simulink model "deltino"  (R2021b)
settings: Solver=VariableStepAuto  StartTime=0.0  StopTime=inf  FixedStep=0.0001  RelTol=1e-3
values from neighbouring files (symbols this model uses):
  alpha1 = 0    [compute_deltino_dyn_parallel.m]
  alpha2 = 2/3*pi    (= 2.09439510239)    [compute_deltino_dyn_parallel.m]
  alpha3 = 4/3*pi    (= 4.18879020479)    [compute_deltino_dyn_parallel.m]
  H = 0.05    [main.m]
  J_T = [J_1', J_2', J_3', J_4']    [main.m]
  K_d = 10    [main.m]
  K_el = 10000    [main.m]
  K_i = 1    [main.m]
  K_p = 200    [main.m]
  K_v = 10    [main.m]
  mu = 0.8    [main.m]
  ni_0 = zeros(18,1)    [main.m]
  offset1 = [l1/2; l2/2; -h/2]    [compute_deltino_dyn_parallel.m]    (also in main.m = [+l1/2; +l2/2; -h/2])
  offset2 = [l1/2; -l2/2; -h/2]    [compute_deltino_dyn_parallel.m]    (also in main.m = [+l1/2; -l2/2; -h/2])
  offset3 = [-l1/2; -l2/2; -h/2]    [compute_deltino_dyn_parallel.m]    (also in main.m)
  offset4 = [-l1/2; l2/2; -h/2]    [compute_deltino_dyn_parallel.m]    (also in main.m = [-l1/2; +l2/2; -h/2])
  p_leg1_0 = forward_kin(theta_leg1_0)    [main.m]
  p_leg2_0 = forward_kin(theta_leg2_0)    [main.m]
  p_leg3_0 = forward_kin(theta_leg3_0)    [main.m]
  p_leg4_0 = forward_kin(theta_leg4_0)    [main.m]
  points_ccw = [+0.1,  0.00 ... (first row only)    [main.m]
  points_cw = [-0.1,  0.00 ... (first row only)    [main.m]
  q_0 = [base_0; ypr_0; theta_leg1_0; ee_leg1_0; theta_leg2_0; ee_leg2_0;        theta_leg3_0; ee_leg3_0; theta_leg4_0; ee_leg4_0;]    [main.m]
  ratio = 2    [main.m]
  steps = 4+2*ratio    (= 8)    [main.m]
  theta_leg1_0 = [pi/6; pi/6; pi/6]    [main.m]
  theta_leg2_0 = [pi/6; pi/6; pi/6]    [main.m]
  theta_leg3_0 = [pi/6; pi/6; pi/6]    [main.m]
  theta_leg4_0 = [pi/6; pi/6; pi/6]    [main.m]
  ts = T/steps    (= 0.1875)    [main.m]
  ts2 = 3*ts    (= 0.5625)    [main.m]
  vel = 0.2    [main.m]
undefined symbols (not defined in the file or in its folder): l1, l_A, l_B, R, radius0, radius1, radius2, theta, WPs
libraries: simulink x14, dspsigops x12
(part 3 of 10)

== matlab function deltino/DELTINO DYNAMICS /compute_S_dot ==
  data: q input; S_dot output; q_dot input
function S_dot = S_dot(q, q_dot)
%#codegen

%    This function was generated by the Symbolic Math Toolbox version 9.0.
%    03-May-2022 13:43:05
bx = q(1); by = q(2); bz = q(3);
phi = q(4); zeta = q(5); psi = q(6);
th11 = q(7); th12 = q(8); th13 = q(9);
p1x = q(10); p1y = q(11); p1z = q(12);
th21 = q(13); th22 = q(14); th23 = q(15);
p2x = q(16); p2y = q(17); p2z = q(18);
th31 = q(19); th32 = q(20); th33 = q(21);
p3x = q(22); p3y = q(23); p3z = q(24);
th41 = q(25); th42 = q(26); th43 = q(27);
p4x = q(28); p4y = q(29); p4z = q(30);

bx_dot = q_dot(1); by_dot = q_dot(2); bz_dot = q(3);
phi_dot = q_dot(4); zeta_dot = q_dot(5); psi_dot = q(6);
th11_dot = q_dot(7); th12_dot = q_dot(8); th13_dot = q_dot(9);
p1x_dot = q_dot(10); p1y_dot = q_dot(11); p1z_dot = q_dot(12);
th21_dot = q_dot(13); th22_dot = q_dot(14); th23_dot = q_dot(15);
p2x_dot = q_dot(16); p2y_dot = q_dot(17); p2z_dot = q_dot(18);
th31_dot = q_dot(19); th32_dot = q_dot(20); th33_dot = q_dot(21);
p3x_dot = q_dot(22); p3y_dot = q_dot(23); p3z_dot = q_dot(24);
th41_dot = q_dot(25); th42_dot = q_dot(26); th43_dot = q_dot(27);
p4x_dot = q_dot(28); p4y_dot = q_dot(29); p4z_dot = q_dot(30);

t2 = cos(phi);
t3 = cos(psi);
t4 = cos(th11);
t5 = cos(th12);
t6 = cos(th13);
t7 = cos(th21);
t8 = cos(th22);
t9 = cos(th23);
t10 = cos(th31);
t11 = cos(th32);
t12 = cos(th33);
t13 = cos(th41);
t14 = cos(th42);
t15 = cos(th43);
t16 = cos(zeta);
t17 = sin(phi);
t18 = sin(psi);
t19 = sin(th11);
t20 = sin(th12);
t21 = sin(th13);
t22 = sin(th21);
t23 = sin(th22);
t24 = sin(th23);
t25 = sin(th31);
t26 = sin(th32);
t27 = sin(th33);
t28 = sin(th41);
t29 = sin(th42);
t30 = sin(th43);
t31 = sin(zeta);
t45 = -bx;
t46 = bx.*2.0e+1;
t47 = -bx_dot;
t48 = -by;
t49 = by.*2.0e+1;
t50 = -by_dot;
t51 = -bz;
t52 = bz.*2.0e+1;
t53 = p1x.*2.0e+1;
t54 = p2x.*2.0e+1;
t55 = p3x.*2.0e+1;
t56 = p4x.*2.0e+1;
t57 = -p1y;
t58 = -p2y;
t59 = -p4y;
t60 = p1y.*2.0e+1;
t61 = p2y.*2.0e+1;
t62 = p3y.*2.0e+1;
t63 = p4y.*2.0e+1;
t64 = -p3x_dot;
t65 = -p4x_dot;
t66 = -p4z;
t67 = p1z.*2.0e+1;
t68 = p2z.*2.0e+1;
t69 = p3z.*2.0e+1;
t70 = p4z.*2.0e+1;
t71 = -p1y_dot;
t72 = -p4y_dot;
t73 = -p1z_dot;
t74 = -p2z_dot;
t75 = -p3z_dot;
t76 = -p4z_dot;
t102 = sqrt(3.0);
t32 = t3.*7.0;
t33 = t5.*2.0;
t34 = t6.*2.0;
t35 = t8.*2.0;
t36 = t9.*2.0;
t37 = t11.*2.0;
t38 = t12.*2.0;
t39 = t14.*2.0;
t40 = t15.*2.0;
t41 = t18.*2.0;
t42 = t31.*5.0;
t43 = t31.*6.0;
t44 = t31.*7.0;
t77 = t2.*t3;
t78 = t2.*t16;
t79 = t2.*t18;
t80 = t3.*t17;
t81 = t16.*t17;
t82 = t17.*t18;
t84 = t19.*t31;
t85 = t20.*t31;
t86 = t21.*t31;
t87 = t22.*t31;
t88 = t23.*t31;
t89 = t24.*t31;
t90 = t25.*t31;
t91 = t26.*t31;
t92 = t27.*t31;
t93 = t28.*t31;
t94 = t29.*t31;
t95 = t30.*t31;
t100 = t31.*8.0;
t101 = t31.*9.0;
t103 = -t46;
t104 = -t49;
t105 = -t52;
t106 = -t60;
t107 = -t61;
t108 = -t63;
t109 = -t70;
t113 = t3.*t16.*2.0;
t118 = t16.*t18.*7.0;
t120 = t4.*t31.*4.0;
t123 = t7.*t31.*4.0;
t126 = t10.*t31.*4.0;
t129 = t13.*t31.*4.0;
t132 = t18.*t19.*4.0;
t133 = t18.*t20.*4.0;
t134 = t18.*t21.*4.0;
t135 = t18.*t22.*4.0;
t136 = t18.*t23.*4.0;
t137 = t18.*t24.*4.0;
t138 = t18.*t25.*4.0;
t139 = t18.*t26.*4.0;
t140 = t18.*t27.*4.0;
t141 = t18.*t28.*4.0;
t142 = t18.*t29.*4.0;
t143 = t18.*t30.*4.0;
t144 = t4./5.0;
t145 = t5./5.0;
t146 = t6./5.0;
t147 = t7./5.0;
t148 = t8./5.0;
t149 = t9./5.0;
t150 = t10./5.0;
t151 = t11./5.0;
t152 = t12./5.0;
t153 = t13./5.0;
t154 = t14./5.0;
t155 = t15./5.0;
t156 = t16./2.0;
t157 = t16./4.0;
t158 = t31./2.0;
t159 = t31./4.0;
t195 = t6.*t31.*-2.0;
t196 = t8.*t31.*-2.0;
t197 = t9.*t31.*-2.0;
t198 = t12.*t31.*-2.0;
t199 = t15.*t31.*-2.0;
t202 = t16.*(7.0./2.0e+1);
t204 = t31.*(7.0./2.0e+1);
t209 = t3.*t4.*t16;
t210 = t3.*t7.*t16;
t211 = t3.*t10.*t16;
t212 = t3.*t13.*t16;
t251 = t16.*(9.0./2.0e+1);
t253 = t31.*(9.0./2.0e+1);
t270 = t3.*t102;
t272 = t31.*zeta_dot.*(-1.0./2.0);
t291 = t3.*t16.*t19.*4.0;
t292 = t3.*t16.*t20.*4.0;
t293 = t3.*t16.*t21.*4.0;
t294 = t3.*t16.*t22.*4.0;
t295 = t3.*t16.*t23.*4.0;
t296 = t3.*t16.*t24.*4.0;
t297 = t3.*t16.*t25.*4.0;
t298 = t3.*t16.*t26.*4.0;
t299 = t3.*t16.*t27.*4.0;
t300 = t3.*t16.*t28.*4.0;
t301 = t3.*t16.*t29.*4.0;
t302 = t3.*t16.*t30.*4.0;
t314 = (t3.*t16)./1.0e+1;
t316 = t7.*t16.*(-1.0./5.0);
t317 = t10.*t16.*(-1.0./5.0);
t318 = t13.*t16.*(-1.0./5.0);
t326 = (t3.*t31)./1.0e+1;
t360 = (t16.*t19.*zeta_dot)./5.0;
t361 = (t16.*t22.*zeta_dot)./5.0;
t362 = (t16.*t25.*zeta_dot)./5.0;
t363 = (t16.*t28.*zeta_dot)./5.0;
t372 = t16.*zeta_dot.*(-7.0./2.0e+1);
t374 = t31.*zeta_dot.*(-7.0./2.0e+1);
t433 = t16.*t18.*(-7.0./2.0e+1);
t435 = t18.*t31.*(-7.0./2.0e+1);
t447 = t16.*t18.*t102;
t466 = t4.*t16.*zeta_dot.*(-1.0./5.0);
t473 = (psi_dot.*t16.*t18)./1.0e+1;
t481 = t2.*t31.*zeta_dot.*(-1.0./4.0);
t487 = phi_dot.*t17.*t31.*(-1.0./2.0);
t488 = phi_dot.*t17.*t31.*(-1.0./4.0);
t490 = (psi_dot.*t18.*t31)./1.0e+1;
t492 = t17.*t31.*zeta_dot.*(-1.0./4.0);
t494 = (t18.*t31.*zeta_dot)./1.0e+1;
t496 = t16.*zeta_dot.*(-9.0./2.0e+1);
t537 = (t3.*t16.*t19)./5.0;
t538 = (t3.*t16.*t20)./5.0;
t539 = (t3.*t16.*t21)./5.0;
t540 = (t3.*t16.*t22)./5.0;
t541 = (t3.*t16.*t23)./5.0;
t542 = (t3.*t16.*t24)./5.0;
t543 = (t3.*t16.*t25)./5.0;
t544 = (t3.*t16.*t26)./5.0;
t545 = (t3.*t16.*t27)./5.0;
t546 = (t3.*t16.*t28)./5.0;
t547 = (t3.*t16.*t29)./5.0;
t548 = (t3.*t16.*t30)./5.0;
t706 = (psi_dot.*t16.*t18.*t19)./5.0;
t707 = (psi_dot.*t16.*t18.*t20)./5.0;
t708 = (psi_dot.*t16.*t18.*t21)./5.0;
t709 = (psi_dot.*t16.*t18.*t22)./5.0;
t710 = (psi_dot.*t16.*t18.*t23)./5.0;
t711 = (psi_dot.*t16.*t18.*t24)./5.0;
t712 = (psi_dot.*t16.*t18.*t25)./5.0;
t713 = (psi_dot.*t16.*t18.*t26)./5.0;
t714 = (psi_dot.*t16.*t18.*t27)./5.0;
t715 = (psi_dot.*t16.*t18.*t28)./5.0;
t716 = (psi_dot.*t16.*t18.*t29)./5.0;
t717 = (psi_dot.*t16.*t18.*t30)./5.0;
t728 = psi_dot.*t3.*t16.*(-1.0./1.0e+1);
t729 = psi_dot.*t3.*t16.*(-7.0./2.0e+1);
t765 = t3.*t16.*zeta_dot.*(-1.0./1.0e+1);
t766 = phi_dot.*t2.*t31.*(-7.0./2.0e+1);
t770 = psi_dot.*t3.*t31.*(-7.0./2.0e+1);
t797 = phi_dot.*t17.*t31.*(-7.0./2.0e+1);
t857 = t3.*t5.*t16.*th12_dot.*(-1.0./5.0);
t858 = t3.*t6.*t16.*th13_dot.*(-1.0./5.0);
t860 = t3.*t8.*t16.*th22_dot.*(-1.0./5.0);
t861 = t3.*t9.*t16.*th23_dot.*(-1.0./5.0);
t863 = t3.*t11.*t16.*th32_dot.*(-1.0./5.0);
t864 = t3.*t12.*t16.*th33_dot.*(-1.0./5.0);
t866 = t3.*t14.*t16.*th42_dot.*(-1.0./5.0);
t867 = t3.*t15.*t16.*th43_dot.*(-1.0./5.0);
t1132 = t18.*t31.*t102.*(-1.0./2.0);
t83 = -t32;
t96 = -t41;
t97 = -t42;
t98 = -t43;
t99 = -t44;
t110 = t2.*t32;
t111 = t78.*5.0;
t112 = t78.*7.0;
t114 = t2.*t41;
t115 = t17.*t32;
t116 = t81.*5.0;
t117 = t81.*7.0;
t119 = t31.*t33;
t121 = t31.*t34;
t122 = t31.*t35;
t124 = t31.*t36;
t125 = t31.*t37;
t127 = t31.*t38;
t128 = t31.*t39;
t130 = t31.*t40;
t131 = t17.*t41;
t160 = -t100;
t161 = phi_dot.*t77;
t162 = psi_dot.*t77;
t163 = phi_dot.*t79;
t164 = phi_dot.*t80;
t165 = psi_dot.*t79;
t166 = psi_dot.*t80;
t167 = t33+1.0;
t168 = t34+1.0;
t169 = t35+1.0;
t170 = t36+1.0;
t171 = t37+1.0;
t172 = t38+1.0;
t173 = t39+1.0;
t174 = t40+1.0;
t175 = phi_dot.*t82;
t176 = psi_dot.*t82;
t177 = t31.*t79;
t178 = t31.*t80;
t179 = t77.*-7.0;
t180 = t19.*t81;
t181 = t22.*t81;
t182 = t25.*t81;
t183 = t28.*t81;
t185 = t78.*9.0;
t186 = -t113;
t187 = t31.*t82;
t188 = t79.*-2.0;
t189 = t80.*-7.0;
t190 = -t81;
t193 = t81.*9.0;
t194 = -t118;
t200 = -t137;
t201 = -t140;
t203 = -t159;
t205 = t156.*zeta_dot;
t206 = t157.*zeta_dot;
t207 = t158.*zeta_dot;
t208 = t159.*zeta_dot;
t213 = t4.*t79;
t214 = t7.*t79;
t215 = t10.*t79;
t216 = t13.*t79;
t217 = t31.*t77;
t218 = t19.*t78;
t219 = t22.*t78;
t220 = t25.*t78;
t221 = t28.*t78;
t222 = t4.*t82;
t223 = t7.*t82;
t224 = t10.*t82;
t225 = t13.*t82;
t227 = t44.*t79;
t228 = t19.*t82.*4.0;
t229 = t22.*t82.*4.0;
t230 = t25.*t82.*4.0;
t231 = t28.*t82.*4.0;
t232 = t78./2.0;
t233 = t78./4.0;
t235 = t44.*t82;
t236 = t16.*t144;
t237 = t16.*t147;
t238 = t16.*t150;
t239 = t16.*t153;
t240 = t81./2.0;
t241 = t81./4.0;
t242 = t31.*t144;
t243 = t31.*t147;
t244 = t31.*t150;
t245 = t31.*t153;
t246 = t84./5.0;
t247 = t87./5.0;
t248 = t90./5.0;
t249 = t93./5.0;
t250 = -t202;
t252 = -t204;
t254 = t16.*t77.*zeta_dot;
t257 = t18.*t78.*zeta_dot;
t258 = t16.*t80.*zeta_dot;
t265 = t18.*t81.*zeta_dot;
t271 = t202.*zeta_dot;
t273 = t204.*zeta_dot;
t274 = t4.*t78.*4.0;
t275 = t7.*t78.*4.0;
t276 = t10.*t78.*4.0;
t277 = t13.*t78.*4.0;
t278 = t3.*t16.*t33;
t279 = t3.*t16.*t34;
t280 = t3.*t16.*t35;
t281 = t3.*t16.*t36;
t282 = t3.*t16.*t37;
t283 = t3.*t16.*t38;
t284 = t3.*t16.*t39;
t285 = t3.*t16.*t40;
t287 = t4.*t81.*4.0;
t288 = t7.*t81.*4.0;
t289 = t10.*t81.*4.0;
t290 = t13.*t81.*4.0;
t303 = t19.*t79.*4.0;
t304 = t22.*t79.*4.0;
t305 = t25.*t79.*4.0;
t306 = t28.*t79.*4.0;
t311 = t77./1.0e+1;
t312 = t77.*(7.0./2.0e+1);
t313 = t78.*(7.0./2.0e+1);
t319 = t79./1.0e+1;
t320 = t80./1.0e+1;
t321 = t79.*(7.0./2.0e+1);
t322 = t80.*(7.0./2.0e+1);
t325 = t81.*(7.0./2.0e+1);
t327 = t18.*t202;
t328 = t82./1.0e+1;
t329 = t82.*(7.0./2.0e+1);
t330 = t18.*t204;
t331 = t85./1.0e+1;
t332 = t86./1.0e+1;
t333 = t88./1.0e+1;
t334 = t89./1.0e+1;
t335 = t91./1.0e+1;
t336 = t92./1.0e+1;
t337 = t94./1.0e+1;
t338 = t95./1.0e+1;
t339 = -t251;
t348 = phi_dot.*t2.*t158;
t350 = phi_dot.*t2.*t159;
t364 = phi_dot.*t17.*t158;
t365 = phi_dot.*t17.*t159;
t373 = t251.*zeta_dot;
t375 = t253.*zeta_dot;
t388 = -t209;
t389 = -t210;
t390 = -t211;
t391 = -t212;
t397 = -t292;
t398 = -t298;
t399 = -t301;
t400 = -t302;
t408 = (t3.*t85)./5.0;
t409 = (t3.*t86)./5.0;
t411 = (t3.*t88)./5.0;
t412 = (t3.*t89)./5.0;
t414 = (t3.*t91)./5.0;
t415 = (t3.*t92)./5.0;
t417 = (t3.*t94)./5.0;
t418 = (t3.*t95)./5.0;
t419 = (t19.*t82)./5.0;
t420 = (t22.*t82)./5.0;
t421 = (t25.*t82)./5.0;
t422 = (t28.*t82)./5.0;
t424 = t78.*(9.0./2.0e+1);
t425 = -t314;
t431 = t81.*(9.0./2.0e+1);
t432 = -t326;
t436 = t77.*t102;
t440 = t80.*t102;
t448 = phi_dot.*t78.*(-1.0./2.0);
t450 = psi_dot.*t314;
t451 = psi_dot.*t3.*t202;
t463 = t78.*zeta_dot.*(-1.0./2.0);
t465 = t314.*zeta_dot;
t467 = t316.*zeta_dot;
t468 = t317.*zeta_dot;
t469 = t318.*zeta_dot;
t470 = phi_dot.*t81.*(-1.0./4.0);
t471 = phi_dot.*t2.*t204;
t474 = psi_dot.*t3.*t204;
t476 = -t270;
t484 = t326.*zeta_dot;
t489 = phi_dot.*t17.*t204;
t491 = t17.*t272;
t497 = t77.*t84.*4.0;
t498 = t77.*t87.*4.0;
t499 = t77.*t90.*4.0;
t500 = t77.*t93.*4.0;
t501 = t78.*t144;
t502 = t78.*t147;
t503 = t78.*t150;
t504 = t78.*t153;
t506 = t3.*t16.*t145;
t507 = t3.*t16.*t146;
t509 = t3.*t16.*t148;
t510 = t3.*t16.*t149;
t512 = t3.*t16.*t151;
t513 = t3.*t16.*t152;
t515 = t3.*t16.*t154;
t516 = t3.*t16.*t155;
t517 = t80.*t84.*4.0;
t518 = t80.*t87.*4.0;
t519 = t80.*t90.*4.0;
t520 = t80.*t93.*4.0;
t521 = (t19.*t77)./5.0;
t522 = t79.*t144;
t523 = (t22.*t77)./5.0;
t524 = t79.*t147;
t525 = (t25.*t77)./5.0;
t526 = t79.*t150;
t527 = (t28.*t77)./5.0;
t528 = t79.*t153;
t530 = t81.*t144;
t532 = t81.*t147;
t534 = t81.*t150;
t536 = t81.*t153;
t549 = (t19.*t79)./5.0;
t550 = (t19.*t80)./5.0;
t551 = t82.*t144;
t552 = (t22.*t79)./5.0;
t553 = (t22.*t80)./5.0;
t554 = t82.*t147;
t555 = (t25.*t79)./5.0;
t556 = (t25.*t80)./5.0;
t557 = t82.*t150;
t558 = (t28.*t79)./5.0;
t559 = (t28.*t80)./5.0;
t560 = t82.*t153;
t569 = t3.*t84.*(-1.0./5.0);
t622 = psi_dot.*t16.*t18.*t145;
t623 = psi_dot.*t16.*t18.*t146;
t625 = psi_dot.*t16.*t18.*t148;
t626 = psi_dot.*t16.*t18.*t149;
t628 = psi_dot.*t16.*t18.*t151;
t629 = psi_dot.*t16.*t18.*t152;
t631 = psi_dot.*t16.*t18.*t154;
t632 = psi_dot.*t16.*t18.*t155;
t633 = t33.*t270;
t634 = t34.*t270;
t635 = t35.*t270;
t636 = t36.*t270;
t637 = t37.*t270;
t638 = t38.*t270;
t639 = t39.*t270;
t640 = t40.*t270;
t649 = t537.*th11_dot;
t650 = t538.*th12_dot;
t651 = t539.*th13_dot;
t652 = t540.*th21_dot;
t653 = t541.*th22_dot;
t654 = t542.*th23_dot;
t655 = t543.*th31_dot;
t656 = t544.*th32_dot;
t657 = t545.*th33_dot;
t658 = t546.*th41_dot;
t659 = t547.*th42_dot;
t660 = t548.*th43_dot;
t686 = t3.*t31.*t145.*zeta_dot;
t687 = t3.*t31.*t146.*zeta_dot;
t689 = t3.*t31.*t148.*zeta_dot;
t690 = t3.*t31.*t149.*zeta_dot;
t692 = t3.*t31.*t151.*zeta_dot;
t693 = t3.*t31.*t152.*zeta_dot;
t695 = t3.*t31.*t154.*zeta_dot;
t696 = t3.*t31.*t155.*zeta_dot;
t726 = phi_dot.*t78.*(-7.0./2.0e+1);
t763 = t78.*zeta_dot.*(-7.0./2.0e+1);
S_dot = ft_1({bx,bx_dot,by,by_dot,bz,bz_dot,p1x,p1x_dot,p1y,p1y_dot,p1z,p2x,p2x_dot,p2y,p2y_dot,p2z,p3x,p3x_dot,p3y,p3y_dot,p3z,p4x,p4x_dot,p4y,p4y_dot,p4z,phi_dot,psi_dot,t10,t100,t101,t102,t103,t104,t105,t106,t107,t108,t109,t11,t110,t111,t112,t113,t1132,t114,t115,t116,t117,t118,t119,t12,t120,t123,t125,t126,t128,t129,t13,t131,t132,t133,t134,t135,t136,t138,t139,t14,t141,t142,t143,t144,t145,t146,t147,t148,t149,t15,t150,t151,t152,t153,t154,t155,t156,t157,t158,t16,t160,t161,t162,t163,t164,t165,t166,t167,t168,t169,t17,t170,t171,t172,t173,t174,t175,t176,t177,t178,t179,t18,t180,t181,t182,t183,t185,t186,t187,t188,t189,t19,t190,t193,t194,t195,t196,t197,t198,t199,t2,t20,t200,t201,t202,t203,t204,t205,t206,t207,t208,t209,t21,t210,t211,t212,t213,t214,t215,t216,t217,t218,t219,t22,t220,t221,t222,t223,t224,t225,t227,t228,t229,t23,t230,t231,t232,t233,t235,t236,t237,t238,t239,t24,t240,t241,t242,t243,t244,t245,t246,t247,t248,t249,t25,t250,t251,t252,t253,t254,t257,t258,t26,t265,t27,t270,t271,t272,t273,t274,t275,t276,t277,t278,t279,t28,t280,t281,t282,t283,t284,t285,t287,t288,t289,t29,t290,t291,t292,t293,t294,t295,t296,t297,t298,t299,t3,t30,t300,t302,t303,t304,t305,t306,t31,t311,t312,t313,t314,t316,t317,t318,t319,t32,t320,t321,t322,t325,t326,t327,t328,t329,t33,t330,t331,t332,t333,t334,t335,t336,t337,t338,t339,t34,t348,t35,t350,t36,t360,t361,t362,t363,t364,t37,t372,t374,t375,t38,t388,t389,t39,t390,t391,t397,t398,t399,t4,t40,t400,t408,t409,t41,t411,t412,t414,t415,t417,t418,t419,t420,t421,t422,t424,t425,t43,t431,t432,t433,t435,t436,t44,t440,t447,t448,t45,t450,t451,t463,t465,t466,t467,t468,t469,t47,t470,t471,t473,t474,t476,t48,t481,t484,t487,t488,t489,t49,t490,t491,t492,t494,t496,t497,t498,t499,t5,t50,t500,t501,t502,t503,t504,t506,t507,t509,t51,t510,t512,t513,t515,t516,t517,t518,t519,t52,t520,t521,t522,t523,t524,t525,t526,t527,t528,t53,t530,t532,t534,t536,t537,t538,t539,t54,t540,t541,t542,t543,t544,t545,t546,t547,t548,t549,t55,t550,t551,t552,t553,t554,t555,t556,t557,t558,t559,t56,t560,t569,t57,t58,t59,t6,t61,t62,t622,t623,t625,t626,t628,t629,t631,t632,t633,t635,t636,t637,t638,t639,t64,t649,t65,t650,t651,t652,t653,t654,t655,t656,t657,t658,t659,t66,t660,t67,t68,t686,t687,t689,t69,t690,t692,t693,t695,t696,t7,t70,t706,t707,t708,t709,t71,t710,t711,t712,t713,t714,t715,t716,t717,t72,t726,t728,t729,t73,t74,t75,t76,t763,t765,t77,t770,t78,t79,t797,t8,t80,t81,t82,t83,t84,t85,t857,t858,t86,t860,t861,t863,t864,t866,t867,t87,t88,t89,t9,t90,t91,t92,t93,t94,t95,t96,t97,t98,t99,th11_dot,th12_dot,th13_dot,th21_dot,th22_dot,th23_dot,th31_dot,th32_dot,th33_dot,th41_dot,th42_dot,th43_dot,zeta_dot});
end
function S_dot = ft_1(ct)
bx = ct{1};
bx_dot = ct{2};
by = ct{3};
by_dot = ct{4};
bz = ct{5};
bz_dot = ct{6};
p1x = ct{7};
p1x_dot = ct{8};
p1y = ct{9};
p1y_dot = ct{10};
p1z = ct{11};
p2x = ct{12};
p2x_dot = ct{13};
p2y = ct{14};
p2y_dot = ct{15};
p2z = ct{16};
p3x = ct{17};
p3x_dot = ct{18};
p3y = ct{19};
p3y_dot = ct{20};
p3z = ct{21};
p4x = ct{22};
p4x_dot = ct{23};
p4y = ct{24};
p4y_dot = ct{25};
p4z = ct{26};
phi_dot = ct{27};
psi_dot = ct{28};
t10 = ct{29};
t100 = ct{30};
t101 = ct{31};
t102 = ct{32};
t103 = ct{33};
t104 = ct{34};
t105 = ct{35};
t106 = ct{36};
t107 = ct{37};
t108 = ct{38};
t109 = ct{39};
t11 = ct{40};
t110 = ct{41};
t111 = ct{42};
t112 = ct{43};
t113 = ct{44};
t1132 = ct{45};
t114 = ct{46};
t115 = ct{47};
t116 = ct{48};
t117 = ct{49};
t118 = ct{50};
t119 = ct{51};
t12 = ct{52};
t120 = ct{53};
t123 = ct{54};
t125 = ct{55};
t126 = ct{56};
t128 = ct{57};
t129 = ct{58};
t13 = ct{59};
t131 = ct{60};
t132 = ct{61};
t133 = ct{62};
t134 = ct{63};
t135 = ct{64};
t136 = ct{65};
t138 = ct{66};
t139 = ct{67};
t14 = ct{68};
t141 = ct{69};
t142 = ct{70};
t143 = ct{71};
t144 = ct{72};
t145 = ct{73};
t146 = ct{74};
t147 = ct{75};
t148 = ct{76};
t149 = ct{77};
t15 = ct{78};
t150 = ct{79};
t151 = ct{80};
t152 = ct{81};
t153 = ct{82};
t154 = ct{83};
t155 = ct{84};
t156 = ct{85};
t157 = ct{86};
t158 = ct{87};
t16 = ct{88};
t160 = ct{89};
t161 = ct{90};
t162 = ct{91};
t163 = ct{92};
t164 = ct{93};
t165 = ct{94};
t166 = ct{95};
t167 = ct{96};
t168 = ct{97};
t169 = ct{98};
t17 = ct{99};
t170 = ct{100};
t171 = ct{101};
t172 = ct{102};
t173 = ct{103};
t174 = ct{104};
t175 = ct{105};
t176 = ct{106};
t177 = ct{107};
t178 = ct{108};
t179 = ct{109};
t18 = ct{110};
t180 = ct{111};
t181 = ct{112};
t182 = ct{113};
t183 = ct{114};
t185 = ct{115};
t186 = ct{116};
t187 = ct{117};
t188 = ct{118};
t189 = ct{119};
t19 = ct{120};
t190 = ct{121};
t193 = ct{122};
t194 = ct{123};
t195 = ct{124};
t196 = ct{125};
t197 = ct{126};
t198 = ct{127};
t199 = ct{128};
t2 = ct{129};
t20 = ct{130};
t200 = ct{131};
t201 = ct{132};
t202 = ct{133};
t203 = ct{134};
t204 = ct{135};
t205 = ct{136};
t206 = ct{137};
t207 = ct{138};
t208 = ct{139};
t209 = ct{140};
t21 = ct{141};
t210 = ct{142};
t211 = ct{143};
t212 = ct{144};
t213 = ct{145};
t214 = ct{146};
t215 = ct{147};
t216 = ct{148};
t217 = ct{149};
t218 = ct{150};
t219 = ct{151};
t22 = ct{152};
t220 = ct{153};
t221 = ct{154};
t222 = ct{155};
t223 = ct{156};
t224 = ct{157};
t225 = ct{158};
t227 = ct{159};
t228 = ct{160};
t229 = ct{161};
t23 = ct{162};
t230 = ct{163};
t231 = ct{164};
t232 = ct{165};
t233 = ct{166};
t235 = ct{167};
t236 = ct{168};
t237 = ct{169};
t238 = ct{170};
t239 = ct{171};
t24 = ct{172};
t240 = ct{173};
t241 = ct{174};
t242 = ct{175};
t243 = ct{176};
t244 = ct{177};
t245 = ct{178};
t246 = ct{179};
t247 = ct{180};
t248 = ct{181};
t249 = ct{182};
t25 = ct{183};
t250 = ct{184};
t251 = ct{185};
t252 = ct{186};
t253 = ct{187};
t254 = ct{188};
t257 = ct{189};
t258 = ct{190};
t26 = ct{191};
t265 = ct{192};
t27 = ct{193};
t270 = ct{194};
t271 = ct{195};
t272 = ct{196};
t273 = ct{197};
t274 = ct{198};
t275 = ct{199};
t276 = ct{200};
t277 = ct{201};
t278 = ct{202};
t279 = ct{203};
t28 = ct{204};
t280 = ct{205};
t281 = ct{206};
t282 = ct{207};
t283 = ct{208};
t284 = ct{209};
t285 = ct{210};
t287 = ct{211};
t288 = ct{212};
t289 = ct{213};
t29 = ct{214};
t290 = ct{215};
t291 = ct{216};
t292 = ct{217};
t293 = ct{218};
t294 = ct{219};
t295 = ct{220};
t296 = ct{221};
t297 = ct{222};
t298 = ct{223};
t299 = ct{224};
t3 = ct{225};
t30 = ct{226};
t300 = ct{227};
t302 = ct{228};
t303 = ct{229};
t304 = ct{230};
t305 = ct{231};
t306 = ct{232};
t31 = ct{233};
t311 = ct{234};
t312 = ct{235};
t313 = ct{236};
t314 = ct{237};
t316 = ct{238};
t317 = ct{239};
t318 = ct{240};
t319 = ct{241};
t32 = ct{242};
t320 = ct{243};
t321 = ct{244};
t322 = ct{245};
t325 = ct{246};
t326 = ct{247};
t327 = ct{248};
t328 = ct{249};
t329 = ct{250};
t33 = ct{251};
t330 = ct{252};
t331 = ct{253};
t332 = ct{254};
t333 = ct{255};
t334 = ct{256};
t335 = ct{257};
t336 = ct{258};
t337 = ct{259};
t338 = ct{260};
t339 = ct{261};
t34 = ct{262};
t348 = ct{263};
t35 = ct{264};
t350 = ct{265};
t36 = ct{266};
t360 = ct{267};
t361 = ct{268};
t362 = ct{269};
t363 = ct{270};
t364 = ct{271};
t37 = ct{272};
t372 = ct{273};
t374 = ct{274};
t375 = ct{275};
t38 = ct{276};
t388 = ct{277};
t389 = ct{278};
t39 = ct{279};
t390 = ct{280};
t391 = ct{281};
t397 = ct{282};
t398 = ct{283};
t399 = ct{284};
t4 = ct{285};
t40 = ct{286};
t400 = ct{287};
t408 = ct{288};
t409 = ct{289};
t41 = ct{290};
t411 = ct{291};
t412 = ct{292};
t414 = ct{293};
t415 = ct{294};
t417 = ct{295};
t418 = ct{296};
t419 = ct{297};
t420 = ct{298};
t421 = ct{299};
t422 = ct{300};
t424 = ct{301};
t425 = ct{302};
t43 = ct{303};
t431 = ct{304};
t432 = ct{305};
t433 = ct{306};
t435 = ct{307};
t436 = ct{308};
t44 = ct{309};
t440 = ct{310};
t447 = ct{311};
t448 = ct{312};
t45 = ct{313};
t450 = ct{314};
t451 = ct{315};
t463 = ct{316};
t465 = ct{317};
t466 = ct{318};
t467 = ct{319};
t468 = ct{320};
t469 = ct{321};
t47 = ct{322};
t470 = ct{323};
t471 = ct{324};
t473 = ct{325};
t474 = ct{326};
t476 = ct{327};
t48 = ct{328};
t481 = ct{329};
t484 = ct{330};
t487 = ct{331};
t488 = ct{332};
t489 = ct{333};
t49 = ct{334};
t490 = ct{335};
t491 = ct{336};
t492 = ct{337};
t494 = ct{338};
t496 = ct{339};
t497 = ct{340};
t498 = ct{341};
t499 = ct{342};
t5 = ct{343};
t50 = ct{344};
t500 = ct{345};
t501 = ct{346};
t502 = ct{347};
t503 = ct{348};
t504 = ct{349};
t506 = ct{350};
t507 = ct{351};
t509 = ct{352};
t51 = ct{353};
t510 = ct{354};
t512 = ct{355};
t513 = ct{356};
t515 = ct{357};
t516 = ct{358};
t517 = ct{359};
t518 = ct{360};
t519 = ct{361};
t52 = ct{362};
t520 = ct{363};
t521 = ct{364};
t522 = ct{365};
t523 = ct{366};
t524 = ct{367};
t525 = ct{368};
t526 = ct{369};
t527 = ct{370};
t528 = ct{371};
t53 = ct{372};
t530 = ct{373};
t532 = ct{374};
t534 = ct{375};
t536 = ct{376};
t537 = ct{377};
t538 = ct{378};
t539 = ct{379};
t54 = ct{380};
t540 = ct{381};
t541 = ct{382};
t542 = ct{383};
t543 = ct{384};
t544 = ct{385};
t545 = ct{386};
t546 = ct{387};
t547 = ct{388};
t548 = ct{389};
t549 = ct{390};
t55 = ct{391};
t550 = ct{392};
t551 = ct{393};
t552 = ct{394};
t553 = ct{395};
t554 = ct{396};
t555 = ct{397};
t556 = ct{398};
t557 = ct{399};
t558 = ct{400};
t559 = ct{401};
t56 = ct{402};
t560 = ct{403};
t569 = ct{404};
t57 = ct{405};
t58 = ct{406};
t59 = ct{407};
t6 = ct{408};
t61 = ct{409};
t62 = ct{410};
t622 = ct{411};
t623 = ct{412};
t625 = ct{413};
t626 = ct{414};
t628 = ct{415};
t629 = ct{416};
t631 = ct{417};
t632 = ct{418};
t633 = ct{419};
t635 = ct{420};
t636 = ct{421};
t637 = ct{422};
t638 = ct{423};
t639 = ct{424};
t64 = ct{425};
t649 = ct{426};
t65 = ct{427};
t650 = ct{428};
t651 = ct{429};
t652 = ct{430};
t653 = ct{431};
t654 = ct{432};
t655 = ct{433};
t656 = ct{434};
t657 = ct{435};
t658 = ct{436};
t659 = ct{437};
t66 = ct{438};
t660 = ct{439};
t67 = ct{440};
t68 = ct{441};
t686 = ct{442};
t687 = ct{443};
t689 = ct{444};
t69 = ct{445};
t690 = ct{446};
t692 = ct{447};
t693 = ct{448};
t695 = ct{449};
t696 = ct{450};
t7 = ct{451};
t70 = ct{452};
t706 = ct{453};
t707 = ct{454};
t708 = ct{455};
t709 = ct{456};
t71 = ct{457};
t710 = ct{458};
t711 = ct{459};
t712 = ct{460};
t713 = ct{461};
t714 = ct{462};
t715 = ct{463};
t716 = ct{464};
t717 = ct{465};
t72 = ct{466};
t726 = ct{467};
t728 = ct{468};
t729 = ct{469};
t73 = ct{470};
t74 = ct{471};
t75 = ct{472};
t76 = ct{473};
t763 = ct{474};
t765 = ct{475};
t77 = ct{476};
t770 = ct{477};
t78 = ct{478};
t79 = ct{479};
t797 = ct{480};
t8 = ct{481};
t80 = ct{482};
t81 = ct{483};
t82 = ct{484};
t83 = ct{485};
t84 = ct{486};
t85 = ct{487};
t857 = ct{488};
t858 = ct{489};
t86 = ct{490};
t860 = ct{491};
t861 = ct{492};
t863 = ct{493};
t864 = ct{494};
t866 = ct{495};
t867 = ct{496};
t87 = ct{497};
t88 = ct{498};
t89 = ct{499};
t9 = ct{500};
t90 = ct{501};
t91 = ct{502};
t92 = ct{503};
t93 = ct{504};
t94 = ct{505};
t95 = ct{506};
t96 = ct{507};
t97 = ct{508};
t98 = ct{509};
t99 = ct{510};
th11_dot = ct{511};
th12_dot = ct{512};
th13_dot = ct{513};
th21_dot = ct{514};
th22_dot = ct{515};
th23_dot = ct{516};
th31_dot = ct{517};
th32_dot = ct{518};
th33_dot = ct{519};
th41_dot = ct{520};
th42_dot = ct{521};
th43_dot = ct{522};
zeta_dot = ct{523};
t767 = phi_dot.*t81.*(-7.0./2.0e+1);
t768 = phi_dot.*t2.*t253;
t771 = psi_dot.*t433;
t776 = t144+1.0./1.0e+1;
t777 = t145+1.0./1.0e+1;
t778 = t146+1.0./1.0e+1;
t779 = t147+1.0./1.0e+1;
t780 = t148+1.0./1.0e+1;
t781 = t149+1.0./1.0e+1;
t782 = t150+1.0./1.0e+1;
t783 = t151+1.0./1.0e+1;
t784 = t152+1.0./1.0e+1;
t785 = t153+1.0./1.0e+1;
t786 = t154+1.0./1.0e+1;
t787 = t155+1.0./1.0e+1;
t791 = t2.*t374;
t792 = t81.*zeta_dot.*(-7.0./2.0e+1);
t795 = t3.*t374;
t796 = t18.*t372;
t798 = phi_dot.*t17.*t253;
t799 = -t490;
t800 = t17.*t374;
t802 = -t494;
t803 = t18.*t374;
t806 = t4.*t78.*(-1.0./5.0);
t807 = t7.*t78.*(-1.0./5.0);
t808 = t10.*t78.*(-1.0./5.0);
t809 = t13.*t78.*(-1.0./5.0);
t810 = t209.*(-1.0./5.0);
t811 = t210.*(-1.0./5.0);
t812 = t211.*(-1.0./5.0);
t813 = t212.*(-1.0./5.0);
t826 = t77.*t204;
t827 = t10.*t81.*(-1.0./5.0);
t828 = -t547;
t829 = -t548;
t892 = (psi_dot.*t18.*t78)./1.0e+1;
t897 = t20.*t447;
t898 = t21.*t447;
t899 = t23.*t447;
t900 = t24.*t447;
t901 = t26.*t447;
t902 = t27.*t447;
t903 = t29.*t447;
t904 = t30.*t447;
t905 = t6.*t270.*-2.0;
t906 = t15.*t270.*-2.0;
t920 = (psi_dot.*t18.*t81)./1.0e+1;
t929 = -t447;
t930 = phi_dot.*t78.*(-9.0./2.0e+1);
t935 = t78.*zeta_dot.*(-9.0./2.0e+1);
t937 = t17.*t84.*zeta_dot.*(-1.0./5.0);
t938 = t17.*t87.*zeta_dot.*(-1.0./5.0);
t939 = t17.*t90.*zeta_dot.*(-1.0./5.0);
t940 = t17.*t93.*zeta_dot.*(-1.0./5.0);
t1019 = t33.*t447;
t1020 = t34.*t447;
t1021 = t35.*t447;
t1022 = t36.*t447;
t1023 = t37.*t447;
t1024 = t38.*t447;
t1025 = t39.*t447;
t1026 = t40.*t447;
t1074 = t18.*t102.*t156;
t1080 = t18.*t102.*t158;
t1084 = t31+t447;
t1094 = t80.*t84.*(-1.0./5.0);
t1095 = t79.*t87.*(-1.0./5.0);
t1096 = t80.*t87.*(-1.0./5.0);
t1097 = t79.*t90.*(-1.0./5.0);
t1098 = t80.*t93.*(-1.0./5.0);
t1104 = t8.*t447.*-2.0;
t1119 = t80.*t90.*th31_dot.*(-1.0./5.0);
t1131 = t447.*(-1.0./2.0);
t1140 = psi_dot.*t156.*t270;
t1147 = psi_dot.*t158.*t270;
t1150 = t32+t41+t132;
t1151 = t32+t41+t141;
t1152 = t18.*t102.*t272;
t1157 = t79.*t102.*t158;
t1158 = t82.*t102.*t158;
t1167 = psi_dot.*t16.*t270.*(-1.0./2.0);
t1367 = t156+t1132;
t1533 = t101+t113+t118+t123+t294;
t184 = -t112;
t191 = -t116;
t192 = -t117;
t226 = t178.*2.0;
t234 = -t185;
t255 = t31.*t161;
t256 = t31.*t162;
t259 = t31.*t163;
t260 = t31.*t164;
t261 = t31.*t165;
t262 = t31.*t166;
t263 = -t161;
t264 = -t162;
t266 = t31.*t175;
t267 = t31.*t176;
t268 = -t164;
t269 = -t165;
t286 = t217.*2.0;
t307 = -t177;
t308 = -t178;
t310 = t177.*-7.0;
t315 = t187.*-7.0;
t323 = -t240;
t324 = -t241;
t340 = phi_dot.*t232;
t341 = phi_dot.*t233;
t342 = t232.*zeta_dot;
t343 = t233.*zeta_dot;
t344 = t236.*zeta_dot;
t345 = t237.*zeta_dot;
t346 = t238.*zeta_dot;
t347 = t239.*zeta_dot;
t349 = phi_dot.*t240;
t351 = phi_dot.*t241;
t352 = t242.*th11_dot;
t353 = t243.*th21_dot;
t354 = t244.*th31_dot;
t355 = t245.*th41_dot;
t356 = t2.*t207;
t357 = t240.*zeta_dot;
t358 = t2.*t208;
t359 = t241.*zeta_dot;
t366 = t246.*th11_dot;
t367 = t247.*th21_dot;
t368 = t248.*th31_dot;
t369 = t249.*th41_dot;
t370 = t17.*t207;
t371 = t17.*t208;
t376 = t4.*t217;
t377 = t7.*t217;
t378 = t10.*t217;
t379 = t13.*t217;
t380 = t4.*t178;
t381 = t7.*t178;
t382 = t10.*t178;
t383 = t13.*t178;
t384 = -t274;
t385 = -t275;
t386 = -t276;
t387 = -t277;
t392 = -t213;
t393 = -t214;
t394 = -t215;
t395 = -t216;
t396 = -t289;
t401 = -t305;
t402 = -t312;
t403 = t180./5.0;
t404 = t181./5.0;
t405 = t182./5.0;
t406 = t183./5.0;
t407 = t3.*t246;
t410 = t3.*t247;
t413 = t3.*t248;
t416 = t3.*t249;
t423 = -t313;
t426 = -t319;
t427 = -t320;
t428 = -t321;
t429 = -t322;
t430 = -t325;
t434 = -t329;
t437 = bx_dot.*t312;
t441 = t161./1.0e+1;
t442 = t161.*(7.0./2.0e+1);
t443 = t162./1.0e+1;
t444 = t162.*(7.0./2.0e+1);
t445 = bx_dot.*t319;
t446 = by_dot.*t322;
t449 = phi_dot.*t313;
t454 = t163./1.0e+1;
t455 = t164./1.0e+1;
t456 = t163.*(7.0./2.0e+1);
t457 = t164.*(7.0./2.0e+1);
t458 = t165./1.0e+1;
t459 = t166./1.0e+1;
t460 = t165.*(7.0./2.0e+1);
t461 = t166.*(7.0./2.0e+1);
t462 = by_dot.*t328;
t464 = t313.*zeta_dot;
t472 = phi_dot.*t325;
t475 = psi_dot.*t327;
t477 = t175./1.0e+1;
t478 = t175.*(7.0./2.0e+1);
t479 = t176./1.0e+1;
t480 = t176.*(7.0./2.0e+1);
t482 = t2.*t273;
t483 = t325.*zeta_dot;
t485 = t3.*t273;
t486 = t18.*t271;
t493 = t17.*t273;
t495 = t18.*t273;
t505 = t3.*t236;
t508 = t3.*t237;
t511 = t3.*t238;
t514 = t3.*t239;
t529 = t218./5.0;
t531 = t219./5.0;
t533 = t220./5.0;
t535 = t221./5.0;
t561 = t177./1.0e+1;
t562 = t178./1.0e+1;
t563 = t177.*(7.0./2.0e+1);
t564 = t178.*(7.0./2.0e+1);
t570 = -t424;
t571 = t187./1.0e+1;
t572 = t187.*(7.0./2.0e+1);
t573 = t144.*t162;
t574 = t147.*t162;
t575 = t150.*t162;
t576 = t153.*t162;
t577 = phi_dot.*t501;
t578 = phi_dot.*t502;
t579 = phi_dot.*t503;
t580 = phi_dot.*t504;
t581 = t501.*th11_dot;
t582 = t502.*th21_dot;
t583 = t503.*th31_dot;
t584 = t504.*th41_dot;
t586 = t506.*th12_dot;
t587 = t507.*th13_dot;
t589 = t509.*th22_dot;
t590 = t510.*th23_dot;
t592 = t512.*th32_dot;
t593 = t513.*th33_dot;
t595 = t515.*th42_dot;
t596 = t516.*th43_dot;
t597 = t144.*t163;
t598 = t147.*t163;
t599 = t150.*t163;
t600 = t153.*t163;
t601 = (t19.*t162)./5.0;
t602 = t144.*t166;
t603 = (t22.*t162)./5.0;
t604 = t147.*t166;
t605 = (t25.*t162)./5.0;
t606 = t150.*t166;
t607 = (t28.*t162)./5.0;
t608 = t153.*t166;
t609 = t522.*th11_dot;
t610 = t524.*th21_dot;
t611 = t526.*th31_dot;
t612 = t528.*th41_dot;
t614 = phi_dot.*t530;
t616 = phi_dot.*t532;
t618 = phi_dot.*t534;
t620 = phi_dot.*t536;
t621 = psi_dot.*t18.*t236;
t624 = psi_dot.*t18.*t237;
t627 = psi_dot.*t18.*t238;
t630 = psi_dot.*t18.*t239;
t642 = t530.*th11_dot;
t644 = t532.*th21_dot;
t646 = t534.*th31_dot;
t648 = t536.*th41_dot;
t661 = (t19.*t163)./5.0;
t662 = t144.*t175;
t663 = (t22.*t163)./5.0;
t664 = t147.*t175;
t665 = (t25.*t163)./5.0;
t666 = t150.*t175;
t667 = (t28.*t163)./5.0;
t668 = t153.*t175;
t669 = (t19.*t166)./5.0;
t670 = (t22.*t166)./5.0;
t671 = (t25.*t166)./5.0;
t672 = (t28.*t166)./5.0;
t673 = t2.*t242.*zeta_dot;
t674 = t2.*t243.*zeta_dot;
t675 = t2.*t244.*zeta_dot;
t676 = t2.*t245.*zeta_dot;
t677 = t549.*th11_dot;
t678 = t551.*th11_dot;
t679 = t552.*th21_dot;
t680 = t554.*th21_dot;
t681 = t555.*th31_dot;
t682 = t557.*th31_dot;
t683 = t558.*th41_dot;
t684 = t560.*th41_dot;
t685 = t3.*t242.*zeta_dot;
t688 = t3.*t243.*zeta_dot;
t691 = t3.*t244.*zeta_dot;
t694 = t3.*t245.*zeta_dot;
t697 = by_dot.*t424;
t722 = (t19.*t175)./5.0;
t723 = (t22.*t175)./5.0;
t724 = (t25.*t175)./5.0;
t725 = (t28.*t175)./5.0;
t727 = phi_dot.*t424;
t730 = t2.*t246.*zeta_dot;
t731 = t17.*t242.*zeta_dot;
t732 = t2.*t247.*zeta_dot;
t733 = t17.*t243.*zeta_dot;
t734 = t2.*t248.*zeta_dot;
t735 = t17.*t244.*zeta_dot;
t736 = t2.*t249.*zeta_dot;
t737 = t17.*t245.*zeta_dot;
t738 = t419.*th11_dot;
t739 = t420.*th21_dot;
t740 = t421.*th31_dot;
t741 = t422.*th41_dot;
t743 = t408.*zeta_dot;
t744 = t409.*zeta_dot;
t746 = t411.*zeta_dot;
t747 = t412.*zeta_dot;
t749 = t414.*zeta_dot;
t750 = t415.*zeta_dot;
t752 = t417.*zeta_dot;
t753 = t418.*zeta_dot;
t754 = bx_dot.*t431;
t764 = t424.*zeta_dot;
t769 = phi_dot.*t431;
t772 = t17.*t246.*zeta_dot;
t773 = t17.*t247.*zeta_dot;
t774 = t17.*t248.*zeta_dot;
t775 = t17.*t249.*zeta_dot;
t793 = t2.*t375;
t794 = t431.*zeta_dot;
t801 = t17.*t375;
t818 = -t517;
t819 = -t518;
t820 = -t520;
t821 = t213.*(-1.0./5.0);
t822 = t214.*(-1.0./5.0);
t823 = t215.*(-1.0./5.0);
t824 = t216.*(-1.0./5.0);
t825 = t217./1.0e+1;
t832 = -t550;
t833 = -t555;
t834 = -t559;
t841 = t4.*t162.*(-1.0./5.0);
t842 = t7.*t162.*(-1.0./5.0);
t843 = t10.*t162.*(-1.0./5.0);
t844 = t13.*t162.*(-1.0./5.0);
t846 = t162.*t202;
t848 = phi_dot.*t806;
t849 = phi_dot.*t807;
t850 = phi_dot.*t808;
t851 = phi_dot.*t809;
t852 = t806.*th11_dot;
t853 = t807.*th21_dot;
t854 = t808.*th31_dot;
t855 = t809.*th41_dot;
t856 = t810.*th11_dot;
t859 = t811.*th21_dot;
t862 = t812.*th31_dot;
t865 = t813.*th41_dot;
t868 = t4.*t163.*(-1.0./5.0);
t869 = t7.*t163.*(-1.0./5.0);
t870 = t10.*t163.*(-1.0./5.0);
t871 = t13.*t163.*(-1.0./5.0);
t872 = t254./1.0e+1;
t873 = t77.*t271;
t875 = t4.*t166.*(-1.0./5.0);
t877 = t7.*t166.*(-1.0./5.0);
t879 = t10.*t166.*(-1.0./5.0);
t881 = t13.*t166.*(-1.0./5.0);
t886 = t102.*t177;
t889 = t161.*t204;
t893 = t162.*t204;
t894 = t166.*t202;
t908 = t257./1.0e+1;
t909 = t258./1.0e+1;
t910 = t257.*(7.0./2.0e+1);
t911 = t80.*t271;
t912 = t102.*t187;
t915 = t163.*t204;
t916 = t164.*t204;
t921 = t165.*t204;
t922 = t166.*t204;
t923 = -t440;
t926 = t265./1.0e+1;
t928 = t265.*(7.0./2.0e+1);
t932 = t175.*t204;
t934 = t176.*t204;
t941 = t144.*t217;
t942 = t147.*t217;
t943 = t150.*t217;
t944 = t153.*t217;
t945 = t77.*t246;
t946 = t144.*t178;
t947 = t77.*t247;
t948 = t147.*t178;
t949 = t77.*t248;
t950 = t150.*t178;
t951 = t77.*t249;
t952 = t153.*t178;
t954 = bx.*t164.*(-7.0./2.0e+1);
t955 = bx.*t165.*(-7.0./2.0e+1);
t956 = t79.*t246;
t957 = t80.*t246;
t958 = t79.*t247;
t959 = t80.*t247;
t960 = t79.*t248;
t961 = t80.*t248;
t962 = t79.*t249;
t963 = t80.*t249;
t965 = t217.*(-7.0./2.0e+1);
t966 = bx.*t175.*(-1.0./1.0e+1);
t967 = by.*t176.*(-7.0./2.0e+1);
t968 = t82.*t246;
t969 = t82.*t247;
t970 = t82.*t248;
t971 = t82.*t249;
t977 = t161.*t242;
t978 = t161.*t243;
t979 = t161.*t244;
t980 = t161.*t245;
t985 = (t19.*t254)./5.0;
t987 = (t22.*t254)./5.0;
t989 = (t25.*t254)./5.0;
t991 = (t28.*t254)./5.0;
t993 = t161.*t246;
t994 = t164.*t242;
t995 = t161.*t247;
t996 = t164.*t243;
t997 = t161.*t248;
t998 = t164.*t244;
t999 = t161.*t249;
t1000 = t164.*t245;
t1001 = t165.*t242;
t1002 = t165.*t243;
t1003 = t165.*t244;
t1004 = t165.*t245;
t1013 = t16.*t161.*(-1.0./1.0e+1);
t1014 = t16.*t162.*(-7.0./2.0e+1);
t1015 = (t19.*t258)./5.0;
t1016 = (t22.*t258)./5.0;
t1017 = (t25.*t258)./5.0;
t1018 = (t28.*t258)./5.0;
t1027 = t164.*t246;
t1028 = t164.*t247;
t1029 = t164.*t248;
t1030 = t164.*t249;
t1031 = t165.*t246;
t1032 = t176.*t242;
t1033 = t165.*t247;
t1034 = t176.*t243;
t1035 = t165.*t248;
t1036 = t176.*t244;
t1037 = t165.*t249;
t1038 = t176.*t245;
t1040 = t254.*(-7.0./2.0e+1);
t1047 = t18.*t726;
t1049 = t16.*t166.*(-7.0./2.0e+1);
t1050 = t436./2.0;
t1051 = bx_dot.*t178.*(-1.0./1.0e+1);
t1052 = by_dot.*t177.*(-7.0./2.0e+1);
t1053 = t176.*t246;
t1054 = t176.*t247;
t1055 = t176.*t248;
t1056 = t176.*t249;
t1059 = t258.*(-7.0./2.0e+1);
t1063 = t18.*t767;
t1065 = -t920;
t1068 = t440./2.0;
t1069 = t77+t187;
t1070 = t82+t217;
t1071 = t178.*zeta_dot.*(-1.0./1.0e+1);
t1072 = t177.*zeta_dot.*(-7.0./2.0e+1);
t1079 = t187.*zeta_dot.*(-7.0./2.0e+1);
t1099 = t18.*t102.*t207;
t1100 = t4.*t254.*(-1.0./5.0);
t1101 = t7.*t254.*(-1.0./5.0);
t1102 = t10.*t254.*(-1.0./5.0);
t1103 = t13.*t254.*(-1.0./5.0);
t1105 = t84.*t164.*(-1.0./5.0);
t1106 = t87.*t164.*(-1.0./5.0);
t1107 = t90.*t164.*(-1.0./5.0);
t1108 = t93.*t164.*(-1.0./5.0);
t1109 = t84.*t165.*(-1.0./5.0);
t1111 = t87.*t165.*(-1.0./5.0);
t1113 = t90.*t165.*(-1.0./5.0);
t1115 = t93.*t165.*(-1.0./5.0);
t1117 = t1094.*th11_dot;
t1118 = t1096.*th21_dot;
t1120 = t1098.*th41_dot;
t1122 = -t898;
t1123 = -t900;
t1124 = -t902;
t1125 = -t904;
t1126 = t84.*t176.*(-1.0./5.0);
t1127 = t87.*t176.*(-1.0./5.0);
t1128 = t90.*t176.*(-1.0./5.0);
t1129 = t93.*t176.*(-1.0./5.0);
t1135 = bx.*t258.*(-1.0./1.0e+1);
t1136 = by.*t257.*(-7.0./2.0e+1);
t1137 = (t102.*t161)./2.0;
t1141 = t31.*t776;
t1142 = t31.*t779;
t1143 = t31.*t782;
t1144 = t31.*t785;
t1145 = (t102.*t164)./2.0;
t1146 = (t102.*t165)./2.0;
t1148 = (t102.*t176)./2.0;
t1149 = t18.*t102.*t205;
S_dot = ft_2({bx,bx_dot,by,by_dot,bz,bz_dot,p1x,p1x_dot,p1y,p1y_dot,p1z,p2x,p2x_dot,p2y,p2y_dot,p2z,p3x,p3x_dot,p3y,p3y_dot,p3z,p4x,p4x_dot,p4y,p4y_dot,p4z,phi_dot,psi_dot,t10,t100,t1000,t1001,t1002,t1003,t1004,t101,t1013,t1014,t1015,t1016,t1017,t1018,t1019,t102,t1020,t1022,t1023,t1024,t1025,t1026,t1027,t1028,t103,t1030,t1031,t1033,t1037,t104,t1040,t1047,t1049,t105,t1050,t1051,t1052,t1053,t1054,t1056,t1059,t106,t1063,t1065,t1068,t1069,t107,t1070,t1071,t1072,t1074,t1079,t108,t1080,t1084,t109,t1094,t1095,t1096,t1097,t1098,t1099,t11,t110,t1100,t1101,t1102,t1103,t1104,t1105,t1106,t1107,t1108,t1109,t111,t1111,t1113,t1115,t1117,t1118,t1119,t112,t1120,t1122,t1123,t1124,t1125,t1126,t1127,t1128,t1129,t113,t1131,t1135,t1136,t1137,t114,t1140,t1141,t1142,t1143,t1144,t1145,t1146,t1147,t1148,t1149,t115,t1150,t1151,t1152,t1157,t1158,t116,t1167,t117,t118,t119,t12,t120,t125,t126,t128,t129,t13,t131,t133,t134,t135,t136,t1367,t138,t139,t14,t142,t143,t144,t145,t146,t147,t148,t149,t15,t150,t151,t152,t153,t1533,t154,t155,t156,t157,t158,t16,t160,t161,t162,t163,t164,t165,t166,t167,t168,t169,t17,t170,t171,t172,t173,t174,t175,t176,t177,t179,t18,t180,t181,t182,t183,t184,t186,t187,t188,t189,t19,t190,t191,t192,t193,t194,t195,t196,t197,t198,t199,t2,t20,t200,t201,t202,t203,t204,t205,t206,t207,t208,t209,t21,t210,t211,t212,t214,t217,t218,t219,t22,t220,t221,t222,t223,t224,t225,t226,t227,t228,t229,t23,t230,t231,t232,t233,t234,t235,t236,t237,t238,t24,t240,t241,t242,t243,t244,t245,t246,t247,t248,t249,t25,t250,t251,t252,t253,t254,t255,t256,t257,t258,t259,t26,t260,t261,t262,t263,t264,t265,t266,t267,t268,t269,t27,t270,t271,t272,t273,t278,t279,t28,t280,t281,t282,t283,t284,t285,t286,t287,t288,t29,t290,t291,t292,t293,t295,t296,t297,t298,t299,t3,t30,t300,t302,t303,t304,t306,t307,t308,t31,t310,t311,t312,t313,t314,t315,t316,t317,t318,t319,t32,t320,t321,t322,t323,t324,t325,t326,t327,t328,t329,t33,t330,t331,t332,t333,t334,t335,t336,t337,t338,t339,t34,t340,t341,t342,t343,t344,t345,t346,t347,t348,t349,t35,t350,t351,t352,t353,t354,t355,t356,t357,t358,t359,t36,t360,t361,t362,t363,t364,t366,t367,t368,t369,t37,t370,t371,t372,t374,t375,t376,t377,t378,t379,t38,t380,t381,t382,t383,t384,t385,t386,t387,t388,t389,t39,t390,t391,t392,t393,t394,t395,t396,t397,t398,t399,t4,t40,t400,t401,t402,t403,t404,t405,t406,t407,t408,t409,t41,t410,t411,t412,t413,t414,t415,t416,t417,t418,t419,t420,t421,t422,t423,t424,t425,t426,t427,t428,t429,t43,t430,t431,t432,t433,t434,t435,t436,t437,t44,t440,t441,t442,t443,t444,t445,t446,t447,t448,t449,t45,t450,t451,t454,t455,t456,t457,t458,t459,t460,t461,t462,t463,t464,t465,t466,t467,t468,t469,t47,t470,t471,t472,t473,t474,t475,t476,t477,t478,t479,t48,t480,t481,t482,t483,t484,t485,t486,t487,t488,t489,t49,t490,t491,t492,t493,t494,t495,t496,t497,t498,t499,t5,t50,t500,t501,t502,t504,t505,t506,t507,t508,t509,t51,t510,t511,t512,t513,t514,t515,t516,t519,t52,t521,t523,t525,t527,t529,t53,t530,t531,t532,t533,t535,t536,t537,t538,t539,t54,t540,t541,t542,t543,t544,t545,t546,t548,t549,t55,t551,t552,t553,t554,t556,t557,t558,t56,t560,t561,t562,t563,t564,t569,t57,t570,t571,t572,t577,t578,t58,t580,t59,t6,t601,t603,t605,t607,t609,t61,t610,t612,t614,t616,t618,t62,t620,t621,t622,t623,t624,t625,t626,t627,t628,t629,t630,t631,t632,t633,t635,t636,t637,t638,t639,t64,t642,t644,t646,t648,t649,t65,t650,t651,t652,t653,t654,t655,t656,t657,t658,t659,t66,t660,t661,t662,t663,t664,t665,t666,t667,t668,t669,t67,t670,t671,t672,t673,t674,t675,t676,t677,t678,t679,t68,t680,t681,t682,t683,t684,t685,t686,t687,t688,t689,t69,t690,t691,t692,t693,t694,t695,t696,t7,t70,t706,t707,t708,t709,t71,t710,t711,t712,t713,t714,t715,t716,t717,t72,t722,t723,t724,t725,t726,t727,t728,t729,t73,t730,t731,t732,t733,t734,t735,t736,t737,t738,t739,t74,t740,t741,t743,t744,t746,t747,t749,t75,t750,t752,t753,t754,t76,t763,t765,t767,t768,t769,t77,t770,t771,t776,t777,t778,t779,t78,t780,t781,t782,t783,t784,t785,t786,t787,t79,t791,t792,t793,t794,t795,t796,t797,t798,t799,t8,t80,t800,t801,t802,t803,t806,t807,t808,t809,t81,t810,t811,t812,t813,t818,t819,t82,t820,t821,t822,t823,t824,t825,t826,t827,t828,t829,t83,t832,t833,t834,t84,t841,t842,t843,t844,t846,t848,t849,t85,t850,t851,t852,t853,t854,t855,t856,t857,t858,t859,t86,t860,t861,t862,t863,t864,t865,t866,t867,t868,t869,t87,t870,t871,t872,t873,t875,t877,t879,t88,t881,t886,t889,t89,t892,t893,t894,t897,t898,t899,t9,t90,t900,t901,t902,t903,t904,t905,t906,t908,t909,t91,t910,t911,t912,t915,t916,t92,t920,t921,t922,t923,t926,t928,t929,t93,t930,t932,t934,t935,t937,t938,t939,t94,t940,t941,t942,t943,t944,t945,t946,t947,t948,t949,t95,t950,t951,t952,t954,t955,t956,t957,t959,t96,t961,t962,t963,t965,t966,t967,t968,t969,t97,t970,t971,t977,t978,t979,t98,t980,t985,t987,t989,t99,t991,t993,t994,t995,t996,t997,t998,t999,th11_dot,th12_dot,th13_dot,th21_dot,th22_dot,th23_dot,th31_dot,th32_dot,th33_dot,th41_dot,th42_dot,th43_dot,zeta_dot});
end
function S_dot = ft_2(ct)
bx = ct{1};
bx_dot = ct{2};
by = ct{3};
by_dot = ct{4};
bz = ct{5};
bz_dot = ct{6};
p1x = ct{7};
p1x_dot = ct{8};
p1y = ct{9};
p1y_dot = ct{10};
p1z = ct{11};
p2x = ct{12};
p2x_dot = ct{13};
p2y = ct{14};
p2y_dot = ct{15};
p2z = ct{16};
p3x = ct{17};
p3x_dot = ct{18};
p3y = ct{19};
p3y_dot = ct{20};
p3z = ct{21};
p4x = ct{22};
p4x_dot = ct{23};
p4y = ct{24};
p4y_dot = ct{25};
p4z = ct{26};
phi_dot = ct{27};
psi_dot = ct{28};
t10 = ct{29};
t100 = ct{30};
t1000 = ct{31};
t1001 = ct{32};
t1002 = ct{33};
t1003 = ct{34};
t1004 = ct{35};
t101 = ct{36};
t1013 = ct{37};
t1014 = ct{38};
t1015 = ct{39};
t1016 = ct{40};
t1017 = ct{41};
t1018 = ct{42};
t1019 = ct{43};
t102 = ct{44};
t1020 = ct{45};
t1022 = ct{46};
t1023 = ct{47};
t1024 = ct{48};
t1025 = ct{49};
t1026 = ct{50};
t1027 = ct{51};
t1028 = ct{52};
t103 = ct{53};
t1030 = ct{54};
t1031 = ct{55};
t1033 = ct{56};
t1037 = ct{57};
t104 = ct{58};
t1040 = ct{59};
t1047 = ct{60};
t1049 = ct{61};
t105 = ct{62};
t1050 = ct{63};
t1051 = ct{64};
t1052 = ct{65};
t1053 = ct{66};
t1054 = ct{67};
t1056 = ct{68};
t1059 = ct{69};
t106 = ct{70};
t1063 = ct{71};
t1065 = ct{72};
t1068 = ct{73};
t1069 = ct{74};
t107 = ct{75};
t1070 = ct{76};
t1071 = ct{77};
t1072 = ct{78};
t1074 = ct{79};
t1079 = ct{80};
t108 = ct{81};
t1080 = ct{82};
t1084 = ct{83};
t109 = ct{84};
t1094 = ct{85};
t1095 = ct{86};
t1096 = ct{87};
t1097 = ct{88};
t1098 = ct{89};
t1099 = ct{90};
t11 = ct{91};
t110 = ct{92};
t1100 = ct{93};
t1101 = ct{94};
t1102 = ct{95};
t1103 = ct{96};
t1104 = ct{97};
t1105 = ct{98};
t1106 = ct{99};
t1107 = ct{100};
t1108 = ct{101};
t1109 = ct{102};
t111 = ct{103};
t1111 = ct{104};
t1113 = ct{105};
t1115 = ct{106};
t1117 = ct{107};
t1118 = ct{108};
t1119 = ct{109};
t112 = ct{110};
t1120 = ct{111};
t1122 = ct{112};
t1123 = ct{113};
t1124 = ct{114};
t1125 = ct{115};
t1126 = ct{116};
t1127 = ct{117};
t1128 = ct{118};
t1129 = ct{119};
t113 = ct{120};
t1131 = ct{121};
t1135 = ct{122};
t1136 = ct{123};
t1137 = ct{124};
t114 = ct{125};
t1140 = ct{126};
t1141 = ct{127};
t1142 = ct{128};
t1143 = ct{129};
t1144 = ct{130};
t1145 = ct{131};
t1146 = ct{132};
t1147 = ct{133};
t1148 = ct{134};
t1149 = ct{135};
t115 = ct{136};
t1150 = ct{137};
t1151 = ct{138};
t1152 = ct{139};
t1157 = ct{140};
t1158 = ct{141};
t116 = ct{142};
t1167 = ct{143};
t117 = ct{144};
t118 = ct{145};
t119 = ct{146};
t12 = ct{147};
t120 = ct{148};
t125 = ct{149};
t126 = ct{150};
t128 = ct{151};
t129 = ct{152};
t13 = ct{153};
t131 = ct{154};
t133 = ct{155};
t134 = ct{156};
t135 = ct{157};
t136 = ct{158};
t1367 = ct{159};
t138 = ct{160};
t139 = ct{161};
t14 = ct{162};
t142 = ct{163};
t143 = ct{164};
t144 = ct{165};
t145 = ct{166};
t146 = ct{167};
t147 = ct{168};
t148 = ct{169};
t149 = ct{170};
t15 = ct{171};
t150 = ct{172};
t151 = ct{173};
t152 = ct{174};
t153 = ct{175};
t1533 = ct{176};
t154 = ct{177};
t155 = ct{178};
t156 = ct{179};
t157 = ct{180};
t158 = ct{181};
t16 = ct{182};
t160 = ct{183};
t161 = ct{184};
t162 = ct{185};
t163 = ct{186};
t164 = ct{187};
t165 = ct{188};
t166 = ct{189};
t167 = ct{190};
t168 = ct{191};
t169 = ct{192};
t17 = ct{193};
t170 = ct{194};
t171 = ct{195};
t172 = ct{196};
t173 = ct{197};
t174 = ct{198};
t175 = ct{199};
t176 = ct{200};
t177 = ct{201};
t179 = ct{202};
t18 = ct{203};
t180 = ct{204};
t181 = ct{205};
t182 = ct{206};
t183 = ct{207};
t184 = ct{208};
t186 = ct{209};
t187 = ct{210};
t188 = ct{211};
t189 = ct{212};
t19 = ct{213};
t190 = ct{214};
t191 = ct{215};
t192 = ct{216};
t193 = ct{217};
t194 = ct{218};
t195 = ct{219};
t196 = ct{220};
t197 = ct{221};
t198 = ct{222};
t199 = ct{223};
t2 = ct{224};
t20 = ct{225};
t200 = ct{226};
t201 = ct{227};
t202 = ct{228};
t203 = ct{229};
t204 = ct{230};
t205 = ct{231};
t206 = ct{232};
t207 = ct{233};
t208 = ct{234};
t209 = ct{235};
t21 = ct{236};
t210 = ct{237};
t211 = ct{238};
t212 = ct{239};
t214 = ct{240};
t217 = ct{241};
t218 = ct{242};
t219 = ct{243};
t22 = ct{244};
t220 = ct{245};
t221 = ct{246};
t222 = ct{247};
t223 = ct{248};
t224 = ct{249};
t225 = ct{250};
t226 = ct{251};
t227 = ct{252};
t228 = ct{253};
t229 = ct{254};
t23 = ct{255};
t230 = ct{256};
t231 = ct{257};
t232 = ct{258};
t233 = ct{259};
t234 = ct{260};
t235 = ct{261};
t236 = ct{262};
t237 = ct{263};
t238 = ct{264};
t24 = ct{265};
t240 = ct{266};
t241 = ct{267};
t242 = ct{268};
t243 = ct{269};
t244 = ct{270};
t245 = ct{271};
t246 = ct{272};
t247 = ct{273};
t248 = ct{274};
t249 = ct{275};
t25 = ct{276};
t250 = ct{277};
t251 = ct{278};
t252 = ct{279};
t253 = ct{280};
t254 = ct{281};
t255 = ct{282};
t256 = ct{283};
t257 = ct{284};
t258 = ct{285};
t259 = ct{286};
t26 = ct{287};
t260 = ct{288};
t261 = ct{289};
t262 = ct{290};
t263 = ct{291};
t264 = ct{292};
t265 = ct{293};
t266 = ct{294};
t267 = ct{295};
t268 = ct{296};
t269 = ct{297};
t27 = ct{298};
t270 = ct{299};
t271 = ct{300};
t272 = ct{301};
t273 = ct{302};
t278 = ct{303};
t279 = ct{304};
t28 = ct{305};
t280 = ct{306};
t281 = ct{307};
t282 = ct{308};
t283 = ct{309};
t284 = ct{310};
t285 = ct{311};
t286 = ct{312};
t287 = ct{313};
t288 = ct{314};
t29 = ct{315};
t290 = ct{316};
t291 = ct{317};
t292 = ct{318};
t293 = ct{319};
t295 = ct{320};
t296 = ct{321};
t297 = ct{322};
t298 = ct{323};
t299 = ct{324};
t3 = ct{325};
t30 = ct{326};
t300 = ct{327};
t302 = ct{328};
t303 = ct{329};
t304 = ct{330};
t306 = ct{331};
t307 = ct{332};
t308 = ct{333};
t31 = ct{334};
t310 = ct{335};
t311 = ct{336};
t312 = ct{337};
t313 = ct{338};
t314 = ct{339};
t315 = ct{340};
t316 = ct{341};
t317 = ct{342};
t318 = ct{343};
t319 = ct{344};
t32 = ct{345};
t320 = ct{346};
t321 = ct{347};
t322 = ct{348};
t323 = ct{349};
t324 = ct{350};
t325 = ct{351};
t326 = ct{352};
t327 = ct{353};
t328 = ct{354};
t329 = ct{355};
t33 = ct{356};
t330 = ct{357};
t331 = ct{358};
t332 = ct{359};
t333 = ct{360};
t334 = ct{361};
t335 = ct{362};
t336 = ct{363};
t337 = ct{364};
t338 = ct{365};
t339 = ct{366};
t34 = ct{367};
t340 = ct{368};
t341 = ct{369};
t342 = ct{370};
t343 = ct{371};
t344 = ct{372};
t345 = ct{373};
t346 = ct{374};
t347 = ct{375};
t348 = ct{376};
t349 = ct{377};
t35 = ct{378};
t350 = ct{379};
t351 = ct{380};
t352 = ct{381};
t353 = ct{382};
t354 = ct{383};
t355 = ct{384};
t356 = ct{385};
t357 = ct{386};
t358 = ct{387};
t359 = ct{388};
t36 = ct{389};
t360 = ct{390};
t361 = ct{391};
t362 = ct{392};
t363 = ct{393};
t364 = ct{394};
t366 = ct{395};
t367 = ct{396};
t368 = ct{397};
t369 = ct{398};
t37 = ct{399};
t370 = ct{400};
t371 = ct{401};
t372 = ct{402};
t374 = ct{403};
t375 = ct{404};
t376 = ct{405};
t377 = ct{406};
t378 = ct{407};
t379 = ct{408};
t38 = ct{409};
t380 = ct{410};
t381 = ct{411};
t382 = ct{412};
t383 = ct{413};
t384 = ct{414};
t385 = ct{415};
t386 = ct{416};
t387 = ct{417};
t388 = ct{418};
t389 = ct{419};
t39 = ct{420};
t390 = ct{421};
t391 = ct{422};
t392 = ct{423};
t393 = ct{424};
t394 = ct{425};
t395 = ct{426};
t396 = ct{427};
t397 = ct{428};
t398 = ct{429};
t399 = ct{430};
t4 = ct{431};
t40 = ct{432};
t400 = ct{433};
t401 = ct{434};
t402 = ct{435};
t403 = ct{436};
t404 = ct{437};
t405 = ct{438};
t406 = ct{439};
t407 = ct{440};
t408 = ct{441};
t409 = ct{442};
t41 = ct{443};
t410 = ct{444};
t411 = ct{445};
t412 = ct{446};
t413 = ct{447};
t414 = ct{448};
t415 = ct{449};
t416 = ct{450};
t417 = ct{451};
t418 = ct{452};
t419 = ct{453};
t420 = ct{454};
t421 = ct{455};
t422 = ct{456};
t423 = ct{457};
t424 = ct{458};
t425 = ct{459};
t426 = ct{460};
t427 = ct{461};
t428 = ct{462};
t429 = ct{463};
t43 = ct{464};
t430 = ct{465};
t431 = ct{466};
t432 = ct{467};
t433 = ct{468};
t434 = ct{469};
t435 = ct{470};
t436 = ct{471};
t437 = ct{472};
t44 = ct{473};
t440 = ct{474};
t441 = ct{475};
t442 = ct{476};
t443 = ct{477};
t444 = ct{478};
t445 = ct{479};
t446 = ct{480};
t447 = ct{481};
t448 = ct{482};
t449 = ct{483};
t45 = ct{484};
t450 = ct{485};
t451 = ct{486};
t454 = ct{487};
t455 = ct{488};
t456 = ct{489};
t457 = ct{490};
t458 = ct{491};
t459 = ct{492};
t460 = ct{493};
t461 = ct{494};
t462 = ct{495};
t463 = ct{496};
t464 = ct{497};
t465 = ct{498};
t466 = ct{499};
t467 = ct{500};
t468 = ct{501};
t469 = ct{502};
t47 = ct{503};
t470 = ct{504};
t471 = ct{505};
t472 = ct{506};
t473 = ct{507};
t474 = ct{508};
t475 = ct{509};
t476 = ct{510};
t477 = ct{511};
t478 = ct{512};
t479 = ct{513};
t48 = ct{514};
t480 = ct{515};
t481 = ct{516};
t482 = ct{517};
t483 = ct{518};
t484 = ct{519};
t485 = ct{520};
t486 = ct{521};
t487 = ct{522};
t488 = ct{523};
t489 = ct{524};
t49 = ct{525};
t490 = ct{526};
t491 = ct{527};
t492 = ct{528};
t493 = ct{529};
t494 = ct{530};
t495 = ct{531};
t496 = ct{532};
t497 = ct{533};
t498 = ct{534};
t499 = ct{535};
t5 = ct{536};
t50 = ct{537};
t500 = ct{538};
t501 = ct{539};
t502 = ct{540};
t504 = ct{541};
t505 = ct{542};
t506 = ct{543};
t507 = ct{544};
t508 = ct{545};
t509 = ct{546};
t51 = ct{547};
t510 = ct{548};
t511 = ct{549};
t512 = ct{550};
t513 = ct{551};
t514 = ct{552};
t515 = ct{553};
t516 = ct{554};
t519 = ct{555};
t52 = ct{556};
t521 = ct{557};
t523 = ct{558};
t525 = ct{559};
t527 = ct{560};
t529 = ct{561};
t53 = ct{562};
t530 = ct{563};
t531 = ct{564};
t532 = ct{565};
t533 = ct{566};
t535 = ct{567};
t536 = ct{568};
t537 = ct{569};
t538 = ct{570};
t539 = ct{571};
t54 = ct{572};
t540 = ct{573};
t541 = ct{574};
t542 = ct{575};
t543 = ct{576};
t544 = ct{577};
t545 = ct{578};
t546 = ct{579};
t548 = ct{580};
t549 = ct{581};
t55 = ct{582};
t551 = ct{583};
t552 = ct{584};
t553 = ct{585};
t554 = ct{586};
t556 = ct{587};
t557 = ct{588};
t558 = ct{589};
t56 = ct{590};
t560 = ct{591};
t561 = ct{592};
t562 = ct{593};
t563 = ct{594};
t564 = ct{595};
t569 = ct{596};
t57 = ct{597};
t570 = ct{598};
t571 = ct{599};
t572 = ct{600};
t577 = ct{601};
t578 = ct{602};
t58 = ct{603};
t580 = ct{604};
t59 = ct{605};
t6 = ct{606};
t601 = ct{607};
t603 = ct{608};
t605 = ct{609};
t607 = ct{610};
t609 = ct{611};
t61 = ct{612};
t610 = ct{613};
t612 = ct{614};
t614 = ct{615};
t616 = ct{616};
t618 = ct{617};
t62 = ct{618};
t620 = ct{619};
t621 = ct{620};
t622 = ct{621};
t623 = ct{622};
t624 = ct{623};
t625 = ct{624};
t626 = ct{625};
t627 = ct{626};
t628 = ct{627};
t629 = ct{628};
t630 = ct{629};
t631 = ct{630};
t632 = ct{631};
t633 = ct{632};
t635 = ct{633};
t636 = ct{634};
t637 = ct{635};
t638 = ct{636};
t639 = ct{637};
t64 = ct{638};
t642 = ct{639};
t644 = ct{640};
t646 = ct{641};
t648 = ct{642};
t649 = ct{643};
t65 = ct{644};
t650 = ct{645};
t651 = ct{646};
t652 = ct{647};
t653 = ct{648};
t654 = ct{649};
t655 = ct{650};
t656 = ct{651};
t657 = ct{652};
t658 = ct{653};
t659 = ct{654};
t66 = ct{655};
t660 = ct{656};
t661 = ct{657};
t662 = ct{658};
t663 = ct{659};
t664 = ct{660};
t665 = ct{661};
t666 = ct{662};
t667 = ct{663};
t668 = ct{664};
t669 = ct{665};
t67 = ct{666};
t670 = ct{667};
t671 = ct{668};
t672 = ct{669};
t673 = ct{670};
t674 = ct{671};
t675 = ct{672};
t676 = ct{673};
t677 = ct{674};
t678 = ct{675};
t679 = ct{676};
t68 = ct{677};
t680 = ct{678};
t681 = ct{679};
t682 = ct{680};
t683 = ct{681};
t684 = ct{682};
t685 = ct{683};
t686 = ct{684};
t687 = ct{685};
t688 = ct{686};
t689 = ct{687};
t69 = ct{688};
t690 = ct{689};
t691 = ct{690};
t692 = ct{691};
t693 = ct{692};
t694 = ct{693};
t695 = ct{694};
t696 = ct{695};
t7 = ct{696};
t70 = ct{697};
t706 = ct{698};
t707 = ct{699};
t708 = ct{700};
t709 = ct{701};
t71 = ct{702};
t710 = ct{703};
t711 = ct{704};
t712 = ct{705};
t713 = ct{706};
t714 = ct{707};
t715 = ct{708};
t716 = ct{709};
t717 = ct{710};
t72 = ct{711};
t722 = ct{712};
t723 = ct{713};
t724 = ct{714};
t725 = ct{715};
t726 = ct{716};
t727 = ct{717};
t728 = ct{718};
t729 = ct{719};
t73 = ct{720};
t730 = ct{721};
t731 = ct{722};
t732 = ct{723};
t733 = ct{724};
t734 = ct{725};
t735 = ct{726};
t736 = ct{727};
t737 = ct{728};
t738 = ct{729};
t739 = ct{730};
t74 = ct{731};
t740 = ct{732};
t741 = ct{733};
t743 = ct{734};
t744 = ct{735};
t746 = ct{736};
t747 = ct{737};
t749 = ct{738};
t75 = ct{739};
t750 = ct{740};
t752 = ct{741};
t753 = ct{742};
t754 = ct{743};
t76 = ct{744};
t763 = ct{745};
t765 = ct{746};
t767 = ct{747};
t768 = ct{748};
t769 = ct{749};
t77 = ct{750};
t770 = ct{751};
t771 = ct{752};
t776 = ct{753};
t777 = ct{754};
t778 = ct{755};
t779 = ct{756};
t78 = ct{757};
t780 = ct{758};
t781 = ct{759};
t782 = ct{760};
t783 = ct{761};
t784 = ct{762};
t785 = ct{763};
t786 = ct{764};
t787 = ct{765};
t79 = ct{766};
t791 = ct{767};
t792 = ct{768};
t793 = ct{769};
t794 = ct{770};
t795 = ct{771};
t796 = ct{772};
t797 = ct{773};
t798 = ct{774};
t799 = ct{775};
t8 = ct{776};
t80 = ct{777};
t800 = ct{778};
t801 = ct{779};
t802 = ct{780};
t803 = ct{781};
t806 = ct{782};
t807 = ct{783};
t808 = ct{784};
t809 = ct{785};
t81 = ct{786};
t810 = ct{787};
t811 = ct{788};
t812 = ct{789};
t813 = ct{790};
t818 = ct{791};
t819 = ct{792};
t82 = ct{793};
t820 = ct{794};
t821 = ct{795};
t822 = ct{796};
t823 = ct{797};
t824 = ct{798};
t825 = ct{799};
t826 = ct{800};
t827 = ct{801};
t828 = ct{802};
t829 = ct{803};
t83 = ct{804};
t832 = ct{805};
t833 = ct{806};
t834 = ct{807};
t84 = ct{808};
t841 = ct{809};
t842 = ct{810};
t843 = ct{811};
t844 = ct{812};
t846 = ct{813};
t848 = ct{814};
t849 = ct{815};
t85 = ct{816};
t850 = ct{817};
t851 = ct{818};
t852 = ct{819};
t853 = ct{820};
t854 = ct{821};
t855 = ct{822};
t856 = ct{823};
t857 = ct{824};
t858 = ct{825};
t859 = ct{826};
t86 = ct{827};
t860 = ct{828};
t861 = ct{829};
t862 = ct{830};
t863 = ct{831};
t864 = ct{832};
t865 = ct{833};
t866 = ct{834};
t867 = ct{835};
t868 = ct{836};
t869 = ct{837};
t87 = ct{838};
t870 = ct{839};
t871 = ct{840};
t872 = ct{841};
t873 = ct{842};
t875 = ct{843};
t877 = ct{844};
t879 = ct{845};
t88 = ct{846};
t881 = ct{847};
t886 = ct{848};
t889 = ct{849};
t89 = ct{850};
t892 = ct{851};
t893 = ct{852};
t894 = ct{853};
t897 = ct{854};
t898 = ct{855};
t899 = ct{856};
t9 = ct{857};
t90 = ct{858};
t900 = ct{859};
t901 = ct{860};
t902 = ct{861};
t903 = ct{862};
t904 = ct{863};
t905 = ct{864};
t906 = ct{865};
t908 = ct{866};
t909 = ct{867};
t91 = ct{868};
t910 = ct{869};
t911 = ct{870};
t912 = ct{871};
t915 = ct{872};
t916 = ct{873};
t92 = ct{874};
t920 = ct{875};
t921 = ct{876};
t922 = ct{877};
t923 = ct{878};
t926 = ct{879};
t928 = ct{880};
t929 = ct{881};
t93 = ct{882};
t930 = ct{883};
t932 = ct{884};
t934 = ct{885};
t935 = ct{886};
t937 = ct{887};
t938 = ct{888};
t939 = ct{889};
t94 = ct{890};
t940 = ct{891};
t941 = ct{892};
t942 = ct{893};
t943 = ct{894};
t944 = ct{895};
t945 = ct{896};
t946 = ct{897};
t947 = ct{898};
t948 = ct{899};
t949 = ct{900};
t95 = ct{901};
t950 = ct{902};
t951 = ct{903};
t952 = ct{904};
t954 = ct{905};
t955 = ct{906};
t956 = ct{907};
t957 = ct{908};
t959 = ct{909};
t96 = ct{910};
t961 = ct{911};
t962 = ct{912};
t963 = ct{913};
t965 = ct{914};
t966 = ct{915};
t967 = ct{916};
t968 = ct{917};
t969 = ct{918};
t97 = ct{919};
t970 = ct{920};
t971 = ct{921};
t977 = ct{922};
t978 = ct{923};
t979 = ct{924};
t98 = ct{925};
t980 = ct{926};
t985 = ct{927};
t987 = ct{928};
t989 = ct{929};
t99 = ct{930};
t991 = ct{931};
t993 = ct{932};
t994 = ct{933};
t995 = ct{934};
t996 = ct{935};
t997 = ct{936};
t998 = ct{937};
t999 = ct{938};
th11_dot = ct{939};
th12_dot = ct{940};
th13_dot = ct{941};
th21_dot = ct{942};
th22_dot = ct{943};
th23_dot = ct{944};
th31_dot = ct{945};
th32_dot = ct{946};
th33_dot = ct{947};
th41_dot = ct{948};
th42_dot = ct{949};
th43_dot = ct{950};
zeta_dot = ct{951};
t1153 = t16.*t776.*zeta_dot;
t1154 = t16.*t779.*zeta_dot;
t1155 = t16.*t782.*zeta_dot;
t1156 = t16.*t785.*zeta_dot;
t1161 = t84+t388;
t1162 = t87+t389;
t1163 = t90+t390;
t1164 = t93+t391;
t1165 = t31+t929;
t1171 = t41+t83+t135;
t1172 = t41+t83+t138;
t1174 = t897./1.0e+1;
t1175 = t898./1.0e+1;
t1176 = t899./1.0e+1;
t1177 = t900./1.0e+1;
t1178 = t901./1.0e+1;
t1179 = t902./1.0e+1;
t1180 = t903./1.0e+1;
t1181 = t904./1.0e+1;
t1182 = t78.*t776;
t1183 = t78.*t779;
t1184 = t78.*t782;
t1185 = t78.*t785;
t1186 = t102.*t156.*t162;
t1187 = t81.*t776;
t1188 = t81.*t779;
t1189 = t81.*t782;
t1190 = t81.*t785;
t1192 = t102.*t158.*t162;
t1193 = t102.*t156.*t166;
t1195 = t102.*t158.*t163;
t1197 = t102.*t158.*t166;
t1198 = t79.*t102.*t207;
t1200 = t102.*t158.*t175;
t1201 = t82.*t102.*t207;
t1234 = t16.*t102.*t162.*(-1.0./2.0);
t1243 = t18.*t102.*t448;
t1245 = t16.*t102.*t166.*(-1.0./2.0);
t1246 = t102.*t257.*(-1.0./2.0);
t1261 = t190.*t782;
t1326 = t156+t1080;
t1327 = t158+t1074;
t1340 = t246+t810;
t1341 = t247+t811;
t1342 = t248+t812;
t1343 = t249+t813;
t1359 = t167.*t1084;
t1360 = t169.*t1084;
t1361 = t171.*t1084;
t1362 = t173.*t1084;
t1368 = t158+t1131;
t1473 = t85+t278+t897;
t1474 = t88+t280+t899;
t1475 = t91+t282+t901;
t1476 = t94+t284+t903;
t1534 = t97+t113+t118+t126+t297;
t1539 = t777.*t1367;
t1541 = t780.*t1367;
t1543 = t783.*t1367;
t1545 = t786.*t1367;
t1571 = t101+t113+t120+t194+t291;
t1572 = t97+t113+t129+t194+t300;
t1582 = t32+t41+t133+t270+t633;
t1583 = t32+t41+t142+t270+t639;
t1599 = t41+t83+t136+t270+t635;
t1600 = t41+t83+t139+t270+t637;
t1610 = t32+t96+t200+t270+t636;
t1611 = t32+t96+t201+t270+t638;
t1612 = t205+t1140+t1152;
t1634 = t32+t41+t134+t476+t905;
t1635 = t32+t41+t143+t476+t906;
t1640 = t68+t105+t1533;
t1730 = t236+t251+t330+t432+t569;
t1796 = p3z+t51+t203+t244+t314+t327+t543;
t1809 = p2z+t51+t243+t253+t314+t327+t540;
t1810 = p4z+t51+t203+t245+t314+t433+t546;
t1823 = p1z+t51+t242+t253+t314+t433+t537;
t1847 = t43+t113+t118+t197+t296+t447+t1022;
t1851 = t43+t113+t194+t195+t293+t447+t1020;
t1858 = t98+t118+t119+t186+t397+t447+t1019;
t1859 = t113+t118+t160+t198+t299+t447+t1024;
t1860 = t100+t118+t128+t186+t399+t447+t1025;
t1866 = t43+t113+t118+t196+t295+t929+t1104;
t1867 = t100+t125+t186+t194+t398+t447+t1023;
t1868 = t113+t160+t194+t199+t302+t447+t1026;
t309 = -t226;
t438 = -t260;
t439 = -t261;
t452 = -t266;
t453 = -t267;
t565 = -t403;
t566 = -t404;
t567 = -t405;
t568 = -t406;
t585 = t505.*th11_dot;
t588 = t508.*th21_dot;
t591 = t511.*th31_dot;
t594 = t514.*th41_dot;
t613 = phi_dot.*t529;
t615 = phi_dot.*t531;
t617 = phi_dot.*t533;
t619 = phi_dot.*t535;
t641 = t529.*th11_dot;
t643 = t531.*th21_dot;
t645 = t533.*th31_dot;
t647 = t535.*th41_dot;
t698 = -t441;
t699 = -t442;
t700 = -t443;
t701 = -t444;
t702 = phi_dot.*t403;
t703 = phi_dot.*t404;
t704 = phi_dot.*t405;
t705 = phi_dot.*t406;
t718 = t403.*th11_dot;
t719 = t404.*th21_dot;
t720 = t405.*th31_dot;
t721 = t406.*th41_dot;
t742 = t407.*zeta_dot;
t745 = t410.*zeta_dot;
t748 = t413.*zeta_dot;
t751 = t416.*zeta_dot;
t755 = -t454;
t756 = -t455;
t757 = -t456;
t758 = -t457;
t759 = -t458;
t760 = -t459;
t761 = -t460;
t762 = -t461;
t788 = -t477;
t789 = -t478;
t790 = -t480;
t804 = by.*t442;
t805 = bx.*t443;
t814 = bx.*t457;
t815 = by.*t454;
t816 = bx.*t460;
t817 = by.*t459;
t830 = bx.*t477;
t831 = by.*t480;
t835 = -t561;
t836 = -t562;
t837 = -t563;
t838 = -t564;
t839 = bx.*t801;
t840 = -t572;
t845 = t16.*t441;
t847 = by_dot.*t825;
t874 = -t601;
t876 = -t603;
t878 = -t605;
t880 = -t607;
t882 = t821.*th11_dot;
t883 = t822.*th21_dot;
t884 = t823.*th31_dot;
t885 = t824.*th41_dot;
t887 = t255./1.0e+1;
t888 = t16.*t455;
t890 = t18.*t449;
t891 = t256./1.0e+1;
t895 = bx_dot.*t562;
t896 = by_dot.*t563;
t907 = t825.*zeta_dot;
t913 = t259./1.0e+1;
t914 = t260./1.0e+1;
t917 = t18.*t472;
t918 = t261./1.0e+1;
t919 = t262./1.0e+1;
t924 = bx_dot.*t572;
t925 = t562.*zeta_dot;
t927 = t563.*zeta_dot;
t931 = t266./1.0e+1;
t933 = t267./1.0e+1;
t936 = t572.*zeta_dot;
t953 = bx.*t727;
t964 = by.*t769;
t972 = by.*t793;
t973 = t77.*t344;
t974 = t77.*t345;
t975 = t77.*t346;
t976 = t77.*t347;
t981 = t941.*th11_dot;
t982 = t942.*th21_dot;
t983 = t943.*th31_dot;
t984 = t944.*th41_dot;
t986 = t80.*t344;
t988 = t80.*t345;
t990 = t80.*t346;
t992 = t80.*t347;
t1005 = t77.*t366;
t1006 = t946.*th11_dot;
t1007 = t77.*t367;
t1008 = t948.*th21_dot;
t1009 = t77.*t368;
t1010 = t950.*th31_dot;
t1011 = t77.*t369;
t1012 = t952.*th41_dot;
t1039 = -t872;
t1041 = t80.*t366;
t1042 = t80.*t367;
t1043 = t80.*t368;
t1044 = t80.*t369;
t1046 = t255.*(-7.0./2.0e+1);
t1048 = t256.*(-7.0./2.0e+1);
t1057 = -t909;
t1058 = -t910;
t1061 = t259.*(-7.0./2.0e+1);
t1062 = t260.*(-7.0./2.0e+1);
t1066 = t261.*(-7.0./2.0e+1);
t1067 = t262.*(-7.0./2.0e+1);
t1073 = -t928;
t1076 = t266.*(-7.0./2.0e+1);
t1078 = t267.*(-7.0./2.0e+1);
t1081 = by.*t872;
t1083 = by.*t893;
t1085 = bx.*t909;
t1086 = by.*t910;
t1087 = bx.*t915;
t1089 = bx.*t922;
t1091 = bx.*t928;
t1092 = by.*t932;
t1110 = t4.*t267.*(-1.0./5.0);
t1112 = t7.*t267.*(-1.0./5.0);
t1114 = t10.*t267.*(-1.0./5.0);
t1116 = t13.*t267.*(-1.0./5.0);
t1121 = t102.*t307;
t1130 = -t1068;
t1133 = bx.*t255.*(-1.0./1.0e+1);
t1138 = by.*t260.*(-1.0./1.0e+1);
t1139 = by.*t261.*(-1.0./1.0e+1);
t1159 = t79+t308;
t1160 = t80+t307;
t1166 = -t1137;
t1168 = -t1145;
t1169 = -t1146;
t1170 = -t1148;
t1173 = t886.*(-1.0./2.0);
t1191 = t18.*t102.*t340;
t1194 = t18.*t102.*t342;
t1196 = t18.*t102.*t349;
t1199 = t18.*t102.*t357;
t1202 = phi_dot.*t1182;
t1203 = phi_dot.*t1183;
t1204 = phi_dot.*t1184;
t1205 = phi_dot.*t1185;
t1206 = phi_dot.*t1187;
t1207 = phi_dot.*t1188;
t1208 = phi_dot.*t1189;
t1209 = phi_dot.*t1190;
t1210 = t2.*t1141.*zeta_dot;
t1211 = t2.*t1142.*zeta_dot;
t1212 = t2.*t1143.*zeta_dot;
t1213 = t2.*t1144.*zeta_dot;
t1214 = t17.*t1141.*zeta_dot;
t1215 = t17.*t1142.*zeta_dot;
t1216 = t17.*t1143.*zeta_dot;
t1217 = t17.*t1144.*zeta_dot;
t1218 = -t1153;
t1219 = -t1154;
t1220 = -t1155;
t1221 = -t1156;
t1222 = -t1175;
t1223 = -t1177;
t1224 = -t1179;
t1225 = -t1181;
t1226 = t33.*t1070;
t1227 = t34.*t1070;
t1228 = t35.*t1070;
t1229 = t36.*t1070;
t1230 = t37.*t1070;
t1231 = t38.*t1070;
t1232 = t39.*t1070;
t1233 = t40.*t1070;
t1235 = t20.*t1070.*4.0;
t1236 = t21.*t1070.*4.0;
t1237 = t23.*t1070.*4.0;
t1238 = t24.*t1070.*4.0;
t1239 = t26.*t1070.*4.0;
t1240 = t27.*t1070.*4.0;
t1241 = t29.*t1070.*4.0;
t1242 = t30.*t1070.*4.0;
t1244 = t102.*t256.*(-1.0./2.0);
t1247 = t102.*t266.*(-1.0./2.0);
t1248 = t912.*zeta_dot.*(-1.0./2.0);
t1249 = -t1182;
t1250 = -t1183;
t1251 = -t1184;
t1252 = -t1185;
t1253 = t5.*t1070.*-2.0;
t1254 = t6.*t1070.*-2.0;
t1255 = t8.*t1070.*-2.0;
t1256 = t9.*t1070.*-2.0;
t1257 = t11.*t1070.*-2.0;
t1258 = t12.*t1070.*-2.0;
t1259 = t14.*t1070.*-2.0;
t1260 = t15.*t1070.*-2.0;
t1268 = t144.*t1070;
t1269 = t145.*t1070;
t1270 = t146.*t1070;
t1273 = t147.*t1070;
t1274 = t148.*t1070;
t1275 = t149.*t1070;
t1278 = t150.*t1070;
t1279 = t151.*t1070;
t1280 = t152.*t1070;
t1283 = t153.*t1070;
t1284 = t154.*t1070;
t1285 = t155.*t1070;
t1286 = (t19.*t1070)./5.0;
t1288 = (t20.*t1069)./5.0;
t1289 = (t20.*t1070)./5.0;
t1291 = (t21.*t1069)./5.0;
t1292 = (t21.*t1070)./5.0;
t1293 = (t22.*t1070)./5.0;
t1295 = (t23.*t1069)./5.0;
t1296 = (t23.*t1070)./5.0;
t1298 = (t24.*t1069)./5.0;
t1299 = (t24.*t1070)./5.0;
t1300 = (t25.*t1070)./5.0;
t1302 = (t26.*t1069)./5.0;
t1303 = (t26.*t1070)./5.0;
t1305 = (t27.*t1069)./5.0;
t1306 = (t27.*t1070)./5.0;
t1307 = (t28.*t1070)./5.0;
t1309 = (t29.*t1069)./5.0;
t1310 = (t29.*t1070)./5.0;
t1312 = (t30.*t1069)./5.0;
t1313 = (t30.*t1070)./5.0;
t1345 = t5.*t1070.*(-1.0./5.0);
t1346 = t6.*t1070.*(-1.0./5.0);
t1348 = t8.*t1070.*(-1.0./5.0);
t1349 = t9.*t1070.*(-1.0./5.0);
t1351 = t11.*t1070.*(-1.0./5.0);
t1352 = t12.*t1070.*(-1.0./5.0);
t1354 = t14.*t1070.*(-1.0./5.0);
t1355 = t15.*t1070.*(-1.0./5.0);
t1369 = t20.*t1070.*th12_dot.*(-1.0./5.0);
t1370 = t21.*t1070.*th13_dot.*(-1.0./5.0);
t1371 = t23.*t1070.*th22_dot.*(-1.0./5.0);
t1372 = t24.*t1070.*th23_dot.*(-1.0./5.0);
t1373 = t26.*t1070.*th32_dot.*(-1.0./5.0);
t1374 = t27.*t1070.*th33_dot.*(-1.0./5.0);
t1375 = t29.*t1070.*th42_dot.*(-1.0./5.0);
t1376 = t30.*t1070.*th43_dot.*(-1.0./5.0);
t1443 = -t1359;
t1444 = t168.*t1165;
t1445 = -t1360;
t1446 = t170.*t1165;
t1447 = -t1361;
t1448 = t172.*t1165;
t1449 = t174.*t1165;
t1462 = t218+t222+t376;
t1463 = t219+t223+t377;
t1464 = t220+t224+t378;
t1465 = t221+t225+t379;
t1469 = t180+t380+t392;
t1470 = t181+t381+t393;
t1471 = t182+t382+t394;
t1472 = t183+t383+t395;
t1477 = t145.*t1327.*th12_dot;
t1478 = t148.*t1327.*th22_dot;
t1479 = t151.*t1327.*th32_dot;
t1480 = t154.*t1327.*th42_dot;
t1481 = (t20.*t1327.*th12_dot)./5.0;
t1482 = (t23.*t1327.*th22_dot)./5.0;
t1483 = (t26.*t1327.*th32_dot)./5.0;
t1484 = (t29.*t1327.*th42_dot)./5.0;
t1485 = t81+t436+t912;
t1486 = t5.*t1327.*th12_dot.*(-1.0./5.0);
t1487 = t146.*t1368.*th13_dot;
t1488 = t8.*t1327.*th22_dot.*(-1.0./5.0);
t1489 = t149.*t1368.*th23_dot;
t1490 = t11.*t1327.*th32_dot.*(-1.0./5.0);
t1491 = t152.*t1368.*th33_dot;
t1492 = t14.*t1327.*th42_dot.*(-1.0./5.0);
t1493 = t155.*t1368.*th43_dot;
t1494 = t86+t279+t1122;
t1495 = t89+t281+t1123;
t1496 = t92+t283+t1124;
t1497 = t95+t285+t1125;
t1499 = (t21.*t1368.*th13_dot)./5.0;
t1501 = (t24.*t1368.*th23_dot)./5.0;
t1503 = (t27.*t1368.*th33_dot)./5.0;
t1505 = (t30.*t1368.*th43_dot)./5.0;
t1506 = t6.*t1368.*th13_dot.*(-1.0./5.0);
t1507 = t9.*t1368.*th23_dot.*(-1.0./5.0);
t1508 = t12.*t1368.*th33_dot.*(-1.0./5.0);
t1509 = t15.*t1368.*th43_dot.*(-1.0./5.0);
t1519 = t78+t886+t923;
t1520 = t190+t436+t912;
t1525 = t777.*t1327;
t1526 = t778.*t1326;
t1527 = t780.*t1327;
t1528 = t781.*t1326;
t1529 = t783.*t1327;
t1530 = t784.*t1326;
t1531 = t786.*t1327;
t1532 = t787.*t1326;
t1540 = t778.*t1368;
t1542 = t781.*t1368;
t1544 = t784.*t1368;
t1546 = t787.*t1368;
t1547 = t529+t551+t941;
t1548 = t531+t554+t942;
t1549 = t533+t557+t943;
t1550 = t535+t560+t944;
t1563 = (t102.*t777.*t1070)./2.0;
t1564 = (t102.*t778.*t1070)./2.0;
t1565 = (t102.*t780.*t1070)./2.0;
t1566 = (t102.*t781.*t1070)./2.0;
t1567 = (t102.*t783.*t1070)./2.0;
t1568 = (t102.*t784.*t1070)./2.0;
t1569 = (t102.*t786.*t1070)./2.0;
t1570 = (t102.*t787.*t1070)./2.0;
t1576 = t403+t821+t946;
t1577 = t404+t822+t948;
t1578 = t405+t823+t950;
t1579 = t406+t824+t952;
t1601 = t207+t1147+t1149;
t1606 = t331+t506+t1174;
t1607 = t333+t509+t1176;
t1608 = t335+t512+t1178;
t1609 = t337+t515+t1180;
t1613 = t205+t1099+t1167;
t1614 = t272+t1147+t1149;
t1629 = t240+t1050+t1158;
t1638 = t323+t1050+t1158;
t1641 = t69+t105+t1534;
t1645 = t259+t262+t265+t268+t269;
t1646 = t67+t105+t1571;
t1647 = t70+t105+t1572;
t1648 = (t20.*t1612)./5.0;
t1650 = (t23.*t1612)./5.0;
t1652 = (t26.*t1612)./5.0;
t1654 = (t29.*t1612)./5.0;
t1664 = t157+t317+t326+t330+t413;
t1701 = t157+t318+t326+t416+t435;
t1731 = t316+t326+t330+t339+t410;
t1801 = t777.*t1612;
t1803 = t780.*t1612;
t1805 = t783.*t1612;
t1807 = t786.*t1612;
t1839 = t352+t360+t621+t649+t685;
t1840 = t353+t361+t624+t652+t688;
t1841 = t354+t362+t627+t655+t691;
t1842 = t355+t363+t630+t658+t694;
t1848 = p2z+t51+t204+t314+t327+t540+t1142;
t1850 = t44+t52+t109+t118+t186+t399+t1362;
t1852 = p1z+t51+t204+t314+t433+t537+t1141;
t1853 = p3z+t51+t252+t314+t327+t543+t1143;
t1856 = t1162.*t1640;
t1861 = p4z+t51+t252+t314+t433+t546+t1144;
t1872 = t311+t428+t521+t564+t571+t968;
t1875 = t311+t428+t527+t564+t571+t971;
t1876 = t329+t427+t561+t826+t832+t956;
t1879 = t329+t427+t561+t826+t834+t962;
t1898 = t348+t357+t1201+t1243+t1245;
t1900 = t202+t326+t330+t414+t1543;
t1905 = t250+t326+t330+t411+t1541;
t1906 = t202+t326+t417+t435+t1545;
t1907 = t250+t326+t408+t435+t1539;
t1908 = t55+t103+t111+t131+t189+t227+t230+t286+t386+t499;
t1909 = t56+t103+t111+t115+t131+t231+t286+t310+t387+t500;
t1911 = t62+t104+t110+t116+t188+t226+t235+t396+t401+t519;
t1913 = t53+t103+t115+t131+t228+t234+t286+t310+t384+t497;
t1914 = t54+t103+t131+t189+t227+t229+t234+t286+t385+t498;
t1942 = p3x+t45+t233+t328+t421+t429+t563+t808+t825+t949;
t1945 = p3y+t48+t241+t312+t426+t562+t572+t827+t833+t961;
t1951 = p2x+t45+t328+t420+t429+t563+t570+t807+t825+t947;
t1045 = -t887;
t1060 = -t914;
t1064 = -t918;
t1075 = -t931;
t1077 = -t933;
t1082 = bx.*t887;
t1088 = by.*t914;
t1090 = by.*t918;
t1093 = bx.*t933;
t1134 = by.*t1048;
t1262 = -t1202;
t1263 = -t1203;
t1264 = -t1204;
t1265 = -t1205;
t1266 = t33.*t1159;
t1267 = t34.*t1159;
t1271 = t35.*t1159;
t1272 = t36.*t1159;
t1276 = t37.*t1159;
t1277 = t38.*t1159;
t1281 = t39.*t1159;
t1282 = t40.*t1159;
t1287 = t20.*t1159.*4.0;
t1290 = t21.*t1159.*4.0;
t1294 = t23.*t1159.*4.0;
t1297 = t24.*t1159.*4.0;
t1301 = t26.*t1159.*4.0;
t1304 = t27.*t1159.*4.0;
t1308 = t29.*t1159.*4.0;
t1311 = t30.*t1159.*4.0;
S_dot = ft_3({bx,bx_dot,by,by_dot,bz,bz_dot,p1x,p1x_dot,p1y,p1y_dot,p1z,p2x,p2x_dot,p2y,p2y_dot,p2z,p3x,p3x_dot,p3y,p3y_dot,p3z,p4x,p4x_dot,p4y,p4y_dot,phi_dot,psi_dot,t10,t1000,t1001,t1002,t1003,t1004,t1005,t1006,t1007,t1008,t1009,t1010,t1011,t1012,t1013,t1014,t1015,t1016,t1017,t1018,t102,t1027,t1028,t103,t1030,t1031,t1033,t1037,t1039,t104,t1040,t1045,t1046,t1047,t1048,t1049,t105,t1051,t1052,t1053,t1054,t1056,t1057,t1058,t1059,t106,t1060,t1061,t1062,t1063,t1064,t1065,t1066,t1067,t1068,t1069,t107,t1070,t1071,t1072,t1073,t1074,t1075,t1076,t1077,t1078,t1079,t108,t1081,t1083,t1084,t1086,t1087,t1089,t109,t1091,t1092,t1093,t1094,t1095,t1096,t1097,t1098,t11,t110,t1100,t1101,t1102,t1103,t1105,t1106,t1107,t1108,t1109,t1110,t1111,t1112,t1113,t1114,t1115,t1116,t1117,t1118,t1119,t112,t1120,t1121,t1126,t1127,t1128,t1129,t113,t1130,t1131,t1133,t1134,t1135,t1136,t1137,t1138,t1139,t114,t1148,t115,t1150,t1151,t1157,t1159,t1160,t1161,t1163,t1164,t1165,t1166,t1168,t1169,t117,t1170,t1171,t1172,t1173,t118,t1187,t1188,t1190,t1191,t1192,t1193,t1194,t1195,t1196,t1197,t1198,t1199,t12,t1200,t1206,t1207,t1208,t1209,t1210,t1211,t1212,t1213,t1214,t1215,t1216,t1217,t1218,t1219,t1220,t1221,t1222,t1223,t1224,t1225,t1226,t1227,t1228,t1229,t1230,t1231,t1232,t1233,t1234,t1235,t1236,t1237,t1238,t1239,t1240,t1241,t1242,t1244,t1246,t1247,t1248,t1249,t1250,t1251,t1252,t1253,t1254,t1255,t1256,t1257,t1258,t1259,t1260,t1261,t1262,t1263,t1264,t1265,t1266,t1267,t1268,t1269,t1270,t1271,t1272,t1273,t1274,t1275,t1276,t1277,t1278,t1279,t1280,t1281,t1282,t1283,t1284,t1285,t1286,t1287,t1288,t1289,t1290,t1291,t1292,t1293,t1294,t1295,t1296,t1297,t1298,t1299,t13,t1300,t1301,t1302,t1303,t1304,t1305,t1306,t1307,t1308,t1309,t131,t1310,t1311,t1312,t1313,t1326,t1345,t1346,t1348,t1349,t1351,t1352,t1354,t1355,t1367,t1369,t1370,t1371,t1372,t1373,t1374,t1375,t1376,t14,t144,t1443,t1444,t1445,t1446,t1447,t1448,t1449,t145,t146,t1462,t1463,t1464,t1465,t1469,t147,t1470,t1471,t1472,t1473,t1474,t1475,t1476,t148,t1481,t1482,t1483,t1484,t1485,t1486,t1488,t149,t1490,t1492,t1494,t1495,t1496,t1497,t1499,t15,t150,t1501,t1503,t1505,t1506,t1507,t1508,t1509,t151,t1519,t152,t1520,t1525,t1526,t1527,t1528,t1529,t153,t1530,t1531,t1532,t1533,t1534,t154,t1540,t1542,t1544,t1546,t1547,t1548,t1549,t155,t1550,t1563,t1564,t1565,t1566,t1567,t1568,t1569,t1570,t1571,t1572,t1576,t1577,t1578,t1579,t1582,t1583,t1599,t16,t1600,t1601,t1606,t1607,t1608,t1609,t161,t1610,t1611,t1613,t1614,t162,t1629,t163,t1634,t1635,t1638,t164,t1641,t1645,t1646,t1647,t1648,t165,t1650,t1652,t1654,t166,t1664,t167,t168,t169,t17,t170,t1701,t171,t172,t173,t1730,t1731,t174,t175,t176,t177,t179,t1796,t18,t180,t1801,t1803,t1805,t1807,t1809,t181,t1810,t1823,t183,t1839,t184,t1840,t1841,t1842,t1847,t1848,t1850,t1851,t1852,t1853,t1856,t1858,t1859,t186,t1860,t1861,t1866,t1867,t1868,t187,t1872,t1875,t1876,t1879,t188,t189,t1898,t19,t190,t1900,t1905,t1906,t1907,t1908,t1909,t191,t1911,t1913,t1914,t192,t193,t194,t1942,t1945,t1951,t2,t20,t202,t204,t206,t207,t208,t209,t21,t210,t211,t212,t214,t217,t218,t219,t22,t221,t222,t223,t225,t226,t227,t23,t232,t233,t235,t236,t237,t238,t24,t241,t242,t243,t244,t245,t246,t247,t248,t249,t25,t250,t252,t254,t255,t256,t257,t258,t26,t260,t261,t263,t264,t265,t267,t27,t270,t271,t272,t273,t28,t286,t287,t288,t29,t290,t292,t293,t295,t296,t298,t299,t3,t30,t303,t304,t306,t308,t309,t31,t310,t311,t312,t313,t314,t315,t316,t317,t318,t319,t320,t321,t322,t324,t325,t326,t327,t328,t329,t330,t332,t334,t336,t338,t340,t341,t342,t343,t348,t349,t350,t351,t352,t353,t354,t356,t357,t358,t359,t360,t361,t362,t364,t366,t367,t368,t369,t370,t371,t372,t374,t375,t376,t377,t379,t380,t381,t383,t4,t400,t402,t403,t404,t405,t406,t409,t412,t415,t418,t419,t420,t422,t423,t424,t425,t426,t427,t428,t429,t430,t431,t433,t434,t435,t437,t438,t439,t44,t440,t442,t443,t444,t445,t446,t448,t449,t45,t450,t451,t452,t453,t454,t455,t456,t457,t458,t459,t460,t461,t462,t463,t464,t465,t466,t467,t468,t469,t47,t470,t471,t472,t473,t474,t475,t477,t478,t479,t48,t480,t481,t482,t483,t484,t485,t486,t487,t488,t489,t49,t490,t491,t492,t493,t494,t495,t496,t5,t50,t501,t502,t504,t507,t51,t510,t513,t516,t52,t523,t525,t529,t53,t530,t531,t532,t533,t535,t536,t538,t539,t54,t540,t541,t542,t543,t544,t545,t548,t549,t55,t552,t553,t556,t558,t56,t561,t562,t563,t564,t565,t566,t567,t568,t57,t570,t571,t572,t577,t578,t58,t580,t59,t6,t601,t603,t607,t609,t61,t610,t612,t613,t614,t615,t616,t617,t618,t619,t62,t620,t622,t623,t625,t626,t628,t629,t631,t632,t64,t641,t642,t643,t644,t645,t646,t647,t648,t65,t650,t651,t653,t654,t656,t657,t659,t66,t660,t661,t662,t663,t664,t665,t666,t667,t668,t669,t67,t670,t671,t672,t673,t674,t675,t676,t677,t678,t679,t68,t680,t681,t682,t683,t684,t686,t687,t689,t69,t690,t692,t693,t695,t696,t698,t699,t7,t700,t701,t702,t703,t704,t705,t706,t707,t708,t709,t71,t710,t711,t712,t713,t714,t715,t716,t717,t718,t719,t72,t720,t721,t722,t723,t724,t725,t726,t728,t729,t73,t730,t731,t732,t733,t734,t735,t736,t737,t738,t739,t74,t740,t741,t742,t743,t744,t745,t746,t747,t748,t749,t75,t750,t751,t752,t753,t754,t755,t756,t757,t758,t759,t76,t760,t761,t762,t763,t765,t767,t768,t769,t77,t770,t771,t777,t778,t78,t780,t781,t783,t784,t786,t787,t788,t789,t79,t790,t791,t792,t793,t794,t795,t796,t797,t798,t799,t8,t80,t800,t801,t802,t803,t804,t805,t806,t807,t808,t809,t81,t814,t815,t816,t817,t818,t819,t82,t820,t825,t826,t827,t828,t829,t831,t835,t836,t837,t838,t84,t840,t841,t842,t843,t844,t845,t846,t847,t848,t849,t85,t850,t851,t852,t853,t854,t855,t856,t857,t858,t859,t86,t860,t861,t862,t863,t864,t865,t866,t867,t868,t869,t87,t870,t871,t872,t873,t874,t875,t876,t877,t878,t879,t88,t880,t881,t882,t883,t884,t885,t887,t888,t889,t89,t890,t891,t892,t893,t894,t896,t9,t90,t907,t908,t909,t91,t910,t911,t913,t914,t915,t916,t917,t918,t919,t92,t920,t921,t922,t924,t925,t926,t927,t928,t93,t930,t932,t933,t934,t935,t936,t937,t938,t939,t94,t940,t945,t947,t949,t95,t951,t953,t954,t955,t957,t959,t961,t963,t964,t965,t966,t967,t969,t970,t972,t977,t978,t979,t980,t981,t982,t983,t984,t985,t986,t987,t988,t989,t99,t990,t991,t992,t993,t994,t995,t996,t997,t998,t999,th11_dot,th12_dot,th13_dot,th21_dot,th22_dot,th23_dot,th31_dot,th32_dot,th33_dot,th41_dot,th42_dot,th43_dot,zeta_dot});
end
function S_dot = ft_3(ct)
bx = ct{1};
bx_dot = ct{2};
by = ct{3};
by_dot = ct{4};
bz = ct{5};
bz_dot = ct{6};
p1x = ct{7};
p1x_dot = ct{8};
p1y = ct{9};
p1y_dot = ct{10};
p1z = ct{11};
p2x = ct{12};
p2x_dot = ct{13};
p2y = ct{14};
p2y_dot = ct{15};
p2z = ct{16};
p3x = ct{17};
p3x_dot = ct{18};
p3y = ct{19};
p3y_dot = ct{20};
p3z = ct{21};
p4x = ct{22};
p4x_dot = ct{23};
p4y = ct{24};
p4y_dot = ct{25};
phi_dot = ct{26};
psi_dot = ct{27};
t10 = ct{28};
t1000 = ct{29};
t1001 = ct{30};
t1002 = ct{31};
t1003 = ct{32};
t1004 = ct{33};
t1005 = ct{34};
t1006 = ct{35};
t1007 = ct{36};
t1008 = ct{37};
t1009 = ct{38};
t1010 = ct{39};
t1011 = ct{40};
t1012 = ct{41};
t1013 = ct{42};
t1014 = ct{43};
t1015 = ct{44};
t1016 = ct{45};
t1017 = ct{46};
t1018 = ct{47};
t102 = ct{48};
t1027 = ct{49};
t1028 = ct{50};
t103 = ct{51};
t1030 = ct{52};
t1031 = ct{53};
t1033 = ct{54};
t1037 = ct{55};
t1039 = ct{56};
t104 = ct{57};
t1040 = ct{58};
t1045 = ct{59};
t1046 = ct{60};
t1047 = ct{61};
t1048 = ct{62};
t1049 = ct{63};
t105 = ct{64};
t1051 = ct{65};
t1052 = ct{66};
t1053 = ct{67};
t1054 = ct{68};
t1056 = ct{69};
t1057 = ct{70};
t1058 = ct{71};
t1059 = ct{72};
t106 = ct{73};
t1060 = ct{74};
t1061 = ct{75};
t1062 = ct{76};
t1063 = ct{77};
t1064 = ct{78};
t1065 = ct{79};
t1066 = ct{80};
t1067 = ct{81};
t1068 = ct{82};
t1069 = ct{83};
t107 = ct{84};
t1070 = ct{85};
t1071 = ct{86};
t1072 = ct{87};
t1073 = ct{88};
t1074 = ct{89};
t1075 = ct{90};
t1076 = ct{91};
t1077 = ct{92};
t1078 = ct{93};
t1079 = ct{94};
t108 = ct{95};
t1081 = ct{96};
t1083 = ct{97};
t1084 = ct{98};
t1086 = ct{99};
t1087 = ct{100};
t1089 = ct{101};
t109 = ct{102};
t1091 = ct{103};
t1092 = ct{104};
t1093 = ct{105};
t1094 = ct{106};
t1095 = ct{107};
t1096 = ct{108};
t1097 = ct{109};
t1098 = ct{110};
t11 = ct{111};
t110 = ct{112};
t1100 = ct{113};
t1101 = ct{114};
t1102 = ct{115};
t1103 = ct{116};
t1105 = ct{117};
t1106 = ct{118};
t1107 = ct{119};
t1108 = ct{120};
t1109 = ct{121};
t1110 = ct{122};
t1111 = ct{123};
t1112 = ct{124};
t1113 = ct{125};
t1114 = ct{126};
t1115 = ct{127};
t1116 = ct{128};
t1117 = ct{129};
t1118 = ct{130};
t1119 = ct{131};
t112 = ct{132};
t1120 = ct{133};
t1121 = ct{134};
t1126 = ct{135};
t1127 = ct{136};
t1128 = ct{137};
t1129 = ct{138};
t113 = ct{139};
t1130 = ct{140};
t1131 = ct{141};
t1133 = ct{142};
t1134 = ct{143};
t1135 = ct{144};
t1136 = ct{145};
t1137 = ct{146};
t1138 = ct{147};
t1139 = ct{148};
t114 = ct{149};
t1148 = ct{150};
t115 = ct{151};
t1150 = ct{152};
t1151 = ct{153};
t1157 = ct{154};
t1159 = ct{155};
t1160 = ct{156};
t1161 = ct{157};
t1163 = ct{158};
t1164 = ct{159};
t1165 = ct{160};
t1166 = ct{161};
t1168 = ct{162};
t1169 = ct{163};
t117 = ct{164};
t1170 = ct{165};
t1171 = ct{166};
t1172 = ct{167};
t1173 = ct{168};
t118 = ct{169};
t1187 = ct{170};
t1188 = ct{171};
t1190 = ct{172};
t1191 = ct{173};
t1192 = ct{174};
t1193 = ct{175};
t1194 = ct{176};
t1195 = ct{177};
t1196 = ct{178};
t1197 = ct{179};
t1198 = ct{180};
t1199 = ct{181};
t12 = ct{182};
t1200 = ct{183};
t1206 = ct{184};
t1207 = ct{185};
t1208 = ct{186};
t1209 = ct{187};
t1210 = ct{188};
t1211 = ct{189};
t1212 = ct{190};
t1213 = ct{191};
t1214 = ct{192};
t1215 = ct{193};
t1216 = ct{194};
t1217 = ct{195};
t1218 = ct{196};
t1219 = ct{197};
t1220 = ct{198};
t1221 = ct{199};
t1222 = ct{200};
t1223 = ct{201};
t1224 = ct{202};
t1225 = ct{203};
t1226 = ct{204};
t1227 = ct{205};
t1228 = ct{206};
t1229 = ct{207};
t1230 = ct{208};
t1231 = ct{209};
t1232 = ct{210};
t1233 = ct{211};
t1234 = ct{212};
t1235 = ct{213};
t1236 = ct{214};
t1237 = ct{215};
t1238 = ct{216};
t1239 = ct{217};
t1240 = ct{218};
t1241 = ct{219};
t1242 = ct{220};
t1244 = ct{221};
t1246 = ct{222};
t1247 = ct{223};
t1248 = ct{224};
t1249 = ct{225};
t1250 = ct{226};
t1251 = ct{227};
t1252 = ct{228};
t1253 = ct{229};
t1254 = ct{230};
t1255 = ct{231};
t1256 = ct{232};
t1257 = ct{233};
t1258 = ct{234};
t1259 = ct{235};
t1260 = ct{236};
t1261 = ct{237};
t1262 = ct{238};
t1263 = ct{239};
t1264 = ct{240};
t1265 = ct{241};
t1266 = ct{242};
t1267 = ct{243};
t1268 = ct{244};
t1269 = ct{245};
t1270 = ct{246};
t1271 = ct{247};
t1272 = ct{248};
t1273 = ct{249};
t1274 = ct{250};
t1275 = ct{251};
t1276 = ct{252};
t1277 = ct{253};
t1278 = ct{254};
t1279 = ct{255};
t1280 = ct{256};
t1281 = ct{257};
t1282 = ct{258};
t1283 = ct{259};
t1284 = ct{260};
t1285 = ct{261};
t1286 = ct{262};
t1287 = ct{263};
t1288 = ct{264};
t1289 = ct{265};
t1290 = ct{266};
t1291 = ct{267};
t1292 = ct{268};
t1293 = ct{269};
t1294 = ct{270};
t1295 = ct{271};
t1296 = ct{272};
t1297 = ct{273};
t1298 = ct{274};
t1299 = ct{275};
t13 = ct{276};
t1300 = ct{277};
t1301 = ct{278};
t1302 = ct{279};
t1303 = ct{280};
t1304 = ct{281};
t1305 = ct{282};
t1306 = ct{283};
t1307 = ct{284};
t1308 = ct{285};
t1309 = ct{286};
t131 = ct{287};
t1310 = ct{288};
t1311 = ct{289};
t1312 = ct{290};
t1313 = ct{291};
t1326 = ct{292};
t1345 = ct{293};
t1346 = ct{294};
t1348 = ct{295};
t1349 = ct{296};
t1351 = ct{297};
t1352 = ct{298};
t1354 = ct{299};
t1355 = ct{300};
t1367 = ct{301};
t1369 = ct{302};
t1370 = ct{303};
t1371 = ct{304};
t1372 = ct{305};
t1373 = ct{306};
t1374 = ct{307};
t1375 = ct{308};
t1376 = ct{309};
t14 = ct{310};
t144 = ct{311};
t1443 = ct{312};
t1444 = ct{313};
t1445 = ct{314};
t1446 = ct{315};
t1447 = ct{316};
t1448 = ct{317};
t1449 = ct{318};
t145 = ct{319};
t146 = ct{320};
t1462 = ct{321};
t1463 = ct{322};
t1464 = ct{323};
t1465 = ct{324};
t1469 = ct{325};
t147 = ct{326};
t1470 = ct{327};
t1471 = ct{328};
t1472 = ct{329};
t1473 = ct{330};
t1474 = ct{331};
t1475 = ct{332};
t1476 = ct{333};
t148 = ct{334};
t1481 = ct{335};
t1482 = ct{336};
t1483 = ct{337};
t1484 = ct{338};
t1485 = ct{339};
t1486 = ct{340};
t1488 = ct{341};
t149 = ct{342};
t1490 = ct{343};
t1492 = ct{344};
t1494 = ct{345};
t1495 = ct{346};
t1496 = ct{347};
t1497 = ct{348};
t1499 = ct{349};
t15 = ct{350};
t150 = ct{351};
t1501 = ct{352};
t1503 = ct{353};
t1505 = ct{354};
t1506 = ct{355};
t1507 = ct{356};
t1508 = ct{357};
t1509 = ct{358};
t151 = ct{359};
t1519 = ct{360};
t152 = ct{361};
t1520 = ct{362};
t1525 = ct{363};
t1526 = ct{364};
t1527 = ct{365};
t1528 = ct{366};
t1529 = ct{367};
t153 = ct{368};
t1530 = ct{369};
t1531 = ct{370};
t1532 = ct{371};
t1533 = ct{372};
t1534 = ct{373};
t154 = ct{374};
t1540 = ct{375};
t1542 = ct{376};
t1544 = ct{377};
t1546 = ct{378};
t1547 = ct{379};
t1548 = ct{380};
t1549 = ct{381};
t155 = ct{382};
t1550 = ct{383};
t1563 = ct{384};
t1564 = ct{385};
t1565 = ct{386};
t1566 = ct{387};
t1567 = ct{388};
t1568 = ct{389};
t1569 = ct{390};
t1570 = ct{391};
t1571 = ct{392};
t1572 = ct{393};
t1576 = ct{394};
t1577 = ct{395};
t1578 = ct{396};
t1579 = ct{397};
t1582 = ct{398};
t1583 = ct{399};
t1599 = ct{400};
t16 = ct{401};
t1600 = ct{402};
t1601 = ct{403};
t1606 = ct{404};
t1607 = ct{405};
t1608 = ct{406};
t1609 = ct{407};
t161 = ct{408};
t1610 = ct{409};
t1611 = ct{410};
t1613 = ct{411};
t1614 = ct{412};
t162 = ct{413};
t1629 = ct{414};
t163 = ct{415};
t1634 = ct{416};
t1635 = ct{417};
t1638 = ct{418};
t164 = ct{419};
t1641 = ct{420};
t1645 = ct{421};
t1646 = ct{422};
t1647 = ct{423};
t1648 = ct{424};
t165 = ct{425};
t1650 = ct{426};
t1652 = ct{427};
t1654 = ct{428};
t166 = ct{429};
t1664 = ct{430};
t167 = ct{431};
t168 = ct{432};
t169 = ct{433};
t17 = ct{434};
t170 = ct{435};
t1701 = ct{436};
t171 = ct{437};
t172 = ct{438};
t173 = ct{439};
t1730 = ct{440};
t1731 = ct{441};
t174 = ct{442};
t175 = ct{443};
t176 = ct{444};
t177 = ct{445};
t179 = ct{446};
t1796 = ct{447};
t18 = ct{448};
t180 = ct{449};
t1801 = ct{450};
t1803 = ct{451};
t1805 = ct{452};
t1807 = ct{453};
t1809 = ct{454};
t181 = ct{455};
t1810 = ct{456};
t1823 = ct{457};
t183 = ct{458};
t1839 = ct{459};
t184 = ct{460};
t1840 = ct{461};
t1841 = ct{462};
t1842 = ct{463};
t1847 = ct{464};
t1848 = ct{465};
t1850 = ct{466};
t1851 = ct{467};
t1852 = ct{468};
t1853 = ct{469};
t1856 = ct{470};
t1858 = ct{471};
t1859 = ct{472};
t186 = ct{473};
t1860 = ct{474};
t1861 = ct{475};
t1866 = ct{476};
t1867 = ct{477};
t1868 = ct{478};
t187 = ct{479};
t1872 = ct{480};
t1875 = ct{481};
t1876 = ct{482};
t1879 = ct{483};
t188 = ct{484};
t189 = ct{485};
t1898 = ct{486};
t19 = ct{487};
t190 = ct{488};
t1900 = ct{489};
t1905 = ct{490};
t1906 = ct{491};
t1907 = ct{492};
t1908 = ct{493};
t1909 = ct{494};
t191 = ct{495};
t1911 = ct{496};
t1913 = ct{497};
t1914 = ct{498};
t192 = ct{499};
t193 = ct{500};
t194 = ct{501};
t1942 = ct{502};
t1945 = ct{503};
t1951 = ct{504};
t2 = ct{505};
t20 = ct{506};
t202 = ct{507};
t204 = ct{508};
t206 = ct{509};
t207 = ct{510};
t208 = ct{511};
t209 = ct{512};
t21 = ct{513};
t210 = ct{514};
t211 = ct{515};
t212 = ct{516};
t214 = ct{517};
t217 = ct{518};
t218 = ct{519};
t219 = ct{520};
t22 = ct{521};
t221 = ct{522};
t222 = ct{523};
t223 = ct{524};
t225 = ct{525};
t226 = ct{526};
t227 = ct{527};
t23 = ct{528};
t232 = ct{529};
t233 = ct{530};
t235 = ct{531};
t236 = ct{532};
t237 = ct{533};
t238 = ct{534};
t24 = ct{535};
t241 = ct{536};
t242 = ct{537};
t243 = ct{538};
t244 = ct{539};
t245 = ct{540};
t246 = ct{541};
t247 = ct{542};
t248 = ct{543};
t249 = ct{544};
t25 = ct{545};
t250 = ct{546};
t252 = ct{547};
t254 = ct{548};
t255 = ct{549};
t256 = ct{550};
t257 = ct{551};
t258 = ct{552};
t26 = ct{553};
t260 = ct{554};
t261 = ct{555};
t263 = ct{556};
t264 = ct{557};
t265 = ct{558};
t267 = ct{559};
t27 = ct{560};
t270 = ct{561};
t271 = ct{562};
t272 = ct{563};
t273 = ct{564};
t28 = ct{565};
t286 = ct{566};
t287 = ct{567};
t288 = ct{568};
t29 = ct{569};
t290 = ct{570};
t292 = ct{571};
t293 = ct{572};
t295 = ct{573};
t296 = ct{574};
t298 = ct{575};
t299 = ct{576};
t3 = ct{577};
t30 = ct{578};
t303 = ct{579};
t304 = ct{580};
t306 = ct{581};
t308 = ct{582};
t309 = ct{583};
t31 = ct{584};
t310 = ct{585};
t311 = ct{586};
t312 = ct{587};
t313 = ct{588};
t314 = ct{589};
t315 = ct{590};
t316 = ct{591};
t317 = ct{592};
t318 = ct{593};
t319 = ct{594};
t320 = ct{595};
t321 = ct{596};
t322 = ct{597};
t324 = ct{598};
t325 = ct{599};
t326 = ct{600};
t327 = ct{601};
t328 = ct{602};
t329 = ct{603};
t330 = ct{604};
t332 = ct{605};
t334 = ct{606};
t336 = ct{607};
t338 = ct{608};
t340 = ct{609};
t341 = ct{610};
t342 = ct{611};
t343 = ct{612};
t348 = ct{613};
t349 = ct{614};
t350 = ct{615};
t351 = ct{616};
t352 = ct{617};
t353 = ct{618};
t354 = ct{619};
t356 = ct{620};
t357 = ct{621};
t358 = ct{622};
t359 = ct{623};
t360 = ct{624};
t361 = ct{625};
t362 = ct{626};
t364 = ct{627};
t366 = ct{628};
t367 = ct{629};
t368 = ct{630};
t369 = ct{631};
t370 = ct{632};
t371 = ct{633};
t372 = ct{634};
t374 = ct{635};
t375 = ct{636};
t376 = ct{637};
t377 = ct{638};
t379 = ct{639};
t380 = ct{640};
t381 = ct{641};
t383 = ct{642};
t4 = ct{643};
t400 = ct{644};
t402 = ct{645};
t403 = ct{646};
t404 = ct{647};
t405 = ct{648};
t406 = ct{649};
t409 = ct{650};
t412 = ct{651};
t415 = ct{652};
t418 = ct{653};
t419 = ct{654};
t420 = ct{655};
t422 = ct{656};
t423 = ct{657};
t424 = ct{658};
t425 = ct{659};
t426 = ct{660};
t427 = ct{661};
t428 = ct{662};
t429 = ct{663};
t430 = ct{664};
t431 = ct{665};
t433 = ct{666};
t434 = ct{667};
t435 = ct{668};
t437 = ct{669};
t438 = ct{670};
t439 = ct{671};
t44 = ct{672};
t440 = ct{673};
t442 = ct{674};
t443 = ct{675};
t444 = ct{676};
t445 = ct{677};
t446 = ct{678};
t448 = ct{679};
t449 = ct{680};
t45 = ct{681};
t450 = ct{682};
t451 = ct{683};
t452 = ct{684};
t453 = ct{685};
t454 = ct{686};
t455 = ct{687};
t456 = ct{688};
t457 = ct{689};
t458 = ct{690};
t459 = ct{691};
t460 = ct{692};
t461 = ct{693};
t462 = ct{694};
t463 = ct{695};
t464 = ct{696};
t465 = ct{697};
t466 = ct{698};
t467 = ct{699};
t468 = ct{700};
t469 = ct{701};
t47 = ct{702};
t470 = ct{703};
t471 = ct{704};
t472 = ct{705};
t473 = ct{706};
t474 = ct{707};
t475 = ct{708};
t477 = ct{709};
t478 = ct{710};
t479 = ct{711};
t48 = ct{712};
t480 = ct{713};
t481 = ct{714};
t482 = ct{715};
t483 = ct{716};
t484 = ct{717};
t485 = ct{718};
t486 = ct{719};
t487 = ct{720};
t488 = ct{721};
t489 = ct{722};
t49 = ct{723};
t490 = ct{724};
t491 = ct{725};
t492 = ct{726};
t493 = ct{727};
t494 = ct{728};
t495 = ct{729};
t496 = ct{730};
t5 = ct{731};
t50 = ct{732};
t501 = ct{733};
t502 = ct{734};
t504 = ct{735};
t507 = ct{736};
t51 = ct{737};
t510 = ct{738};
t513 = ct{739};
t516 = ct{740};
t52 = ct{741};
t523 = ct{742};
t525 = ct{743};
t529 = ct{744};
t53 = ct{745};
t530 = ct{746};
t531 = ct{747};
t532 = ct{748};
t533 = ct{749};
t535 = ct{750};
t536 = ct{751};
t538 = ct{752};
t539 = ct{753};
t54 = ct{754};
t540 = ct{755};
t541 = ct{756};
t542 = ct{757};
t543 = ct{758};
t544 = ct{759};
t545 = ct{760};
t548 = ct{761};
t549 = ct{762};
t55 = ct{763};
t552 = ct{764};
t553 = ct{765};
t556 = ct{766};
t558 = ct{767};
t56 = ct{768};
t561 = ct{769};
t562 = ct{770};
t563 = ct{771};
t564 = ct{772};
t565 = ct{773};
t566 = ct{774};
t567 = ct{775};
t568 = ct{776};
t57 = ct{777};
t570 = ct{778};
t571 = ct{779};
t572 = ct{780};
t577 = ct{781};
t578 = ct{782};
t58 = ct{783};
t580 = ct{784};
t59 = ct{785};
t6 = ct{786};
t601 = ct{787};
t603 = ct{788};
t607 = ct{789};
t609 = ct{790};
t61 = ct{791};
t610 = ct{792};
t612 = ct{793};
t613 = ct{794};
t614 = ct{795};
t615 = ct{796};
t616 = ct{797};
t617 = ct{798};
t618 = ct{799};
t619 = ct{800};
t62 = ct{801};
t620 = ct{802};
t622 = ct{803};
t623 = ct{804};
t625 = ct{805};
t626 = ct{806};
t628 = ct{807};
t629 = ct{808};
t631 = ct{809};
t632 = ct{810};
t64 = ct{811};
t641 = ct{812};
t642 = ct{813};
t643 = ct{814};
t644 = ct{815};
t645 = ct{816};
t646 = ct{817};
t647 = ct{818};
t648 = ct{819};
t65 = ct{820};
t650 = ct{821};
t651 = ct{822};
t653 = ct{823};
t654 = ct{824};
t656 = ct{825};
t657 = ct{826};
t659 = ct{827};
t66 = ct{828};
t660 = ct{829};
t661 = ct{830};
t662 = ct{831};
t663 = ct{832};
t664 = ct{833};
t665 = ct{834};
t666 = ct{835};
t667 = ct{836};
t668 = ct{837};
t669 = ct{838};
t67 = ct{839};
t670 = ct{840};
t671 = ct{841};
t672 = ct{842};
t673 = ct{843};
t674 = ct{844};
t675 = ct{845};
t676 = ct{846};
t677 = ct{847};
t678 = ct{848};
t679 = ct{849};
t68 = ct{850};
t680 = ct{851};
t681 = ct{852};
t682 = ct{853};
t683 = ct{854};
t684 = ct{855};
t686 = ct{856};
t687 = ct{857};
t689 = ct{858};
t69 = ct{859};
t690 = ct{860};
t692 = ct{861};
t693 = ct{862};
t695 = ct{863};
t696 = ct{864};
t698 = ct{865};
t699 = ct{866};
t7 = ct{867};
t700 = ct{868};
t701 = ct{869};
t702 = ct{870};
t703 = ct{871};
t704 = ct{872};
t705 = ct{873};
t706 = ct{874};
t707 = ct{875};
t708 = ct{876};
t709 = ct{877};
t71 = ct{878};
t710 = ct{879};
t711 = ct{880};
t712 = ct{881};
t713 = ct{882};
t714 = ct{883};
t715 = ct{884};
t716 = ct{885};
t717 = ct{886};
t718 = ct{887};
t719 = ct{888};
t72 = ct{889};
t720 = ct{890};
t721 = ct{891};
t722 = ct{892};
t723 = ct{893};
t724 = ct{894};
t725 = ct{895};
t726 = ct{896};
t728 = ct{897};
t729 = ct{898};
t73 = ct{899};
t730 = ct{900};
t731 = ct{901};
t732 = ct{902};
t733 = ct{903};
t734 = ct{904};
t735 = ct{905};
t736 = ct{906};
t737 = ct{907};
t738 = ct{908};
t739 = ct{909};
t74 = ct{910};
t740 = ct{911};
t741 = ct{912};
t742 = ct{913};
t743 = ct{914};
t744 = ct{915};
t745 = ct{916};
t746 = ct{917};
t747 = ct{918};
t748 = ct{919};
t749 = ct{920};
t75 = ct{921};
t750 = ct{922};
t751 = ct{923};
t752 = ct{924};
t753 = ct{925};
t754 = ct{926};
t755 = ct{927};
t756 = ct{928};
t757 = ct{929};
t758 = ct{930};
t759 = ct{931};
t76 = ct{932};
t760 = ct{933};
t761 = ct{934};
t762 = ct{935};
t763 = ct{936};
t765 = ct{937};
t767 = ct{938};
t768 = ct{939};
t769 = ct{940};
t77 = ct{941};
t770 = ct{942};
t771 = ct{943};
t777 = ct{944};
t778 = ct{945};
t78 = ct{946};
t780 = ct{947};
t781 = ct{948};
t783 = ct{949};
t784 = ct{950};
t786 = ct{951};
t787 = ct{952};
t788 = ct{953};
t789 = ct{954};
t79 = ct{955};
t790 = ct{956};
t791 = ct{957};
t792 = ct{958};
t793 = ct{959};
t794 = ct{960};
t795 = ct{961};
t796 = ct{962};
t797 = ct{963};
t798 = ct{964};
t799 = ct{965};
t8 = ct{966};
t80 = ct{967};
t800 = ct{968};
t801 = ct{969};
t802 = ct{970};
t803 = ct{971};
t804 = ct{972};
t805 = ct{973};
t806 = ct{974};
t807 = ct{975};
t808 = ct{976};
t809 = ct{977};
t81 = ct{978};
t814 = ct{979};
t815 = ct{980};
t816 = ct{981};
t817 = ct{982};
t818 = ct{983};
t819 = ct{984};
t82 = ct{985};
t820 = ct{986};
t825 = ct{987};
t826 = ct{988};
t827 = ct{989};
t828 = ct{990};
t829 = ct{991};
t831 = ct{992};
t835 = ct{993};
t836 = ct{994};
t837 = ct{995};
t838 = ct{996};
t84 = ct{997};
t840 = ct{998};
t841 = ct{999};
t842 = ct{1000};
t843 = ct{1001};
t844 = ct{1002};
t845 = ct{1003};
t846 = ct{1004};
t847 = ct{1005};
t848 = ct{1006};
t849 = ct{1007};
t85 = ct{1008};
t850 = ct{1009};
t851 = ct{1010};
t852 = ct{1011};
t853 = ct{1012};
t854 = ct{1013};
t855 = ct{1014};
t856 = ct{1015};
t857 = ct{1016};
t858 = ct{1017};
t859 = ct{1018};
t86 = ct{1019};
t860 = ct{1020};
t861 = ct{1021};
t862 = ct{1022};
t863 = ct{1023};
t864 = ct{1024};
t865 = ct{1025};
t866 = ct{1026};
t867 = ct{1027};
t868 = ct{1028};
t869 = ct{1029};
t87 = ct{1030};
t870 = ct{1031};
t871 = ct{1032};
t872 = ct{1033};
t873 = ct{1034};
t874 = ct{1035};
t875 = ct{1036};
t876 = ct{1037};
t877 = ct{1038};
t878 = ct{1039};
t879 = ct{1040};
t88 = ct{1041};
t880 = ct{1042};
t881 = ct{1043};
t882 = ct{1044};
t883 = ct{1045};
t884 = ct{1046};
t885 = ct{1047};
t887 = ct{1048};
t888 = ct{1049};
t889 = ct{1050};
t89 = ct{1051};
t890 = ct{1052};
t891 = ct{1053};
t892 = ct{1054};
t893 = ct{1055};
t894 = ct{1056};
t896 = ct{1057};
t9 = ct{1058};
t90 = ct{1059};
t907 = ct{1060};
t908 = ct{1061};
t909 = ct{1062};
t91 = ct{1063};
t910 = ct{1064};
t911 = ct{1065};
t913 = ct{1066};
t914 = ct{1067};
t915 = ct{1068};
t916 = ct{1069};
t917 = ct{1070};
t918 = ct{1071};
t919 = ct{1072};
t92 = ct{1073};
t920 = ct{1074};
t921 = ct{1075};
t922 = ct{1076};
t924 = ct{1077};
t925 = ct{1078};
t926 = ct{1079};
t927 = ct{1080};
t928 = ct{1081};
t93 = ct{1082};
t930 = ct{1083};
t932 = ct{1084};
t933 = ct{1085};
t934 = ct{1086};
t935 = ct{1087};
t936 = ct{1088};
t937 = ct{1089};
t938 = ct{1090};
t939 = ct{1091};
t94 = ct{1092};
t940 = ct{1093};
t945 = ct{1094};
t947 = ct{1095};
t949 = ct{1096};
t95 = ct{1097};
t951 = ct{1098};
t953 = ct{1099};
t954 = ct{1100};
t955 = ct{1101};
t957 = ct{1102};
t959 = ct{1103};
t961 = ct{1104};
t963 = ct{1105};
t964 = ct{1106};
t965 = ct{1107};
t966 = ct{1108};
t967 = ct{1109};
t969 = ct{1110};
t970 = ct{1111};
t972 = ct{1112};
t977 = ct{1113};
t978 = ct{1114};
t979 = ct{1115};
t980 = ct{1116};
t981 = ct{1117};
t982 = ct{1118};
t983 = ct{1119};
t984 = ct{1120};
t985 = ct{1121};
t986 = ct{1122};
t987 = ct{1123};
t988 = ct{1124};
t989 = ct{1125};
t99 = ct{1126};
t990 = ct{1127};
t991 = ct{1128};
t992 = ct{1129};
t993 = ct{1130};
t994 = ct{1131};
t995 = ct{1132};
t996 = ct{1133};
t997 = ct{1134};
t998 = ct{1135};
t999 = ct{1136};
th11_dot = ct{1137};
th12_dot = ct{1138};
th13_dot = ct{1139};
th21_dot = ct{1140};
th22_dot = ct{1141};
th23_dot = ct{1142};
th31_dot = ct{1143};
th32_dot = ct{1144};
th33_dot = ct{1145};
th41_dot = ct{1146};
th42_dot = ct{1147};
th43_dot = ct{1148};
zeta_dot = ct{1149};
t1314 = t1268.*th11_dot;
t1315 = t1269.*th12_dot;
t1316 = t1270.*th13_dot;
t1317 = t1273.*th21_dot;
t1318 = t1274.*th22_dot;
t1319 = t1275.*th23_dot;
t1320 = t1278.*th31_dot;
t1321 = t1279.*th32_dot;
t1322 = t1280.*th33_dot;
t1323 = t1283.*th41_dot;
t1324 = t1284.*th42_dot;
t1325 = t1285.*th43_dot;
t1328 = t1286.*th11_dot;
t1329 = t1289.*th12_dot;
t1330 = t1292.*th13_dot;
t1331 = t1293.*th21_dot;
t1332 = t1296.*th22_dot;
t1333 = t1299.*th23_dot;
t1334 = t1300.*th31_dot;
t1335 = t1303.*th32_dot;
t1336 = t1306.*th33_dot;
t1337 = t1307.*th41_dot;
t1338 = t1310.*th42_dot;
t1339 = t1313.*th43_dot;
t1344 = t5.*t1159.*-2.0;
t1347 = t8.*t1159.*-2.0;
t1350 = t11.*t1159.*-2.0;
t1353 = t14.*t1159.*-2.0;
t1363 = t1351.*th32_dot;
t1364 = t1352.*th33_dot;
t1365 = t1354.*th42_dot;
t1366 = t1355.*th43_dot;
t1377 = t144.*t1159;
t1378 = t145.*t1159;
t1379 = t146.*t1159;
t1380 = t147.*t1159;
t1381 = t148.*t1159;
t1382 = t149.*t1159;
t1383 = t150.*t1159;
t1384 = t151.*t1159;
t1385 = t152.*t1159;
t1386 = t153.*t1159;
t1387 = t154.*t1159;
t1388 = t155.*t1159;
t1389 = (t19.*t1159)./5.0;
t1390 = (t20.*t1159)./5.0;
t1391 = (t20.*t1160)./5.0;
t1392 = (t21.*t1159)./5.0;
t1393 = (t21.*t1160)./5.0;
t1394 = (t22.*t1159)./5.0;
t1395 = (t23.*t1159)./5.0;
t1396 = (t23.*t1160)./5.0;
t1397 = (t24.*t1159)./5.0;
t1398 = (t24.*t1160)./5.0;
t1399 = (t25.*t1159)./5.0;
t1400 = (t26.*t1159)./5.0;
t1401 = (t26.*t1160)./5.0;
t1402 = (t27.*t1159)./5.0;
t1403 = (t27.*t1160)./5.0;
t1404 = (t28.*t1159)./5.0;
t1405 = (t29.*t1159)./5.0;
t1406 = (t29.*t1160)./5.0;
t1407 = (t30.*t1159)./5.0;
t1408 = (t30.*t1160)./5.0;
t1433 = t5.*t1159.*(-1.0./5.0);
t1434 = t8.*t1159.*(-1.0./5.0);
t1435 = t11.*t1159.*(-1.0./5.0);
t1436 = t14.*t1159.*(-1.0./5.0);
t1450 = t4.*t1159.*th11_dot.*(-1.0./5.0);
t1451 = t7.*t1159.*th21_dot.*(-1.0./5.0);
t1453 = t9.*t1159.*th23_dot.*(-1.0./5.0);
t1454 = t10.*t1159.*th31_dot.*(-1.0./5.0);
t1456 = t12.*t1159.*th33_dot.*(-1.0./5.0);
t1457 = t13.*t1159.*th41_dot.*(-1.0./5.0);
t1458 = t21.*t1159.*th13_dot.*(-1.0./5.0);
t1459 = t24.*t1159.*th23_dot.*(-1.0./5.0);
t1460 = t27.*t1159.*th33_dot.*(-1.0./5.0);
t1461 = t30.*t1159.*th43_dot.*(-1.0./5.0);
t1466 = -t1444;
t1467 = -t1446;
t1468 = -t1448;
t1498 = -t1481;
t1500 = -t1482;
t1502 = -t1483;
t1504 = -t1484;
t1510 = -t1499;
t1511 = -t1501;
t1512 = -t1503;
t1513 = -t1505;
t1514 = t529+t1268;
t1515 = t531+t1273;
t1516 = t533+t1278;
t1517 = t535+t1283;
t1518 = t78+t440+t1121;
t1521 = t21.*t1485;
t1522 = t24.*t1485;
t1523 = t27.*t1485;
t1524 = t30.*t1485;
t1552 = t21.*t1519;
t1554 = t24.*t1519;
t1556 = t27.*t1519;
t1558 = t30.*t1519;
t1559 = t20.*t1520;
t1560 = t23.*t1520;
t1561 = t26.*t1520;
t1562 = t29.*t1520;
t1573 = -t1525;
t1574 = -t1527;
t1575 = -t1529;
t1580 = -t1565;
t1581 = -t1567;
t1584 = -t1540;
t1585 = -t1542;
t1586 = -t1544;
t1587 = t168.*t1485;
t1588 = t170.*t1485;
t1589 = t172.*t1485;
t1590 = t174.*t1485;
t1591 = (t102.*t777.*t1159)./2.0;
t1592 = (t102.*t778.*t1159)./2.0;
t1593 = (t102.*t780.*t1159)./2.0;
t1594 = (t102.*t781.*t1159)./2.0;
t1595 = (t102.*t783.*t1159)./2.0;
t1596 = (t102.*t784.*t1159)./2.0;
t1597 = (t102.*t786.*t1159)./2.0;
t1598 = (t102.*t787.*t1159)./2.0;
t1616 = t168.*t1519;
t1618 = t170.*t1519;
t1620 = t172.*t1519;
t1622 = t174.*t1519;
t1623 = t167.*t1520;
t1625 = t169.*t1520;
t1626 = t171.*t1520;
t1627 = t173.*t1520;
t1630 = t332+t507+t1222;
t1631 = t334+t510+t1223;
t1632 = t336+t513+t1224;
t1633 = t338+t516+t1225;
t1636 = t232+t1130+t1157;
t1637 = t232+t1068+t1173;
t1642 = t163+t166+t254+t438+t439;
t1643 = t176+t256+t257+t263+t452;
t1644 = t175+t255+t258+t264+t453;
t1649 = (t21.*t1613)./5.0;
t1651 = (t24.*t1613)./5.0;
t1653 = (t27.*t1613)./5.0;
t1655 = (t30.*t1613)./5.0;
t1656 = (t21.*t1629)./5.0;
t1657 = (t24.*t1629)./5.0;
t1658 = (t27.*t1629)./5.0;
t1659 = (t30.*t1629)./5.0;
t1660 = t146.*t1629.*th13_dot;
t1661 = t149.*t1629.*th23_dot;
t1662 = t152.*t1629.*th33_dot;
t1663 = t155.*t1629.*th43_dot;
t1669 = -t1648;
t1671 = -t1650;
t1673 = -t1652;
t1675 = -t1654;
t1685 = (t20.*t1638)./5.0;
t1686 = (t23.*t1638)./5.0;
t1687 = (t26.*t1638)./5.0;
t1688 = (t29.*t1638)./5.0;
t1689 = t145.*t1638.*th12_dot;
t1692 = t148.*t1638.*th22_dot;
t1695 = t151.*t1638.*th32_dot;
t1698 = t154.*t1638.*th42_dot;
t1704 = t24.*t1629.*th23_dot.*(-1.0./5.0);
t1706 = t27.*t1629.*th33_dot.*(-1.0./5.0);
t1720 = t20.*t1638.*th12_dot.*(-1.0./5.0);
t1721 = t29.*t1638.*th42_dot.*(-1.0./5.0);
t1797 = t778.*t1629;
t1798 = t781.*t1629;
t1799 = t784.*t1629;
t1800 = t787.*t1629;
t1802 = t778.*t1613;
t1804 = t781.*t1613;
t1806 = t784.*t1613;
t1808 = t787.*t1613;
t1819 = t777.*t1638;
t1820 = t780.*t1638;
t1821 = t783.*t1638;
t1822 = t786.*t1638;
t1849 = t44+t68+t105+t113+t118+t295+t1445;
t1854 = t44+t67+t105+t113+t194+t292+t1443;
t1855 = t69+t99+t105+t113+t118+t298+t1447;
t1857 = t1163.*t1641;
t1863 = t44+t52+t109+t118+t186+t400+t1449;
t1864 = t1161.*t1646;
t1865 = t1164.*t1647;
t1873 = t311+t321+t523+t571+t838+t969;
t1874 = t311+t321+t525+t571+t838+t970;
t1877 = t320+t329+t553+t826+t835+t1095;
t1878 = t320+t329+t556+t826+t835+t1097;
t1896 = t348+t357+t1191+t1193+t1248;
t1897 = t202+t326+t330+t415+t1530;
t1899 = t250+t326+t330+t412+t1528;
t1901 = t202+t326+t418+t435+t1532;
t1902 = t364+t463+t1196+t1198+t1234;
t1903 = t342+t487+t1196+t1198+t1234;
t1904 = t250+t326+t409+t435+t1526;
t1910 = t49+t106+t110+t114+t193+t235+t287+t303+t309+t818;
t1912 = t49+t108+t110+t114+t191+t235+t290+t306+t309+t820;
t1916 = bz+t66+t204+t327+t425+t828+t1531;
t1917 = t49+t107+t114+t179+t193+t288+t304+t309+t315+t819;
t1921 = bz+t66+t204+t327+t425+t829+t1546;
t1922 = -t1848.*(t210./5.0-t247);
t1925 = -t1852.*(t209./5.0-t246);
t1926 = -t1853.*(t211./5.0-t248);
t1927 = t1848.*(t210./5.0-t247);
t1928 = -t1861.*(t212./5.0-t249);
t1929 = t1852.*(t209./5.0-t246);
t1930 = t1861.*(t212./5.0-t249);
t1932 = t1476.*t1850;
t1939 = t313+t328+t429+t563+t825+t1251+t1300;
t1943 = p4x+t45+t233+t322+t328+t422+t809+t825+t837+t951;
t1946 = by+t59+t312+t319+t324+t536+t558+t572+t836+t1098;
t1948 = by+t57+t312+t319+t431+t530+t549+t572+t836+t1094;
t1950 = p1x+t45+t322+t328+t419+t570+t806+t825+t837+t945;
t1952 = by+t58+t319+t402+t431+t532+t552+t836+t840+t1096;
t1954 = p4x+t45+t313+t322+t328+t825+t837+t1252+t1307;
t1956 = p1x+t45+t322+t328+t423+t825+t837+t1249+t1286;
t1957 = p2x+t45+t328+t423+t429+t563+t825+t1250+t1293;
t1975 = t1464.*t1908;
t1976 = t1465.*t1909;
t1977 = t349+t356+t1148+t1166+t1192+t1194+t1247;
t1980 = t349+t356+t1137+t1170+t1200+t1244+t1246;
t1981 = t370+t448+t1168+t1169+t1195+t1197+t1199;
t1982 = t340+t491+t1168+t1169+t1195+t1197+t1199;
t1987 = t1462.*t1913;
t1988 = t1463.*t1914;
t1996 = t1471.*t1911;
t2005 = t1796.*t1841;
t2012 = t1809.*t1840;
t2013 = t1810.*t1842;
t2035 = t1823.*t1839;
t2044 = bz_dot+t75+t206+t368+t468+t473+t484+t495+t712+t729+t748+t862;
t2045 = bz_dot+t76+t206+t369+t451+t469+t473+t484+t715+t751+t803+t865;
t2050 = t1840.*t1848;
t2051 = t1839.*t1852;
t2052 = t1841.*t1853;
t2057 = t1842.*t1861;
t2058 = bz_dot+t73+t366+t451+t466+t473+t484+t496+t706+t742+t803+t856;
t2059 = bz_dot+t74+t367+t467+t473+t484+t495+t496+t709+t729+t745+t859;
t2080 = bz_dot+t75+t271+t368+t473+t484+t495+t712+t729+t748+t862+t1220;
t2081 = bz_dot+t76+t271+t369+t451+t473+t484+t715+t751+t803+t865+t1221;
t2082 = bz_dot+t73+t366+t372+t451+t473+t484+t706+t742+t803+t856+t1218;
t2083 = bz_dot+t74+t367+t372+t473+t484+t495+t709+t729+t745+t859+t1219;
t2094 = t702+t730+t738+t852+t868+t875+t994+t1001+t1005+t1100;
t2095 = t703+t732+t739+t853+t869+t877+t996+t1002+t1007+t1101;
t2096 = t704+t734+t740+t854+t870+t879+t998+t1003+t1009+t1102;
t2097 = t705+t736+t741+t855+t871+t881+t1000+t1004+t1011+t1103;
t2098 = t613+t642+t662+t677+t841+t937+t977+t986+t1110+t1117;
t2099 = t615+t644+t664+t679+t842+t938+t978+t988+t1112+t1118;
t2100 = t617+t646+t666+t681+t843+t939+t979+t990+t1114+t1119;
t2101 = t619+t648+t668+t683+t844+t940+t980+t992+t1116+t1120;
t1356 = -t1297;
t1357 = -t1301;
t1358 = -t1304;
t1409 = t1377.*th11_dot;
t1410 = t1378.*th12_dot;
t1411 = t1379.*th13_dot;
t1412 = t1380.*th21_dot;
t1413 = t1381.*th22_dot;
t1414 = t1382.*th23_dot;
t1415 = t1383.*th31_dot;
t1416 = t1384.*th32_dot;
t1417 = t1385.*th33_dot;
t1418 = t1386.*th41_dot;
t1419 = t1387.*th42_dot;
t1420 = t1388.*th43_dot;
t1421 = t1389.*th11_dot;
t1422 = t1390.*th12_dot;
t1423 = t1392.*th13_dot;
t1424 = t1394.*th21_dot;
t1425 = t1395.*th22_dot;
t1426 = t1397.*th23_dot;
t1427 = t1399.*th31_dot;
t1428 = t1400.*th32_dot;
t1429 = t1402.*th33_dot;
t1430 = t1404.*th41_dot;
t1431 = t1405.*th42_dot;
t1432 = t1407.*th43_dot;
t1437 = -t1391;
t1438 = -t1397;
t1439 = -t1399;
t1440 = -t1400;
t1441 = -t1402;
t1442 = -t1406;
t1452 = t1434.*th22_dot;
t1455 = t1435.*th32_dot;
t1535 = t565+t1377;
t1536 = t566+t1380;
t1537 = t567+t1383;
t1538 = t568+t1386;
t1551 = t20.*t1518;
t1553 = t23.*t1518;
t1555 = t26.*t1518;
t1557 = t29.*t1518;
t1602 = -t1591;
t1603 = -t1593;
t1604 = -t1595;
t1605 = -t1597;
t1615 = t167.*t1518;
t1617 = t169.*t1518;
t1619 = t171.*t1518;
t1621 = t173.*t1518;
t1624 = -t1587;
t1628 = -t1590;
t1639 = -t1626;
t1665 = t1656.*th13_dot;
t1666 = t1657.*th23_dot;
t1667 = t1658.*th33_dot;
t1668 = t1659.*th43_dot;
t1670 = -t1649;
t1672 = -t1651;
t1674 = -t1653;
t1676 = -t1655;
t1677 = (t20.*t1637)./5.0;
t1678 = (t21.*t1636)./5.0;
t1679 = (t23.*t1637)./5.0;
t1680 = (t24.*t1636)./5.0;
t1681 = (t26.*t1637)./5.0;
t1682 = (t27.*t1636)./5.0;
t1683 = (t29.*t1637)./5.0;
t1684 = (t30.*t1636)./5.0;
t1702 = t1685.*th12_dot;
t1703 = t1686.*th22_dot;
t1705 = t1687.*th32_dot;
t1707 = t1688.*th42_dot;
t1708 = t145.*t1637.*th12_dot;
t1709 = t146.*t1636.*th13_dot;
t1710 = t148.*t1637.*th22_dot;
t1711 = t149.*t1636.*th23_dot;
t1712 = t151.*t1637.*th32_dot;
t1713 = t152.*t1636.*th33_dot;
t1714 = t154.*t1637.*th42_dot;
t1715 = t155.*t1636.*th43_dot;
t1716 = t20.*t1637.*th12_dot.*(-1.0./5.0);
t1717 = t21.*t1636.*th13_dot.*(-1.0./5.0);
t1718 = t23.*t1637.*th22_dot.*(-1.0./5.0);
t1719 = t24.*t1636.*th23_dot.*(-1.0./5.0);
t1722 = t5.*t1637.*th12_dot.*(-1.0./5.0);
t1723 = t6.*t1636.*th13_dot.*(-1.0./5.0);
t1724 = t8.*t1637.*th22_dot.*(-1.0./5.0);
t1725 = t9.*t1636.*th23_dot.*(-1.0./5.0);
t1726 = t11.*t1637.*th32_dot.*(-1.0./5.0);
t1727 = t12.*t1636.*th33_dot.*(-1.0./5.0);
t1728 = t14.*t1637.*th42_dot.*(-1.0./5.0);
t1729 = t15.*t1636.*th43_dot.*(-1.0./5.0);
t1732 = (t19.*t1644)./5.0;
t1733 = (t20.*t1644)./5.0;
t1734 = (t21.*t1644)./5.0;
t1735 = (t22.*t1644)./5.0;
t1736 = (t23.*t1644)./5.0;
t1737 = (t24.*t1644)./5.0;
t1738 = (t25.*t1644)./5.0;
t1739 = (t26.*t1644)./5.0;
t1740 = (t27.*t1644)./5.0;
t1741 = (t28.*t1644)./5.0;
t1742 = (t29.*t1644)./5.0;
t1743 = (t30.*t1644)./5.0;
t1744 = t144.*t1642;
t1745 = t145.*t1642;
t1746 = t146.*t1642;
t1747 = t147.*t1642;
t1748 = t148.*t1642;
t1749 = t149.*t1642;
t1750 = t150.*t1642;
t1751 = t151.*t1642;
t1752 = t152.*t1642;
t1753 = t153.*t1642;
t1754 = t154.*t1642;
t1755 = t155.*t1642;
t1756 = t144.*t1644;
t1757 = (t19.*t1642)./5.0;
t1758 = t145.*t1644;
t1759 = (t20.*t1642)./5.0;
t1760 = t146.*t1644;
t1761 = (t21.*t1642)./5.0;
t1762 = t147.*t1644;
t1763 = (t22.*t1642)./5.0;
t1764 = t148.*t1644;
t1765 = (t23.*t1642)./5.0;
t1766 = t149.*t1644;
t1767 = (t24.*t1642)./5.0;
t1768 = t150.*t1644;
t1769 = (t25.*t1642)./5.0;
t1770 = t151.*t1644;
t1771 = (t26.*t1642)./5.0;
t1772 = t152.*t1644;
t1773 = (t27.*t1642)./5.0;
t1774 = t153.*t1644;
t1775 = (t28.*t1642)./5.0;
t1776 = t154.*t1644;
t1777 = (t29.*t1642)./5.0;
t1778 = t155.*t1644;
t1779 = (t30.*t1642)./5.0;
t1784 = t4.*t1642.*(-1.0./5.0);
t1785 = t7.*t1642.*(-1.0./5.0);
t1786 = t10.*t1642.*(-1.0./5.0);
t1787 = t13.*t1642.*(-1.0./5.0);
t1788 = t6.*t1644.*(-1.0./5.0);
t1789 = t9.*t1644.*(-1.0./5.0);
t1791 = t12.*t1644.*(-1.0./5.0);
t1794 = t15.*t1644.*(-1.0./5.0);
t1811 = t777.*t1637;
t1812 = t778.*t1636;
t1813 = t780.*t1637;
t1814 = t781.*t1636;
t1815 = t783.*t1637;
t1816 = t784.*t1636;
t1817 = t786.*t1637;
t1818 = t787.*t1636;
t1824 = -t1797;
t1825 = -t1800;
t1826 = t1267+t1521;
t1827 = t1272+t1522;
t1828 = t1277+t1523;
t1829 = t1282+t1524;
t1830 = -t1821;
t1832 = t1254+t1552;
t1834 = t1256+t1554;
t1836 = t1258+t1556;
t1838 = t1260+t1558;
t1843 = t1344+t1559;
t1844 = t1347+t1560;
t1845 = t1350+t1561;
t1846 = t1353+t1562;
t1862 = t44+t68+t105+t113+t118+t296+t1467;
t1869 = t44+t67+t105+t113+t194+t293+t1466;
t1870 = t69+t99+t105+t113+t118+t299+t1468;
t1871 = -t1857;
t1888 = t1379+t1656;
t1889 = t1382+t1657;
t1890 = t1385+t1658;
t1891 = t1388+t1659;
t1892 = t1433+t1685;
t1893 = t1434+t1686;
t1894 = t1435+t1687;
t1895 = t1436+t1688;
t1915 = p2z+t51+t204+t314+t327+t541+t1574;
t1918 = p1z+t51+t204+t314+t433+t538+t1573;
t1919 = p2z+t51+t204+t314+t327+t542+t1585;
t1920 = p3z+t51+t252+t314+t327+t544+t1575;
t1923 = p1z+t51+t204+t314+t433+t539+t1584;
t1924 = p3z+t51+t252+t314+t327+t545+t1586;
t1931 = t1474.*t1849;
t1933 = t1473.*t1854;
t1934 = t1475.*t1855;
t1938 = t1497.*t1863;
t1953 = p3x+t45+t1939;
t1955 = by+t57+t312+t319+t325+t572+t836+t1187+t1389;
t1958 = by+t59+t312+t319+t430+t572+t836+t1190+t1404;
t1959 = by+t58+t319+t325+t402+t836+t840+t1188+t1394;
t1960 = t311+t428+t564+t571+t1291+t1592;
t1961 = t311+t321+t571+t838+t1298+t1594;
t1962 = t320+t329+t826+t835+t1398+t1566;
t1963 = t311+t321+t571+t838+t1305+t1596;
t1964 = t320+t329+t826+t835+t1403+t1568;
t1965 = t311+t428+t564+t571+t1312+t1598;
t1970 = t320+t329+t826+t835+t1396+t1580;
t1972 = t320+t329+t826+t835+t1401+t1581;
t1978 = t320+t434+t835+t965+t1393+t1564;
t1979 = t320+t434+t835+t965+t1408+t1570;
t1984 = t55+t103+t112+t131+t189+t227+t286+t1240+t1620;
t1986 = t56+t103+t112+t115+t131+t286+t310+t1242+t1622;
t1989 = -t1976;
t1991 = t53+t103+t115+t131+t184+t286+t310+t1236+t1616;
t1993 = t54+t103+t131+t184+t189+t227+t286+t1238+t1618;
t1995 = t1469.*t1910;
t1997 = t1472.*t1912;
t1998 = t49+t106+t110+t114+t117+t235+t309+t1287+t1623;
t2001 = -t1987;
t2002 = -t1988;
t2003 = t49+t108+t110+t114+t192+t235+t309+t1308+t1627;
t2006 = t1470.*t1917;
t2007 = (t20.*t1977)./5.0;
t2008 = (t23.*t1977)./5.0;
t2009 = (t26.*t1977)./5.0;
t2010 = (t29.*t1977)./5.0;
t2011 = t49+t107+t114+t117+t179+t309+t315+t1294+t1625;
t2022 = (t21.*t1980)./5.0;
t2023 = (t24.*t1980)./5.0;
t2024 = (t27.*t1980)./5.0;
t2025 = (t30.*t1980)./5.0;
t2026 = (t20.*t1981)./5.0;
t2027 = (t21.*t1982)./5.0;
t2028 = (t23.*t1981)./5.0;
t2029 = (t24.*t1982)./5.0;
t2030 = (t26.*t1981)./5.0;
t2031 = (t27.*t1982)./5.0;
t2032 = (t29.*t1981)./5.0;
t2033 = (t30.*t1982)./5.0;
t2036 = -t2005;
t2037 = -t2012;
t2038 = -t2013;
t2039 = -t2035;
t2040 = t622+t650+t686+t1486+t1669;
t2041 = t625+t653+t689+t1488+t1671;
S_dot = ft_4({bx,bx_dot,by,by_dot,bz_dot,p1x,p1x_dot,p1y,p1y_dot,p2x,p2x_dot,p2y,p2y_dot,p3x,p3x_dot,p3y,p3y_dot,p4x,p4x_dot,p4y,p4y_dot,phi_dot,psi_dot,t10,t1006,t1008,t1010,t1012,t1013,t1014,t1015,t1016,t1017,t1018,t102,t1027,t1028,t103,t1030,t1031,t1033,t1037,t1039,t104,t1040,t1045,t1046,t1047,t1048,t1049,t1051,t1052,t1053,t1054,t1056,t1057,t1058,t1059,t106,t1060,t1061,t1062,t1063,t1064,t1065,t1066,t1067,t1069,t1070,t1071,t1072,t1073,t1074,t1075,t1076,t1077,t1078,t1079,t108,t1081,t1083,t1084,t1086,t1087,t1089,t1091,t1092,t1093,t1094,t1096,t1098,t11,t110,t1105,t1106,t1107,t1108,t1109,t1111,t1113,t1115,t112,t1126,t1127,t1128,t1129,t1131,t1133,t1134,t1135,t1136,t1138,t1139,t114,t115,t1150,t1151,t1159,t1160,t1165,t117,t1171,t1172,t12,t1206,t1207,t1208,t1209,t1210,t1211,t1212,t1213,t1214,t1215,t1216,t1217,t1226,t1227,t1228,t1229,t1230,t1231,t1232,t1233,t1235,t1237,t1239,t1241,t1253,t1255,t1257,t1259,t1261,t1262,t1263,t1264,t1265,t1266,t1271,t1276,t1281,t1288,t1289,t1290,t1292,t1295,t1296,t1299,t13,t1302,t1303,t1306,t1309,t131,t1310,t1311,t1313,t1314,t1315,t1316,t1317,t1318,t1319,t1320,t1323,t1326,t1328,t1331,t1334,t1337,t1345,t1346,t1348,t1349,t1351,t1352,t1354,t1355,t1356,t1357,t1358,t1363,t1364,t1365,t1366,t1367,t1369,t1370,t1371,t1372,t1373,t1374,t1375,t1376,t1390,t1392,t1393,t1395,t14,t1405,t1407,t1408,t1410,t1411,t1419,t1420,t1421,t1422,t1424,t1425,t1427,t1428,t1430,t1431,t1436,t1437,t1438,t1439,t144,t1440,t1441,t1442,t145,t1450,t1451,t1452,t1453,t1454,t1455,t1456,t1457,t1458,t1459,t146,t1460,t1461,t147,t148,t149,t1490,t1492,t1494,t1495,t1496,t1498,t15,t150,t1500,t1502,t1504,t1506,t1507,t1508,t1509,t151,t1510,t1511,t1512,t1513,t1514,t1515,t1516,t1517,t152,t153,t1533,t1534,t154,t1547,t1548,t1549,t155,t1550,t1551,t1552,t1553,t1554,t1555,t1556,t1557,t1558,t1559,t1560,t1561,t1562,t1563,t1564,t1569,t1570,t1571,t1572,t1576,t1577,t1578,t1579,t1582,t1583,t1588,t1589,t1599,t16,t1600,t1601,t1602,t1603,t1604,t1605,t1606,t1607,t1608,t1609,t161,t1610,t1611,t1614,t1615,t1617,t1619,t162,t1621,t1624,t1628,t1629,t163,t1630,t1631,t1632,t1633,t1634,t1635,t1636,t1637,t1639,t164,t1642,t1643,t1644,t1645,t165,t166,t1660,t1661,t1662,t1663,t1664,t1665,t1668,t1670,t1672,t1673,t1674,t1675,t1676,t1677,t1678,t1679,t1680,t1681,t1682,t1683,t1684,t1685,t1686,t1687,t1688,t1689,t1692,t1695,t1698,t17,t1701,t1703,t1704,t1705,t1706,t1707,t1716,t1717,t1718,t1719,t1720,t1721,t1722,t1723,t1724,t1725,t1726,t1727,t1728,t1729,t1730,t1731,t1732,t1733,t1734,t1735,t1736,t1737,t1738,t1739,t1740,t1741,t1742,t1743,t1745,t1746,t1748,t1749,t175,t1751,t1752,t1754,t1755,t1756,t1757,t1758,t1759,t176,t1761,t1762,t1763,t1764,t1765,t1767,t1768,t1769,t177,t1770,t1771,t1773,t1774,t1775,t1776,t1777,t1779,t1784,t1785,t1786,t1787,t1788,t1789,t1791,t1794,t1796,t1798,t1799,t18,t180,t1801,t1802,t1803,t1804,t1805,t1806,t1807,t1808,t1809,t181,t1810,t1811,t1812,t1813,t1814,t1815,t1816,t1817,t1818,t1819,t1820,t1822,t1823,t1824,t1825,t1826,t1827,t1828,t1829,t183,t1830,t184,t1847,t1848,t1851,t1852,t1853,t1856,t1858,t1859,t1860,t1861,t1862,t1864,t1865,t1866,t1867,t1868,t1869,t187,t1870,t1871,t1872,t1873,t1874,t1875,t1876,t1877,t1878,t1879,t188,t1888,t1889,t189,t1890,t1891,t1896,t1897,t1898,t1899,t19,t190,t1900,t1901,t1902,t1903,t1904,t1905,t1906,t1907,t1915,t1916,t1918,t1919,t192,t1920,t1921,t1923,t1924,t1926,t1927,t1929,t1930,t1931,t1932,t1933,t1934,t1938,t1939,t1942,t1943,t1945,t1946,t1948,t1950,t1951,t1952,t1953,t1954,t1955,t1956,t1957,t1958,t1959,t1960,t1961,t1962,t1963,t1964,t1965,t1970,t1972,t1975,t1977,t1980,t1981,t1982,t1984,t1986,t1989,t1991,t1993,t1995,t1996,t1997,t1998,t2,t20,t2001,t2002,t2003,t2005,t2006,t2007,t2008,t2009,t2010,t2011,t2012,t2013,t2022,t2023,t2024,t2025,t2026,t2027,t2028,t2029,t2030,t2031,t2032,t2033,t2035,t2036,t2037,t2038,t2039,t2040,t2041,t2044,t2045,t2050,t2051,t2052,t2057,t2058,t2059,t207,t208,t2080,t2081,t2082,t2083,t209,t2094,t2095,t2096,t2097,t2098,t2099,t21,t210,t2100,t2101,t211,t212,t214,t217,t218,t219,t22,t221,t222,t223,t225,t226,t227,t23,t233,t235,t236,t237,t238,t24,t241,t242,t243,t244,t245,t246,t247,t248,t249,t25,t252,t254,t255,t256,t257,t258,t26,t260,t261,t265,t267,t27,t270,t271,t272,t273,t28,t286,t29,t3,t30,t308,t309,t31,t310,t311,t312,t313,t316,t317,t318,t319,t321,t322,t324,t325,t328,t329,t341,t343,t350,t351,t352,t353,t354,t358,t359,t360,t361,t362,t366,t367,t368,t369,t371,t372,t374,t375,t376,t377,t379,t380,t381,t383,t4,t402,t403,t404,t405,t406,t419,t420,t422,t423,t424,t426,t427,t428,t429,t430,t431,t437,t442,t443,t444,t445,t446,t449,t45,t450,t451,t454,t455,t456,t457,t458,t459,t460,t461,t462,t464,t465,t47,t470,t471,t472,t473,t474,t475,t477,t478,t479,t48,t480,t481,t482,t483,t484,t485,t486,t488,t489,t49,t490,t492,t493,t494,t495,t5,t50,t501,t502,t504,t529,t53,t530,t531,t532,t533,t535,t536,t539,t54,t540,t541,t542,t543,t544,t545,t548,t549,t55,t552,t558,t56,t561,t562,t563,t564,t57,t570,t571,t572,t577,t578,t58,t580,t59,t6,t601,t603,t607,t609,t61,t610,t612,t613,t614,t615,t616,t617,t618,t619,t62,t620,t623,t626,t628,t629,t631,t632,t64,t641,t642,t643,t644,t645,t646,t647,t648,t65,t651,t654,t656,t657,t659,t660,t661,t663,t665,t667,t669,t670,t671,t672,t673,t674,t675,t676,t678,t680,t682,t684,t687,t690,t692,t693,t695,t696,t698,t699,t7,t700,t701,t702,t703,t704,t705,t707,t708,t71,t710,t711,t713,t714,t716,t717,t718,t719,t72,t720,t721,t722,t723,t724,t725,t726,t728,t729,t73,t730,t731,t732,t733,t734,t735,t736,t737,t74,t743,t744,t746,t747,t749,t75,t750,t752,t753,t754,t755,t756,t757,t758,t759,t76,t760,t761,t762,t763,t765,t767,t768,t769,t77,t770,t771,t777,t778,t78,t780,t781,t783,t784,t786,t787,t788,t789,t79,t790,t791,t792,t793,t794,t795,t796,t797,t798,t799,t8,t80,t800,t801,t802,t803,t804,t805,t806,t807,t808,t809,t81,t814,t815,t816,t817,t82,t825,t826,t827,t831,t836,t837,t838,t84,t840,t845,t846,t847,t848,t849,t85,t850,t851,t852,t853,t854,t855,t857,t858,t86,t860,t861,t863,t864,t866,t867,t87,t872,t873,t874,t876,t878,t88,t880,t882,t883,t884,t885,t887,t888,t889,t89,t890,t891,t892,t893,t894,t896,t9,t90,t907,t908,t909,t91,t910,t911,t913,t914,t915,t916,t917,t918,t919,t92,t920,t921,t922,t924,t925,t926,t927,t928,t93,t930,t932,t933,t934,t935,t936,t937,t938,t939,t94,t940,t945,t947,t949,t95,t951,t953,t954,t955,t957,t959,t961,t963,t964,t966,t967,t972,t981,t982,t983,t984,t985,t987,t989,t991,t993,t995,t997,t999,th11_dot,th12_dot,th13_dot,th21_dot,th22_dot,th23_dot,th31_dot,th32_dot,th33_dot,th41_dot,th42_dot,th43_dot,zeta_dot});
end
function S_dot = ft_4(ct)
bx = ct{1};
bx_dot = ct{2};
by = ct{3};
by_dot = ct{4};
bz_dot = ct{5};
p1x = ct{6};
p1x_dot = ct{7};
p1y = ct{8};
p1y_dot = ct{9};
p2x = ct{10};
p2x_dot = ct{11};
p2y = ct{12};
p2y_dot = ct{13};
p3x = ct{14};
p3x_dot = ct{15};
p3y = ct{16};
p3y_dot = ct{17};
p4x = ct{18};
p4x_dot = ct{19};
p4y = ct{20};
p4y_dot = ct{21};
phi_dot = ct{22};
psi_dot = ct{23};
t10 = ct{24};
t1006 = ct{25};
t1008 = ct{26};
t1010 = ct{27};
t1012 = ct{28};
t1013 = ct{29};
t1014 = ct{30};
t1015 = ct{31};
t1016 = ct{32};
t1017 = ct{33};
t1018 = ct{34};
t102 = ct{35};
t1027 = ct{36};
t1028 = ct{37};
t103 = ct{38};
t1030 = ct{39};
t1031 = ct{40};
t1033 = ct{41};
t1037 = ct{42};
t1039 = ct{43};
t104 = ct{44};
t1040 = ct{45};
t1045 = ct{46};
t1046 = ct{47};
t1047 = ct{48};
t1048 = ct{49};
t1049 = ct{50};
t1051 = ct{51};
t1052 = ct{52};
t1053 = ct{53};
t1054 = ct{54};
t1056 = ct{55};
t1057 = ct{56};
t1058 = ct{57};
t1059 = ct{58};
t106 = ct{59};
t1060 = ct{60};
t1061 = ct{61};
t1062 = ct{62};
t1063 = ct{63};
t1064 = ct{64};
t1065 = ct{65};
t1066 = ct{66};
t1067 = ct{67};
t1069 = ct{68};
t1070 = ct{69};
t1071 = ct{70};
t1072 = ct{71};
t1073 = ct{72};
t1074 = ct{73};
t1075 = ct{74};
t1076 = ct{75};
t1077 = ct{76};
t1078 = ct{77};
t1079 = ct{78};
t108 = ct{79};
t1081 = ct{80};
t1083 = ct{81};
t1084 = ct{82};
t1086 = ct{83};
t1087 = ct{84};
t1089 = ct{85};
t1091 = ct{86};
t1092 = ct{87};
t1093 = ct{88};
t1094 = ct{89};
t1096 = ct{90};
t1098 = ct{91};
t11 = ct{92};
t110 = ct{93};
t1105 = ct{94};
t1106 = ct{95};
t1107 = ct{96};
t1108 = ct{97};
t1109 = ct{98};
t1111 = ct{99};
t1113 = ct{100};
t1115 = ct{101};
t112 = ct{102};
t1126 = ct{103};
t1127 = ct{104};
t1128 = ct{105};
t1129 = ct{106};
t1131 = ct{107};
t1133 = ct{108};
t1134 = ct{109};
t1135 = ct{110};
t1136 = ct{111};
t1138 = ct{112};
t1139 = ct{113};
t114 = ct{114};
t115 = ct{115};
t1150 = ct{116};
t1151 = ct{117};
t1159 = ct{118};
t1160 = ct{119};
t1165 = ct{120};
t117 = ct{121};
t1171 = ct{122};
t1172 = ct{123};
t12 = ct{124};
t1206 = ct{125};
t1207 = ct{126};
t1208 = ct{127};
t1209 = ct{128};
t1210 = ct{129};
t1211 = ct{130};
t1212 = ct{131};
t1213 = ct{132};
t1214 = ct{133};
t1215 = ct{134};
t1216 = ct{135};
t1217 = ct{136};
t1226 = ct{137};
t1227 = ct{138};
t1228 = ct{139};
t1229 = ct{140};
t1230 = ct{141};
t1231 = ct{142};
t1232 = ct{143};
t1233 = ct{144};
t1235 = ct{145};
t1237 = ct{146};
t1239 = ct{147};
t1241 = ct{148};
t1253 = ct{149};
t1255 = ct{150};
t1257 = ct{151};
t1259 = ct{152};
t1261 = ct{153};
t1262 = ct{154};
t1263 = ct{155};
t1264 = ct{156};
t1265 = ct{157};
t1266 = ct{158};
t1271 = ct{159};
t1276 = ct{160};
t1281 = ct{161};
t1288 = ct{162};
t1289 = ct{163};
t1290 = ct{164};
t1292 = ct{165};
t1295 = ct{166};
t1296 = ct{167};
t1299 = ct{168};
t13 = ct{169};
t1302 = ct{170};
t1303 = ct{171};
t1306 = ct{172};
t1309 = ct{173};
t131 = ct{174};
t1310 = ct{175};
t1311 = ct{176};
t1313 = ct{177};
t1314 = ct{178};
t1315 = ct{179};
t1316 = ct{180};
t1317 = ct{181};
t1318 = ct{182};
t1319 = ct{183};
t1320 = ct{184};
t1323 = ct{185};
t1326 = ct{186};
t1328 = ct{187};
t1331 = ct{188};
t1334 = ct{189};
t1337 = ct{190};
t1345 = ct{191};
t1346 = ct{192};
t1348 = ct{193};
t1349 = ct{194};
t1351 = ct{195};
t1352 = ct{196};
t1354 = ct{197};
t1355 = ct{198};
t1356 = ct{199};
t1357 = ct{200};
t1358 = ct{201};
t1363 = ct{202};
t1364 = ct{203};
t1365 = ct{204};
t1366 = ct{205};
t1367 = ct{206};
t1369 = ct{207};
t1370 = ct{208};
t1371 = ct{209};
t1372 = ct{210};
t1373 = ct{211};
t1374 = ct{212};
t1375 = ct{213};
t1376 = ct{214};
t1390 = ct{215};
t1392 = ct{216};
t1393 = ct{217};
t1395 = ct{218};
t14 = ct{219};
t1405 = ct{220};
t1407 = ct{221};
t1408 = ct{222};
t1410 = ct{223};
t1411 = ct{224};
t1419 = ct{225};
t1420 = ct{226};
t1421 = ct{227};
t1422 = ct{228};
t1424 = ct{229};
t1425 = ct{230};
t1427 = ct{231};
t1428 = ct{232};
t1430 = ct{233};
t1431 = ct{234};
t1436 = ct{235};
t1437 = ct{236};
t1438 = ct{237};
t1439 = ct{238};
t144 = ct{239};
t1440 = ct{240};
t1441 = ct{241};
t1442 = ct{242};
t145 = ct{243};
t1450 = ct{244};
t1451 = ct{245};
t1452 = ct{246};
t1453 = ct{247};
t1454 = ct{248};
t1455 = ct{249};
t1456 = ct{250};
t1457 = ct{251};
t1458 = ct{252};
t1459 = ct{253};
t146 = ct{254};
t1460 = ct{255};
t1461 = ct{256};
t147 = ct{257};
t148 = ct{258};
t149 = ct{259};
t1490 = ct{260};
t1492 = ct{261};
t1494 = ct{262};
t1495 = ct{263};
t1496 = ct{264};
t1498 = ct{265};
t15 = ct{266};
t150 = ct{267};
t1500 = ct{268};
t1502 = ct{269};
t1504 = ct{270};
t1506 = ct{271};
t1507 = ct{272};
t1508 = ct{273};
t1509 = ct{274};
t151 = ct{275};
t1510 = ct{276};
t1511 = ct{277};
t1512 = ct{278};
t1513 = ct{279};
t1514 = ct{280};
t1515 = ct{281};
t1516 = ct{282};
t1517 = ct{283};
t152 = ct{284};
t153 = ct{285};
t1533 = ct{286};
t1534 = ct{287};
t154 = ct{288};
t1547 = ct{289};
t1548 = ct{290};
t1549 = ct{291};
t155 = ct{292};
t1550 = ct{293};
t1551 = ct{294};
t1552 = ct{295};
t1553 = ct{296};
t1554 = ct{297};
t1555 = ct{298};
t1556 = ct{299};
t1557 = ct{300};
t1558 = ct{301};
t1559 = ct{302};
t1560 = ct{303};
t1561 = ct{304};
t1562 = ct{305};
t1563 = ct{306};
t1564 = ct{307};
t1569 = ct{308};
t1570 = ct{309};
t1571 = ct{310};
t1572 = ct{311};
t1576 = ct{312};
t1577 = ct{313};
t1578 = ct{314};
t1579 = ct{315};
t1582 = ct{316};
t1583 = ct{317};
t1588 = ct{318};
t1589 = ct{319};
t1599 = ct{320};
t16 = ct{321};
t1600 = ct{322};
t1601 = ct{323};
t1602 = ct{324};
t1603 = ct{325};
t1604 = ct{326};
t1605 = ct{327};
t1606 = ct{328};
t1607 = ct{329};
t1608 = ct{330};
t1609 = ct{331};
t161 = ct{332};
t1610 = ct{333};
t1611 = ct{334};
t1614 = ct{335};
t1615 = ct{336};
t1617 = ct{337};
t1619 = ct{338};
t162 = ct{339};
t1621 = ct{340};
t1624 = ct{341};
t1628 = ct{342};
t1629 = ct{343};
t163 = ct{344};
t1630 = ct{345};
t1631 = ct{346};
t1632 = ct{347};
t1633 = ct{348};
t1634 = ct{349};
t1635 = ct{350};
t1636 = ct{351};
t1637 = ct{352};
t1639 = ct{353};
t164 = ct{354};
t1642 = ct{355};
t1643 = ct{356};
t1644 = ct{357};
t1645 = ct{358};
t165 = ct{359};
t166 = ct{360};
t1660 = ct{361};
t1661 = ct{362};
t1662 = ct{363};
t1663 = ct{364};
t1664 = ct{365};
t1665 = ct{366};
t1668 = ct{367};
t1670 = ct{368};
t1672 = ct{369};
t1673 = ct{370};
t1674 = ct{371};
t1675 = ct{372};
t1676 = ct{373};
t1677 = ct{374};
t1678 = ct{375};
t1679 = ct{376};
t1680 = ct{377};
t1681 = ct{378};
t1682 = ct{379};
t1683 = ct{380};
t1684 = ct{381};
t1685 = ct{382};
t1686 = ct{383};
t1687 = ct{384};
t1688 = ct{385};
t1689 = ct{386};
t1692 = ct{387};
t1695 = ct{388};
t1698 = ct{389};
t17 = ct{390};
t1701 = ct{391};
t1703 = ct{392};
t1704 = ct{393};
t1705 = ct{394};
t1706 = ct{395};
t1707 = ct{396};
t1716 = ct{397};
t1717 = ct{398};
t1718 = ct{399};
t1719 = ct{400};
t1720 = ct{401};
t1721 = ct{402};
t1722 = ct{403};
t1723 = ct{404};
t1724 = ct{405};
t1725 = ct{406};
t1726 = ct{407};
t1727 = ct{408};
t1728 = ct{409};
t1729 = ct{410};
t1730 = ct{411};
t1731 = ct{412};
t1732 = ct{413};
t1733 = ct{414};
t1734 = ct{415};
t1735 = ct{416};
t1736 = ct{417};
t1737 = ct{418};
t1738 = ct{419};
t1739 = ct{420};
t1740 = ct{421};
t1741 = ct{422};
t1742 = ct{423};
t1743 = ct{424};
t1745 = ct{425};
t1746 = ct{426};
t1748 = ct{427};
t1749 = ct{428};
t175 = ct{429};
t1751 = ct{430};
t1752 = ct{431};
t1754 = ct{432};
t1755 = ct{433};
t1756 = ct{434};
t1757 = ct{435};
t1758 = ct{436};
t1759 = ct{437};
t176 = ct{438};
t1761 = ct{439};
t1762 = ct{440};
t1763 = ct{441};
t1764 = ct{442};
t1765 = ct{443};
t1767 = ct{444};
t1768 = ct{445};
t1769 = ct{446};
t177 = ct{447};
t1770 = ct{448};
t1771 = ct{449};
t1773 = ct{450};
t1774 = ct{451};
t1775 = ct{452};
t1776 = ct{453};
t1777 = ct{454};
t1779 = ct{455};
t1784 = ct{456};
t1785 = ct{457};
t1786 = ct{458};
t1787 = ct{459};
t1788 = ct{460};
t1789 = ct{461};
t1791 = ct{462};
t1794 = ct{463};
t1796 = ct{464};
t1798 = ct{465};
t1799 = ct{466};
t18 = ct{467};
t180 = ct{468};
t1801 = ct{469};
t1802 = ct{470};
t1803 = ct{471};
t1804 = ct{472};
t1805 = ct{473};
t1806 = ct{474};
t1807 = ct{475};
t1808 = ct{476};
t1809 = ct{477};
t181 = ct{478};
t1810 = ct{479};
t1811 = ct{480};
t1812 = ct{481};
t1813 = ct{482};
t1814 = ct{483};
t1815 = ct{484};
t1816 = ct{485};
t1817 = ct{486};
t1818 = ct{487};
t1819 = ct{488};
t1820 = ct{489};
t1822 = ct{490};
t1823 = ct{491};
t1824 = ct{492};
t1825 = ct{493};
t1826 = ct{494};
t1827 = ct{495};
t1828 = ct{496};
t1829 = ct{497};
t183 = ct{498};
t1830 = ct{499};
t184 = ct{500};
t1847 = ct{501};
t1848 = ct{502};
t1851 = ct{503};
t1852 = ct{504};
t1853 = ct{505};
t1856 = ct{506};
t1858 = ct{507};
t1859 = ct{508};
t1860 = ct{509};
t1861 = ct{510};
t1862 = ct{511};
t1864 = ct{512};
t1865 = ct{513};
t1866 = ct{514};
t1867 = ct{515};
t1868 = ct{516};
t1869 = ct{517};
t187 = ct{518};
t1870 = ct{519};
t1871 = ct{520};
t1872 = ct{521};
t1873 = ct{522};
t1874 = ct{523};
t1875 = ct{524};
t1876 = ct{525};
t1877 = ct{526};
t1878 = ct{527};
t1879 = ct{528};
t188 = ct{529};
t1888 = ct{530};
t1889 = ct{531};
t189 = ct{532};
t1890 = ct{533};
t1891 = ct{534};
t1896 = ct{535};
t1897 = ct{536};
t1898 = ct{537};
t1899 = ct{538};
t19 = ct{539};
t190 = ct{540};
t1900 = ct{541};
t1901 = ct{542};
t1902 = ct{543};
t1903 = ct{544};
t1904 = ct{545};
t1905 = ct{546};
t1906 = ct{547};
t1907 = ct{548};
t1915 = ct{549};
t1916 = ct{550};
t1918 = ct{551};
t1919 = ct{552};
t192 = ct{553};
t1920 = ct{554};
t1921 = ct{555};
t1923 = ct{556};
t1924 = ct{557};
t1926 = ct{558};
t1927 = ct{559};
t1929 = ct{560};
t1930 = ct{561};
t1931 = ct{562};
t1932 = ct{563};
t1933 = ct{564};
t1934 = ct{565};
t1938 = ct{566};
t1939 = ct{567};
t1942 = ct{568};
t1943 = ct{569};
t1945 = ct{570};
t1946 = ct{571};
t1948 = ct{572};
t1950 = ct{573};
t1951 = ct{574};
t1952 = ct{575};
t1953 = ct{576};
t1954 = ct{577};
t1955 = ct{578};
t1956 = ct{579};
t1957 = ct{580};
t1958 = ct{581};
t1959 = ct{582};
t1960 = ct{583};
t1961 = ct{584};
t1962 = ct{585};
t1963 = ct{586};
t1964 = ct{587};
t1965 = ct{588};
t1970 = ct{589};
t1972 = ct{590};
t1975 = ct{591};
t1977 = ct{592};
t1980 = ct{593};
t1981 = ct{594};
t1982 = ct{595};
t1984 = ct{596};
t1986 = ct{597};
t1989 = ct{598};
t1991 = ct{599};
t1993 = ct{600};
t1995 = ct{601};
t1996 = ct{602};
t1997 = ct{603};
t1998 = ct{604};
t2 = ct{605};
t20 = ct{606};
t2001 = ct{607};
t2002 = ct{608};
t2003 = ct{609};
t2005 = ct{610};
t2006 = ct{611};
t2007 = ct{612};
t2008 = ct{613};
t2009 = ct{614};
t2010 = ct{615};
t2011 = ct{616};
t2012 = ct{617};
t2013 = ct{618};
t2022 = ct{619};
t2023 = ct{620};
t2024 = ct{621};
t2025 = ct{622};
t2026 = ct{623};
t2027 = ct{624};
t2028 = ct{625};
t2029 = ct{626};
t2030 = ct{627};
t2031 = ct{628};
t2032 = ct{629};
t2033 = ct{630};
t2035 = ct{631};
t2036 = ct{632};
t2037 = ct{633};
t2038 = ct{634};
t2039 = ct{635};
t2040 = ct{636};
t2041 = ct{637};
t2044 = ct{638};
t2045 = ct{639};
t2050 = ct{640};
t2051 = ct{641};
t2052 = ct{642};
t2057 = ct{643};
t2058 = ct{644};
t2059 = ct{645};
t207 = ct{646};
t208 = ct{647};
t2080 = ct{648};
t2081 = ct{649};
t2082 = ct{650};
t2083 = ct{651};
t209 = ct{652};
t2094 = ct{653};
t2095 = ct{654};
t2096 = ct{655};
t2097 = ct{656};
t2098 = ct{657};
t2099 = ct{658};
t21 = ct{659};
t210 = ct{660};
t2100 = ct{661};
t2101 = ct{662};
t211 = ct{663};
t212 = ct{664};
t214 = ct{665};
t217 = ct{666};
t218 = ct{667};
t219 = ct{668};
t22 = ct{669};
t221 = ct{670};
t222 = ct{671};
t223 = ct{672};
t225 = ct{673};
t226 = ct{674};
t227 = ct{675};
t23 = ct{676};
t233 = ct{677};
t235 = ct{678};
t236 = ct{679};
t237 = ct{680};
t238 = ct{681};
t24 = ct{682};
t241 = ct{683};
t242 = ct{684};
t243 = ct{685};
t244 = ct{686};
t245 = ct{687};
t246 = ct{688};
t247 = ct{689};
t248 = ct{690};
t249 = ct{691};
t25 = ct{692};
t252 = ct{693};
t254 = ct{694};
t255 = ct{695};
t256 = ct{696};
t257 = ct{697};
t258 = ct{698};
t26 = ct{699};
t260 = ct{700};
t261 = ct{701};
t265 = ct{702};
t267 = ct{703};
t27 = ct{704};
t270 = ct{705};
t271 = ct{706};
t272 = ct{707};
t273 = ct{708};
t28 = ct{709};
t286 = ct{710};
t29 = ct{711};
t3 = ct{712};
t30 = ct{713};
t308 = ct{714};
t309 = ct{715};
t31 = ct{716};
t310 = ct{717};
t311 = ct{718};
t312 = ct{719};
t313 = ct{720};
t316 = ct{721};
t317 = ct{722};
t318 = ct{723};
t319 = ct{724};
t321 = ct{725};
t322 = ct{726};
t324 = ct{727};
t325 = ct{728};
t328 = ct{729};
t329 = ct{730};
t341 = ct{731};
t343 = ct{732};
t350 = ct{733};
t351 = ct{734};
t352 = ct{735};
t353 = ct{736};
t354 = ct{737};
t358 = ct{738};
t359 = ct{739};
t360 = ct{740};
t361 = ct{741};
t362 = ct{742};
t366 = ct{743};
t367 = ct{744};
t368 = ct{745};
t369 = ct{746};
t371 = ct{747};
t372 = ct{748};
t374 = ct{749};
t375 = ct{750};
t376 = ct{751};
t377 = ct{752};
t379 = ct{753};
t380 = ct{754};
t381 = ct{755};
t383 = ct{756};
t4 = ct{757};
t402 = ct{758};
t403 = ct{759};
t404 = ct{760};
t405 = ct{761};
t406 = ct{762};
t419 = ct{763};
t420 = ct{764};
t422 = ct{765};
t423 = ct{766};
t424 = ct{767};
t426 = ct{768};
t427 = ct{769};
t428 = ct{770};
t429 = ct{771};
t430 = ct{772};
t431 = ct{773};
t437 = ct{774};
t442 = ct{775};
t443 = ct{776};
t444 = ct{777};
t445 = ct{778};
t446 = ct{779};
t449 = ct{780};
t45 = ct{781};
t450 = ct{782};
t451 = ct{783};
t454 = ct{784};
t455 = ct{785};
t456 = ct{786};
t457 = ct{787};
t458 = ct{788};
t459 = ct{789};
t460 = ct{790};
t461 = ct{791};
t462 = ct{792};
t464 = ct{793};
t465 = ct{794};
t47 = ct{795};
t470 = ct{796};
t471 = ct{797};
t472 = ct{798};
t473 = ct{799};
t474 = ct{800};
t475 = ct{801};
t477 = ct{802};
t478 = ct{803};
t479 = ct{804};
t48 = ct{805};
t480 = ct{806};
t481 = ct{807};
t482 = ct{808};
t483 = ct{809};
t484 = ct{810};
t485 = ct{811};
t486 = ct{812};
t488 = ct{813};
t489 = ct{814};
t49 = ct{815};
t490 = ct{816};
t492 = ct{817};
t493 = ct{818};
t494 = ct{819};
t495 = ct{820};
t5 = ct{821};
t50 = ct{822};
t501 = ct{823};
t502 = ct{824};
t504 = ct{825};
t529 = ct{826};
t53 = ct{827};
t530 = ct{828};
t531 = ct{829};
t532 = ct{830};
t533 = ct{831};
t535 = ct{832};
t536 = ct{833};
t539 = ct{834};
t54 = ct{835};
t540 = ct{836};
t541 = ct{837};
t542 = ct{838};
t543 = ct{839};
t544 = ct{840};
t545 = ct{841};
t548 = ct{842};
t549 = ct{843};
t55 = ct{844};
t552 = ct{845};
t558 = ct{846};
t56 = ct{847};
t561 = ct{848};
t562 = ct{849};
t563 = ct{850};
t564 = ct{851};
t57 = ct{852};
t570 = ct{853};
t571 = ct{854};
t572 = ct{855};
t577 = ct{856};
t578 = ct{857};
t58 = ct{858};
t580 = ct{859};
t59 = ct{860};
t6 = ct{861};
t601 = ct{862};
t603 = ct{863};
t607 = ct{864};
t609 = ct{865};
t61 = ct{866};
t610 = ct{867};
t612 = ct{868};
t613 = ct{869};
t614 = ct{870};
t615 = ct{871};
t616 = ct{872};
t617 = ct{873};
t618 = ct{874};
t619 = ct{875};
t62 = ct{876};
t620 = ct{877};
t623 = ct{878};
t626 = ct{879};
t628 = ct{880};
t629 = ct{881};
t631 = ct{882};
t632 = ct{883};
t64 = ct{884};
t641 = ct{885};
t642 = ct{886};
t643 = ct{887};
t644 = ct{888};
t645 = ct{889};
t646 = ct{890};
t647 = ct{891};
t648 = ct{892};
t65 = ct{893};
t651 = ct{894};
t654 = ct{895};
t656 = ct{896};
t657 = ct{897};
t659 = ct{898};
t660 = ct{899};
t661 = ct{900};
t663 = ct{901};
t665 = ct{902};
t667 = ct{903};
t669 = ct{904};
t670 = ct{905};
t671 = ct{906};
t672 = ct{907};
t673 = ct{908};
t674 = ct{909};
t675 = ct{910};
t676 = ct{911};
t678 = ct{912};
t680 = ct{913};
t682 = ct{914};
t684 = ct{915};
t687 = ct{916};
t690 = ct{917};
t692 = ct{918};
t693 = ct{919};
t695 = ct{920};
t696 = ct{921};
t698 = ct{922};
t699 = ct{923};
t7 = ct{924};
t700 = ct{925};
t701 = ct{926};
t702 = ct{927};
t703 = ct{928};
t704 = ct{929};
t705 = ct{930};
t707 = ct{931};
t708 = ct{932};
t71 = ct{933};
t710 = ct{934};
t711 = ct{935};
t713 = ct{936};
t714 = ct{937};
t716 = ct{938};
t717 = ct{939};
t718 = ct{940};
t719 = ct{941};
t72 = ct{942};
t720 = ct{943};
t721 = ct{944};
t722 = ct{945};
t723 = ct{946};
t724 = ct{947};
t725 = ct{948};
t726 = ct{949};
t728 = ct{950};
t729 = ct{951};
t73 = ct{952};
t730 = ct{953};
t731 = ct{954};
t732 = ct{955};
t733 = ct{956};
t734 = ct{957};
t735 = ct{958};
t736 = ct{959};
t737 = ct{960};
t74 = ct{961};
t743 = ct{962};
t744 = ct{963};
t746 = ct{964};
t747 = ct{965};
t749 = ct{966};
t75 = ct{967};
t750 = ct{968};
t752 = ct{969};
t753 = ct{970};
t754 = ct{971};
t755 = ct{972};
t756 = ct{973};
t757 = ct{974};
t758 = ct{975};
t759 = ct{976};
t76 = ct{977};
t760 = ct{978};
t761 = ct{979};
t762 = ct{980};
t763 = ct{981};
t765 = ct{982};
t767 = ct{983};
t768 = ct{984};
t769 = ct{985};
t77 = ct{986};
t770 = ct{987};
t771 = ct{988};
t777 = ct{989};
t778 = ct{990};
t78 = ct{991};
t780 = ct{992};
t781 = ct{993};
t783 = ct{994};
t784 = ct{995};
t786 = ct{996};
t787 = ct{997};
t788 = ct{998};
t789 = ct{999};
t79 = ct{1000};
t790 = ct{1001};
t791 = ct{1002};
t792 = ct{1003};
t793 = ct{1004};
t794 = ct{1005};
t795 = ct{1006};
t796 = ct{1007};
t797 = ct{1008};
t798 = ct{1009};
t799 = ct{1010};
t8 = ct{1011};
t80 = ct{1012};
t800 = ct{1013};
t801 = ct{1014};
t802 = ct{1015};
t803 = ct{1016};
t804 = ct{1017};
t805 = ct{1018};
t806 = ct{1019};
t807 = ct{1020};
t808 = ct{1021};
t809 = ct{1022};
t81 = ct{1023};
t814 = ct{1024};
t815 = ct{1025};
t816 = ct{1026};
t817 = ct{1027};
t82 = ct{1028};
t825 = ct{1029};
t826 = ct{1030};
t827 = ct{1031};
t831 = ct{1032};
t836 = ct{1033};
t837 = ct{1034};
t838 = ct{1035};
t84 = ct{1036};
t840 = ct{1037};
t845 = ct{1038};
t846 = ct{1039};
t847 = ct{1040};
t848 = ct{1041};
t849 = ct{1042};
t85 = ct{1043};
t850 = ct{1044};
t851 = ct{1045};
t852 = ct{1046};
t853 = ct{1047};
t854 = ct{1048};
t855 = ct{1049};
t857 = ct{1050};
t858 = ct{1051};
t86 = ct{1052};
t860 = ct{1053};
t861 = ct{1054};
t863 = ct{1055};
t864 = ct{1056};
t866 = ct{1057};
t867 = ct{1058};
t87 = ct{1059};
t872 = ct{1060};
t873 = ct{1061};
t874 = ct{1062};
t876 = ct{1063};
t878 = ct{1064};
t88 = ct{1065};
t880 = ct{1066};
t882 = ct{1067};
t883 = ct{1068};
t884 = ct{1069};
t885 = ct{1070};
t887 = ct{1071};
t888 = ct{1072};
t889 = ct{1073};
t89 = ct{1074};
t890 = ct{1075};
t891 = ct{1076};
t892 = ct{1077};
t893 = ct{1078};
t894 = ct{1079};
t896 = ct{1080};
t9 = ct{1081};
t90 = ct{1082};
t907 = ct{1083};
t908 = ct{1084};
t909 = ct{1085};
t91 = ct{1086};
t910 = ct{1087};
t911 = ct{1088};
t913 = ct{1089};
t914 = ct{1090};
t915 = ct{1091};
t916 = ct{1092};
t917 = ct{1093};
t918 = ct{1094};
t919 = ct{1095};
t92 = ct{1096};
t920 = ct{1097};
t921 = ct{1098};
t922 = ct{1099};
t924 = ct{1100};
t925 = ct{1101};
t926 = ct{1102};
t927 = ct{1103};
t928 = ct{1104};
t93 = ct{1105};
t930 = ct{1106};
t932 = ct{1107};
t933 = ct{1108};
t934 = ct{1109};
t935 = ct{1110};
t936 = ct{1111};
t937 = ct{1112};
t938 = ct{1113};
t939 = ct{1114};
t94 = ct{1115};
t940 = ct{1116};
t945 = ct{1117};
t947 = ct{1118};
t949 = ct{1119};
t95 = ct{1120};
t951 = ct{1121};
t953 = ct{1122};
t954 = ct{1123};
t955 = ct{1124};
t957 = ct{1125};
t959 = ct{1126};
t961 = ct{1127};
t963 = ct{1128};
t964 = ct{1129};
t966 = ct{1130};
t967 = ct{1131};
t972 = ct{1132};
t981 = ct{1133};
t982 = ct{1134};
t983 = ct{1135};
t984 = ct{1136};
t985 = ct{1137};
t987 = ct{1138};
t989 = ct{1139};
t991 = ct{1140};
t993 = ct{1141};
t995 = ct{1142};
t997 = ct{1143};
t999 = ct{1144};
th11_dot = ct{1145};
th12_dot = ct{1146};
th13_dot = ct{1147};
th21_dot = ct{1148};
th22_dot = ct{1149};
th23_dot = ct{1150};
th31_dot = ct{1151};
th32_dot = ct{1152};
th33_dot = ct{1153};
th41_dot = ct{1154};
th42_dot = ct{1155};
th43_dot = ct{1156};
zeta_dot = ct{1157};
t2042 = t628+t656+t692+t1490+t1673;
t2043 = t631+t659+t695+t1492+t1675;
t2053 = t777.*t1977;
t2054 = t780.*t1977;
t2055 = t783.*t1977;
t2056 = t786.*t1977;
t2060 = t778.*t1980;
t2061 = t781.*t1980;
t2062 = t784.*t1980;
t2063 = t787.*t1980;
t2064 = t777.*t1981;
t2065 = t778.*t1982;
t2066 = t780.*t1981;
t2067 = t781.*t1982;
t2068 = t783.*t1981;
t2069 = t784.*t1982;
t2070 = t786.*t1981;
t2071 = t787.*t1982;
t2092 = t312+t319+t325+t572+t836+t1390+t1819;
t2104 = t312+t319+t430+t572+t836+t1405+t1822;
t2106 = t1517.*t1954;
t2107 = t319+t325+t402+t836+t840+t1395+t1820;
t2109 = t1514.*t1956;
t2110 = t1515.*t1957;
t2124 = -t2044.*(t211./5.0-t248);
t2125 = -t2045.*(t212./5.0-t249);
t2135 = -t2058.*(t209./5.0-t246);
t2136 = -t2059.*(t210./5.0-t247);
t2137 = -t2080.*(t211./5.0-t248);
t2138 = -t2081.*(t212./5.0-t249);
t2139 = -t2082.*(t209./5.0-t246);
t2140 = -t2083.*(t210./5.0-t247);
t2141 = t2080.*(t211./5.0-t248);
t2142 = t2081.*(t212./5.0-t249);
t2143 = t2082.*(t209./5.0-t246);
t2144 = t2083.*(t210./5.0-t247);
t2164 = bz_dot+t75+t271+t473+t484+t495+t713+t729+t749+t863+t1502+t1805;
t2165 = bz_dot+t76+t271+t451+t473+t484+t716+t752+t803+t866+t1504+t1807;
t2166 = bz_dot+t73+t372+t451+t473+t484+t707+t743+t803+t857+t1498+t1801;
t2167 = bz_dot+t74+t372+t473+t484+t495+t710+t729+t746+t860+t1500+t1803;
t2168 = bz_dot+t75+t271+t473+t484+t495+t714+t729+t750+t864+t1512+t1806;
t2169 = bz_dot+t76+t271+t451+t473+t484+t717+t753+t803+t867+t1513+t1808;
t2170 = bz_dot+t73+t372+t451+t473+t484+t708+t744+t803+t858+t1510+t1802;
t2171 = bz_dot+t74+t372+t473+t484+t495+t711+t729+t747+t861+t1511+t1804;
t2201 = t1942.*t2096;
t2202 = t1943.*t2097;
t2203 = t1945.*t2100;
t2204 = t1946.*t2101;
t2207 = t1948.*t2098;
t2208 = t1950.*t2094;
t2209 = t1951.*t2095;
t2212 = t1952.*t2099;
t2248 = p3x_dot+t47+t454+t459+t470+t480+t481+t618+t645+t665+t671+t675+t682+t699+t872+t893+t910+t983+t989+t1060+t1064+t1076+t1107+t1113;
t2249 = p4x_dot+t47+t442+t454+t459+t470+t481+t620+t647+t667+t672+t676+t684+t790+t872+t932+t984+t991+t1048+t1058+t1060+t1064+t1108+t1115;
t2252 = p3y_dot+t50+t341+t477+t492+t700+t720+t724+t735+t758+t761+t850+t878+t884+t887+t909+t915+t922+t928+t997+t1010+t1017+t1077+t1128;
t2253 = p2x_dot+t47+t454+t459+t480+t616+t643+t663+t670+t674+t680+t699+t769+t793+t872+t893+t910+t982+t987+t1060+t1064+t1076+t1106+t1111;
t2256 = p4y_dot+t50+t341+t457+t460+t477+t492+t700+t721+t725+t737+t851+t880+t885+t887+t909+t999+t1012+t1018+t1061+t1067+t1073+t1077+t1129;
t2257 = p1x_dot+t47+t442+t454+t459+t614+t641+t661+t669+t673+t678+t769+t790+t793+t872+t932+t981+t985+t1048+t1058+t1060+t1064+t1105+t1109;
t2258 = p2y_dot+t50+t477+t700+t719+t723+t733+t758+t761+t801+t849+t876+t883+t887+t909+t915+t922+t928+t930+t995+t1008+t1016+t1077+t1127;
t2259 = p1y_dot+t50+t457+t460+t477+t700+t718+t722+t731+t801+t848+t874+t882+t887+t909+t930+t993+t1006+t1015+t1061+t1067+t1073+t1077+t1126;
t1690 = t1677.*th12_dot;
t1691 = t1678.*th13_dot;
t1693 = t1679.*th22_dot;
t1694 = t1680.*th23_dot;
t1696 = t1681.*th32_dot;
t1697 = t1682.*th33_dot;
t1699 = t1683.*th42_dot;
t1700 = t1684.*th43_dot;
t1780 = -t1733;
t1781 = -t1734;
t1782 = -t1742;
t1783 = -t1743;
t1790 = -t1771;
t1792 = -t1773;
t1793 = -t1777;
t1795 = -t1779;
t1831 = t1253+t1551;
t1833 = t1255+t1553;
t1835 = t1257+t1555;
t1837 = t1259+t1557;
t1880 = t1345+t1677;
t1881 = t1346+t1678;
t1882 = t1348+t1679;
t1883 = t1349+t1680;
t1884 = t1351+t1681;
t1885 = t1352+t1682;
t1886 = t1354+t1683;
t1887 = t1355+t1684;
t1935 = -t1931;
t1936 = -t1933;
t1937 = t1495.*t1862;
t1940 = t1494.*t1869;
t1941 = t1496.*t1870;
t1949 = t312+t325+t426+t562+t572+t1261+t1439;
t1967 = t311+t428+t564+t571+t1288+t1602;
t1968 = t329+t427+t561+t826+t1437+t1563;
t1969 = t311+t321+t571+t838+t1295+t1603;
t1971 = t311+t321+t571+t838+t1302+t1604;
t1973 = t311+t428+t564+t571+t1309+t1605;
t1974 = t329+t427+t561+t826+t1442+t1569;
t1983 = t55+t103+t112+t131+t189+t227+t286+t1239+t1619;
t1985 = t56+t103+t112+t115+t131+t286+t310+t1241+t1621;
t1990 = t53+t103+t115+t131+t184+t286+t310+t1235+t1615;
t1992 = t54+t103+t131+t184+t189+t227+t286+t1237+t1617;
t1994 = t62+t104+t110+t117+t188+t226+t235+t1358+t1589;
t1999 = t49+t106+t110+t114+t117+t235+t309+t1290+t1624;
t2000 = t61+t104+t110+t188+t192+t226+t235+t1356+t1588;
t2004 = t49+t108+t110+t114+t192+t235+t309+t1311+t1628;
t2014 = t702+t730+t852+t1328+t1784;
t2015 = t703+t732+t853+t1331+t1785;
t2016 = t704+t734+t854+t1334+t1786;
t2017 = t705+t736+t855+t1337+t1787;
t2018 = t613+t642+t937+t1421+t1756;
t2019 = t615+t644+t938+t1424+t1762;
t2020 = t617+t646+t939+t1427+t1768;
t2021 = t619+t648+t940+t1430+t1774;
t2034 = t62+t104+t110+t117+t188+t226+t235+t1357+t1639;
t2046 = t623+t651+t687+t1506+t1670;
t2047 = t626+t654+t690+t1507+t1672;
t2048 = t629+t657+t693+t1508+t1674;
t2049 = t632+t660+t696+t1509+t1676;
t2072 = -t2053;
t2073 = -t2054;
t2074 = -t2060;
t2075 = -t2061;
t2076 = -t2065;
t2077 = -t2066;
t2078 = -t2068;
t2079 = -t2071;
t2084 = t313+t328+t429+t563+t825+t1303+t1815;
t2085 = t313+t328+t429+t563+t825+t1306+t1816;
t2086 = t313+t322+t328+t825+t837+t1310+t1817;
t2087 = t313+t322+t328+t825+t837+t1313+t1818;
t2088 = t322+t328+t423+t825+t837+t1289+t1811;
t2089 = t322+t328+t423+t825+t837+t1292+t1812;
t2090 = t328+t423+t429+t563+t825+t1296+t1813;
t2091 = t328+t423+t429+t563+t825+t1299+t1814;
t2093 = t312+t325+t426+t562+t572+t1441+t1799;
t2102 = t312+t319+t325+t572+t836+t1392+t1824;
t2103 = t312+t426+t430+t562+t572+t1438+t1798;
t2105 = t1516.*t1953;
t2108 = t312+t319+t430+t572+t836+t1407+t1825;
t2111 = t312+t325+t426+t562+t572+t1440+t1830;
t2121 = -t1955.*(t403-(t4.*t1159)./5.0);
t2122 = by+t57+t2092;
t2126 = -t1958.*(t406-(t13.*t1159)./5.0);
t2129 = by+t59+t2104;
t2130 = -t1959.*(t404-(t7.*t1159)./5.0);
t2131 = by+t58+t2107;
t2146 = -t1984.*(t1231-t1556);
t2148 = -t1986.*(t1233-t1558);
t2151 = -t1991.*(t1227-t1552);
t2153 = -t1993.*(t1229-t1554);
t2158 = t1991.*(t1227-t1552);
t2159 = -t1998.*(t1266-t1559);
t2161 = -t2003.*(t1281-t1562);
t2162 = -t2011.*(t1271-t1560);
t2172 = t1915.*t2041;
t2173 = t1916.*t2043;
t2174 = t1918.*t2040;
t2175 = t1920.*t2042;
